simulink library "outp"  (R2021b)
settings: Solver=VariableStepAuto  StartTime=0.0  StopTime=10.0  RelTol=1e-3
undefined symbols (not defined in the file or in its folder): ENUM_PMMMODE_CHARGE, ENUM_PMMMODE_IDLE, ENUM_PMMMODE_INITIALIZE, ENUM_PMMMODE_POWERDOWN, ENUM_PMMMODE_SLEEP, Left, outp, slcm, TRUE
libraries: FVT_lib x1097, hcu_lib x4, simulink x1
(part 2 of 11)

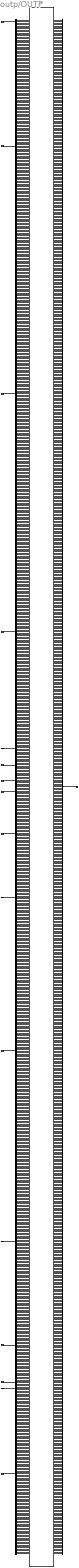
== system outp/OUTP ==
  BACC_outputs : Inport  OutDataTypeStr=Bus: BACC_outputs
  BAPM_outputs : Inport  Port=2  OutDataTypeStr=Bus: BAPM_outputs
  BBCM_outputs : Inport  Port=3  OutDataTypeStr=Bus: BBCM_outputs
  BDDM_outputs : Inport  Port=4  OutDataTypeStr=Bus: BDDM_outputs
  BDHP_outputs : Inport  Port=5  OutDataTypeStr=Bus: BDHP_outputs
  BDKC_outputs : Inport  Port=6  OutDataTypeStr=Bus: BDKC_outputs
  BDSC_outputs : Inport  Port=7  OutDataTypeStr=Bus: BDSC_outputs
  BNMM_outputs : Inport  Port=8  OutDataTypeStr=Bus: BNMM_outputs
  BPMM_outputs : Inport  Port=9  OutDataTypeStr=Bus: BPMM_outputs
  BSYS_outputs : Inport  Port=10  OutDataTypeStr=Bus: BSYS_outputs
  BTHC_outputs : Inport  Port=11  OutDataTypeStr=Bus: BTHC_outputs
  BTPM_outputs : Inport  Port=12  OutDataTypeStr=Bus: BTPM_outputs
  BTQD_outputs : Inport  Port=13  OutDataTypeStr=Bus: BTQD_outputs
  BTQR_outputs : Inport  Port=14  OutDataTypeStr=Bus: BTQR_outputs
  BV2L_outputs : Inport  Port=15  OutDataTypeStr=Bus: BV2L_outputs
  BVMC_outputs : Inport  Port=16  OutDataTypeStr=Bus: BVMC_outputs
  trig_OUTP : TriggerPort  TriggerType=function-call  VariantControl=(inherit)
  bus_creator : BusCreator  Inputs=1097
  bus_selector1 : BusSelector  OutputSignals=VACC_HVTHCMSysAvail_enum,VACC_LVBattVoltSta_enum,VACC_VehHVPwrAvail4THCM_W
  bus_selector10 : BusSelector  OutputSignals=VSYS_HWVer1_cnt,VSYS_HWVer2_cnt,VSYS_HWVer3_cnt,VSYS_CarModel1_cnt,VSYS_CarModel2_cnt,VSYS_CarModel3_cnt,VSYS_ECU1_cnt,VSYS_ECU2_cnt,VSYS_Major1_cnt,VSYS_Major2_cnt,VSYS_Minor1_cnt,VSYS_Minor2_cnt,VSYS_Patch1_cnt,VSYS_Patch2_cnt,VSYS_Country1_cnt,VSYS_Country2_cnt,VSYS_Variation_cnt,VSYS_Dash1_cnt,VSYS_Change1_cnt,VSYS_Change2_cnt,VSYS_Dash2_cnt,VSYS_SHA1_cnt,VSYS_SHA2_cnt,VSYS_SHA3_cnt,VSYS_SHA4_cnt,VSYS_SHA5_cnt,VSYS_SHA6_cnt,VSYS_SHA7_cnt,VSYS_SHA8_cnt,VSYS_NvWriteReqRisingEdge_flg,VSYS_FdcSlpReqRisingEdge_flg,VSYS_FdcSlpTime_sec,VSYS_PmicBootReason_enum,VSYS_WisrBootReason_raw32,VSYS_AcoreRebootCmdACK_flg,VSYS_CurrentNmState_enum,VSYS_ECUGen1_cnt,VSYS_ECUGen2_cnt,VSYS_PmicBootPath_raw32,VSYS_DrivingMode_cnt,VSYS_ModelYear_cnt,VSYS_Var4_cnt,VSYS_Var5_cnt
  bus_selector11 : BusSelector  OutputSignals=VTHC_FDCompCmd_rpm,VTHC_FDSOV1Cmd_flg,VTHC_FDSOV2Cmd_flg,VTHC_FDSOV3Cmd_flg,VTHC_FDEXV1Cmd_step,VTHC_FDEXV2Cmd_step,VTHC_FDSOTXVCmd_flg,VTHC_FDFWVCmd_flg,VTHC_FDTWVCmd_pct,VTHC_FDFrWPTCHeatPwrCmd_W,VTHC_CoolgFanActDuty_pct,VTHC_FDAGSCmd_enum,VTHC_FDEWP1Cmd_enum,VTHC_FDEWP2Cmd_enum,VTHC_FDEWP3Cmd_enum,VTHC_FDFrLeAPTCHeatPwrCmd_W,VTHC_FDFrRiAPTCHeatPwrCmd_W,VTHC_FDRrAPTCHeatPwrCmd_W,VTHC_FDBlowerCmd_pct,VTHC_BatteryMode_enum,VTHC_EDriveMode_enum,VTHC_CabinMode_enum,VTHC_CCUACLampSts_flg,VTHC_CCUAutoLampSts_flg,VTHC_CCUACMaxLampSts_flg,VTHC_CCUSyncLampSts_flg,VTHC_sigAirIntenZon1St_enum,VTHC_sigWindDirZon1St_enum,VTHC_sigRecircSt_flg,VTHC_sigSetTempZon1St_C,VTHC_sigSetTempZon2St_C,VTHC_sigClntTHvBattOut_C,VTHC_sigCbnSolarLeft_W,VTHC_sigClntTHvBattIn_C,VTHC_sigCbnSolarRight_W,VTHC_sigAmbAirT_C,VTHC_sigCbnAirT_C,VTHC_ACSubMode_enum,VTHC_FDRecyAutoCmd_enum,VTHC_ACModeMem_enum,VTHC_Face_flg,VTHC_Foot_flg,VTHC_Frost_flg,VTHC_FaceM_flg,VTHC_FootM_flg,VTHC_CCUSyncSts_flg,VTHC_RecAutoFlg_flg,VTHC_AirIntenZone1M_enum,VTHC_fdefog_flg,VTHC_sigSetTempZon2StM_C,VTHC_sigDfrstSt_flg,VTHC_FDCTHCAirIntZ3Sta_enum,VTHC_FDCTHCLEVentModeSta_enum,VTHC_FDCTHCREVentModeSta_enum,VTHC_FDCTHCLEVentZSta_enum,VTHC_FDCTHCCLEVentZSta_enum,VTHC_FDCTHCREVentZSta_enum,VTHC_FDCTHCCREVentZSta_enum,VTHC_FDCTHCLEVentYSta_enum,VTHC_FDCTHCLVentENSta_flg,VTHC_FDCTHCCLEVentYSta_enum,VTHC_FDCTHCCLVentENSta_flg,VTHC_FDCTHCREVentYSta_enum,VTHC_FDCTHCRVentENSta_flg,VTHC_FDCTHCCREVentYSta_enum,VTHC_FDCTHCCRVentENSta_flg,VTHC_FDCTHCMAPTCForceOFFSta_flg,VTHC_FDCFGSAirIntSta_enum,VTHC_FDCFGSChSta_enum,VTHC_FDCFGSAirIntCmd_enum,VTHC_FDCFGSFuncSta_enum,VTHC_FDCFGSChCmd_enum,VTHC_FDCFGSIONSWSta_flg,VTHC_FDCFGSIONCmd_flg,VTHC_FDCTHCMPreWPTCHeatSta_enum,VTHC_EWPBUflag1_flg,VTHC_EWPBUflag2_flg,VTHC_EWPBUflag3_flg,VTHC_FaceMSet_enum,VTHC_FootMSet_enum,VTHC_fdefogSet_enum,VTHC_CCUSyncStsSet_enum,VTHC_sigRecircStSet_enum,VTHC_RecyAutoSet_enum,VTHC_AirIntenZone1MSet1_enum,VTHC_AirIntenZone1MSet2_enum,VTHC_AirIntenZone1MSet3_enum,VTHC_AirIntenZone1MSet4_enum,VTHC_AirIntenZone1MSet5_enum,VTHC_AirIntenZone1MSet7_enum,VTHC_AirIntenZone3MSet1_enum,VTHC_AirIntenZone3MSet2_enum,VTHC_AirIntenZone3MSet3_enum,VTHC_AirIntenZone3MSet4_enum,VTHC_AirIntenZone3MSet5_enum,VTHC_AirIntenZone3MSet7_enum,VTHC_IONSWStaSet_enum,VTHC_FDCFGSChStaSet123_enum,VTHC_FDCFGSChStaSet457_enum,VTHC_FDCFGSAirIntStaSet123_enum,VTHC_FDCFGSAirIntStaSet457_enum,VTHC_LVentENSet_enum,VTHC_CLVentENSet_enum,VTHC_RVentENSet_enum,VTHC_CRVentENSet_enum,VTHC_LEVentModeStaSet123_enum,VTHC_LEVentModeStaSet457_enum,VTHC_REVentModeStaSet123_enum,VTHC_REVentModeStaSet457_enum,VTHC_FDCTHCLEVentZStaSet1_enum,VTHC_FDCTHCLEVentZStaSet2_enum,VTHC_FDCTHCLEVentZStaSet3_enum,VTHC_FDCTHCLEVentZStaSet4_enum,VTHC_FDCTHCLEVentZStaSet5_enum,VTHC_FDCTHCLEVentZStaSet7_enum,VTHC_FDCTHCCLEVentZStaSet1_enum,VTHC_FDCTHCCLEVentZStaSet2_enum,VTHC_FDCTHCCLEVentZStaSet3_enum,VTHC_FDCTHCCLEVentZStaSet4_enum,VTHC_FDCTHCCLEVentZStaSet5_enum,VTHC_FDCTHCCLEVentZStaSet7_enum,VTHC_FDCTHCREVentZStaSet1_enum,VTHC_FDCTHCREVentZStaSet2_enum,VTHC_FDCTHCREVentZStaSet3_enum,VTHC_FDCTHCREVentZStaSet4_enum,VTHC_FDCTHCREVentZStaSet5_enum,VTHC_FDCTHCREVentZStaSet7_enum,VTHC_FDCTHCCREVentZStaSet1_enum,VTHC_FDCTHCCREVentZStaSet2_enum,VTHC_FDCTHCCREVentZStaSet3_enum,VTHC_FDCTHCCREVentZStaSet4_enum,VTHC_FDCTHCCREVentZStaSet5_enum,VTHC_FDCTHCCREVentZStaSet7_enum,VTHC_FDCTHCLEVentYStaSet1_enum,VTHC_FDCTHCLEVentYStaSet2_enum,VTHC_FDCTHCLEVentYStaSet3_enum,VTHC_FDCTHCLEVentYStaSet4_enum,VTHC_FDCTHCLEVentYStaSet5_enum,VTHC_FDCTHCLEVentYStaSet7_enum,VTHC_FDCTHCCLEVentYStaSet1_enum,VTHC_FDCTHCCLEVentYStaSet2_enum,VTHC_FDCTHCCLEVentYStaSet3_enum,VTHC_FDCTHCCLEVentYStaSet4_enum,VTHC_FDCTHCCLEVentYStaSet5_enum,VTHC_FDCTHCCLEVentYStaSet7_enum,VTHC_FDCTHCREVentYStaSet1_enum,VTHC_FDCTHCREVentYStaSet2_enum,VTHC_FDCTHCREVentYStaSet3_enum,VTHC_FDCTHCREVentYStaSet4_enum,VTHC_FDCTHCREVentYStaSet5_enum,VTHC_FDCTHCREVentYStaSet7_enum,VTHC_FDCTHCCREVentYStaSet1_enum,VTHC_FDCTHCCREVentYStaSet2_enum,VTHC_FDCTHCCREVentYStaSet3_enum,VTHC_FDCTHCCREVentYStaSet4_enum,VTHC_FDCTHCCREVentYStaSet5_enum,VTHC_FDCTHCCREVentYStaSet7_enum,VTHC_SettempZon1Set1_enum,VTHC_SettempZon1Set2_enum,VTHC_SettempZon1Set3_enum,VTHC_SettempZon1Set4_enum,VTHC_SettempZon1Set5_enum,VTHC_SettempZon1Set7_enum,VTHC_ACModeSet123_enum,VTHC_ACModeSet457_enum,VTHC_FACESet_enum,VTHC_FOOTSet_enum,VTHC_FrostSet_enum,VTHC_LVentEN_flg,VTHC_CLVentEN_flg,VTHC_RVentEN_flg,VTHC_CRVentEN_flg,VTHC_FDCFGSLearnCmd_enum,VTHC_FDCFGSFuncSta_flg,VTHC_THSysErrlampReq_flg,VTHC_sigCbnPTCPwrAct_W
  bus_selector12 : BusSelector  OutputSignals=VTPM_LFBatWarn_flg,VTPM_RFBatWarn_flg,VTPM_LRBatWarn_flg,VTPM_RRBatWarn_flg,VTPM_LFWheelPress_raw8,VTPM_RFWheelPress_raw8,VTPM_LRWheelPress_raw8,VTPM_RRWheelPress_raw8,VTPM_LFWheelTemp_C,VTPM_RFWheelTemp_C,VTPM_LRWheelTemp_C,VTPM_RRWheelTemp_C,VTPM_LFSensorFail_flg,VTPM_RFSensorFail_flg,VTPM_LRSensorFail_flg,VTPM_RRSensorFail_flg,VTPM_LFWheelDebug_flg,VTPM_LRWheelDebug_flg,VTPM_RFWheelDebug_flg,VTPM_RRWheelDebug_flg,VTPM_TPMSResButtAllow_flg,VTPM_TPMSCaliButtAllow_flg,VTPM_LFPressIndi_enum,VTPM_RFPressIndi_enum,VTPM_LRPressIndi_enum,VTPM_RRPressIndi_enum,VTPM_TPMSWarnIndi_enum,VTPM_LFWheelTmpIndi_flg,VTPM_RFWheelTmpIndi_flg,VTPM_LRWheelTmpIndi_flg,VTPM_RRWheelTmpIndi_flg,VTPM_LFWheelPSW_raw8,VTPM_LRWheelPSW_raw8,VTPM_RFWheelPSW_raw8,VTPM_RRWheelPSW_raw8,VTPM_CWheelTips_enum,VTPM_AutoLTips_enum,VTPM_LFSensorMode_flg,VTPM_RFSensorMode_flg,VTPM_LRSensorMode_flg,VTPM_RRSensorMode_flg,VTPM_S1ID_raw32,VTPM_S2ID_raw32,VTPM_S3ID_raw32,VTPM_S4ID_raw32,VTPM_S1L_enum,VTPM_S2L_enum,VTPM_S3L_enum,VTPM_S4L_enum,VTPM_ALFin_flg,VTPM_LFP20_raw8,VTPM_RFP20_raw8,VTPM_LRP20_raw8,VTPM_RRP20_raw8,VTPM_FAT_flg,VTPM_IDin_raw32,VTPM_S1WheelDebugALTU_pct,VTPM_S2WheelDebugALTU_pct,VTPM_S3WheelDebugALTU_pct,VTPM_S4WheelDebugALTU_pct,VTPM_ID1messageALTU_raw8,VTPM_ID2messageALTU_raw8,VTPM_ID3messageALTU_raw8,VTPM_ID4messageALTU_raw8,VTPM_Chkfin_flg,VTPM_SetIDLoc_flg,VTPM_TPMSStorge_flg,VTPM_ChkStorge_flg,VTPM_TPMSResButt_flg,VTPM_LFPindi_enum,VTPM_RFPind_enum,VTPM_LRPindi_enum,VTPM_RRPindi_enum,VTPM_WriteChkLFID_raw,VTPM_WriteChkRFID_raw,VTPM_WriteChkLRID_raw,VTPM_WriteChkRRID_raw,VTPM_WriteChkfinLFID_raw,VTPM_WriteChkfinRFID_raw,VTPM_WriteChkfinLRID_raw,VTPM_WriteChkfinRRID_raw,VTPM_Flashchkdatavalid_enum,VTPM_Flashdatavalid_enum,VTPM_unlearnSfali_flg,VTPM_unlearnSfailvalid_enum,VTPM_Prepresstempvalid_enum,VTPM_FlashS1ID_raw,VTPM_FlashS2ID_raw,VTPM_FlashS3ID_raw,VTPM_FlashS4ID_raw,VTPM_FlashIDvalid_enum,VTPM_WritingCnt_enum,VTPM_TPMSTLCmd_flg,VTPM_LProgress_enum,VTPM_TPMSSensorIDRegStart_flg,VTPM_ModelVersion_raw,VTPM_ModelVersionChksum_raw
  bus_selector13 : BusSelector  OutputSignals=VTQD_ParkRequest_flg,VTQD_TqSourceFr_enum,VTQD_TqSourceRr_enum,VTQD_FrEDUAvailBrkRgnTq_Nm,VTQD_RrEDUAvailBrkRgnTq_Nm,VTQD_EVDriveMode_enum,VTQD_ShiftGearPosn_enum,VTQD_PButtonSta_enum,VTQD_FrActvDmpDisabReq_flg,VTQD_RrActvDmpDisabReq_flg,VTQD_FrRgnDecrSta_flg,VTQD_RrRgnDecrSta_flg,VTQD_DriverWhlTqDemFr_Nm,VTQD_DriverWhlTqDemRr_Nm,VTQD_FrEDUActTq_Nm,VTQD_RrEDUActTq_Nm,VTQD_FrEDURolRgnTq_Nm,VTQD_RrEDURolRgnTq_Nm,VTQD_FrEDUSpd_rpm,VTQD_RrEDUSpd_rpm,VTQD_FrEDUSpdValid_flg,VTQD_FrEDUAvailBrkRgnTqV_flg,VTQD_RrEDUSpdValid_flg,VTQD_RrEDUAvailBrkRgnTqV_flg,VTQD_RgnAbnorSta_flg,VTQD_PTCSPermSta_flg,VTQD_FrRgnPermSta_flg,VTQD_RrRgnPermSta_flg,VTQD_FrIdcMin_A,VTQD_FrIdcMax_A,VTQD_FrUdcMin_V,VTQD_FrUdcMax_V,VTQD_RrIdcMin_A,VTQD_RrIdcMax_A,VTQD_RrUdcMin_V,VTQD_RrUdcMax_V,VTQD_ReBrakeLPReq_flg,VTQD_CreepON_flg,VTQD_EquivAccPedalSWSta_flg,VTQD_DriveProtEn_flg,VTQD_ActParkRequest_flg,VTQD_IVIPwrLockSta_enum,VTQD_OPDHoldLamp_flg,VTQD_SaveRegenMode_enum,VTQD_FDCVCURegenMode_enum,VTQD_SpdCtrlMode_enum,VTQD_SpdCtrlSta_flg,VTQD_SetSpd_kph,VTQD_VehActSpd_kph,VTQD_RegenLimIndSta_flg,VTQD_SetSpdLimWarn_flg
  bus_selector14 : BusSelector  OutputSignals=VTQR_FrTMTqReq_Nm,VTQR_RrTMTqReq_Nm
  bus_selector15 : BusSelector  OutputSignals=VV2L_ReqOBCV2LEna_enum,VV2L_ReqV2LIVIPopup_enum,VV2L_ReqV2LIVIDisChrg_enum,VV2L_ReqOBCExtrV2LEna_enum,VV2L_ReqOBCIntrV2LEna_enum,VV2L_HVPO120VGrpALDSt_enum,VV2L_HVPO120VGrpBLDSt_enum
  bus_selector16 : BusSelector  OutputSignals=VVMC_FeatSetSpdFinal_raw32,VVMC_VehicleSpeed_mph,VVMC_VehicleSpeed_kph,VVMC_MeterIndSpeed_raw32,VVMC_VMCAEBCtrlAvail_flg,VVMC_VMCACCCtrlAvail_flg,VVMC_VMCCCCtrlAvail_flg,VVMC_VMCMSACtrlAvail_flg,VVMC_FeatArbitrSta_enum,VVMC_FeatReqSpd_kph,VVMC_JerkPCT_pct,VVMC_LimitPCT_pct,VVMC_FrontRearSlipRatioCtrl_flg,VVMC_RearWhlSlipRatioCtrl_flg,VVMC_SingleWhlSlipRatioCtrl_flg,VVMC_LatAccCtrl_flg,VVMC_SafetyCtrl_flg,VVMC_SPD2ACCAct_flg,VVMC_AccCalcuPID_mps2,VVMC_ISOAccLimit_mps2,VVMC_ISODecLimit_mps2,VVMC_ISOJerkLimit_mps3,VVMC_ACCRequiredAccel_mps2,VVMC_DISCReqAcc_mps2,VVMC_FeatArbitrFinal_enum,VVMC_ActACCRequiredAccel_mps2,VVMC_LateralCtrl_flg,VVMC_ADASLKASta_enum,VVMC_LKAStrToqReq_Nm,VVMC_LKATOIFault_flg,VVMC_LKATOIAct_enum,VVMC_ADASAEBReq_enum,VVMC_ADASFaultSta_flg,VVMC_AEBVehHoldReq_flg,VVMC_ACCVehHoldReq_flg,VVMC_ADASDBSReq_enum,VVMC_ADASACCSta_enum,VVMC_ACCObjDist_m,VVMC_ACCObjRelSpd_mps,VVMC_TimeGapLevel_enum,VVMC_ACCJerkUpperLimit_mps3,VVMC_ACCComfortBandUpper_mps2,VVMC_ACCJerkLowerLimit_mps3,VVMC_ACCComfortBandLower_mps2,VVMC_ADASVehSpdLim_raw32,VVMC_ADASShftPosnReqA_flg,VVMC_ADASShftPosnReq_enum,VVMC_ADASForceIdle_flg,VVMC_HazardWarningReq_flg,VVMC_RightTurnLightReq_flg,VVMC_LeftTurnLightReq_flg,VVMC_ADASFCWSta_enum,VVMC_ADASLDWSta_enum,VVMC_ADASFltWrnReq_flg,VVMC_ACCObjDstLvl_enum,VVMC_ForceLowBeam_enum,VVMC_ACCTakeoverReq_flg,VVMC_ADASWarningMsg_enum,VVMC_ADASCAMSpdLim_enum,VVMC_TargetType_enum,VVMC_ADASSLIFSpdLim_enum,VVMC_LKAHODDisplayWarning_flg,VVMC_LKAHODSoundWarning_flg,VVMC_ADASLFCSta_enum,VVMC_ADASLaneModeL_enum,VVMC_ADASLaneModeR_enum,VVMC_ADASSLIFSta_enum,VVMC_ADASISASta_enum,VVMC_ADASLDWMute_flg,VVMC_ADASFCWMute_flg,VVMC_ADASLFCHandsOffWarning_enum,VVMC_LVDADisabled_flg,VVMC_LVDAMuteSta_enum,VVMC_LVDAFailinfo_flg,VVMC_LVDAWarning_flg,VVMC_LVDAACCStatusInformation_flg,VVMC_ADASLFCWarnSound_enum,VVMC_FCMACCmode_enum,VVMC_ADASLanetypeR_enum,VVMC_ADASLanetypeL_enum,VVMC_ADASLanecurveL_raw32,VVMC_ADASLanecurveR_raw32,VVMC_ADASAEBSta_enum,VVMC_FCMLDWRequest_enum,VVMC_FCMLDWFault_flg,VVMC_ACCCtrlAvail_flg,VVMC_ACCPedalOvrd_flg,VVMC_TimeGapCalcu_s,VVMC_CCCtrlSta_enum,VVMC_MSACtrlSta_enum,VVMC_APSCtrlAvail_flg,VVMC_APSActive_flg,VVMC_APSStaSys_enum,VVMC_APSDecReqA_flg,VVMC_APSDecReq_mps2,VVMC_APSReq_enum,VVMC_LongAcc_Gps,VVMC_CCMSASpdWar_flg,VVMC_IMUEnaCmd_flg,VVMC_CAASCtrlAvail_flg,VVMC_CAASActive_flg,VVMC_ExtraMSACtrlSta_enum,VVMC_CalibratedAccX_G,VVMC_CalibratedAccY_G,VVMC_CalibratedAccZ_G,VVMC_CalibratedGyroX_Dps,VVMC_CalibratedGyroY_Dps,VVMC_CalibratedGyroZ_Dps,VVMC_FDCVMCAPSVRqEPSCtrl_flg,VVMC_FDCVMCAPSAngleTarget_deg,VVMC_FDCVMCAPSRqEPSCtrl_flg,VVMC_FDCVMCAngCtrlTqWtGn_pct,VVMC_FDCVMCDrInpTqBstAct_flg,VVMC_FDCVMCMaxAngCtrlOutTqLim_Nm,VVMC_FDCVMCDrInpTqBstGn_pct
  bus_selector2 : BusSelector  OutputSignals=VAPM_VehSpeed_kph,VAPM_VehSpeedTimeOut_flg,VAPM_FSOffSw_enum,VAPM_FSOffSwTimeOut_flg,VAPM_ChrgPlugSta_enum,VAPM_PASDRMR_cm,VAPM_PASDRML_cm,VAPM_PASDRCR_cm,VAPM_PASDRCL_cm,VAPM_PASDFMR_cm,VAPM_PASDFML_cm,VAPM_PASDFCR_cm,VAPM_PASDFCL_cm,VAPM_APSDRLR_cm,VAPM_APSDRLL_cm,VAPM_APSDFLR_cm,VAPM_APSDFLL_cm,VAPM_PASAFCL_enum,VAPM_PASARMR_enum,VAPM_PASARML_enum,VAPM_PASARCR_enum,VAPM_PASARCL_enum,VAPM_PASAFMR_enum,VAPM_PASAFML_enum,VAPM_PASAFCR_enum,VAPM_USSStaRMR_flg,VAPM_USSStaRML_flg,VAPM_USSStaRLR_flg,VAPM_USSStaRLL_flg,VAPM_USSStaRCR_flg,VAPM_USSStaRCL_flg,VAPM_USSStaFMR_flg,VAPM_USSStaFML_flg,VAPM_USSStaFLR_flg,VAPM_USSStaFLL_flg,VAPM_USSStaFCR_flg,VAPM_USSStaFCL_flg,VAPM_Chime_enum,VAPM_SNSRLayout_enum,VAPM_StaFSya_flg,VAPM_ModOperation_enum,VAPM_BrkPedalPos_pct,VAPM_BrkPedalPosTimeOut_flg,VAPM_LFRawWhlSpeed_kph,VAPM_LFRawWhlSpeedTimeOut_flg,VAPM_RFRawWhlSpeed_kph,VAPM_RFRawWhlSpeedTimeOut_flg,VAPM_LRRawWhlSpeed_kph,VAPM_LRRawWhlSpeedTimeOut_flg,VAPM_RRRawWhlSpeed_kph,VAPM_RRRawWhlSpeedTimeOut_flg,VAPM_LFRawWhlSpeedV_flg,VAPM_LFRawWhlSpeedVTimeOut_flg,VAPM_RFRawWhlSpeedV_flg,VAPM_RFRawWhlSpeedVTimeOut_flg,VAPM_LRRawWhlSpeedV_flg,VAPM_LRRawWhlSpeedVTimeOut_flg,VAPM_RRRawWhlSpeedV_flg,VAPM_RRRawWhlSpeedVTimeOut_flg,VAPM_LFWhlRotDir_enum,VAPM_LFWhlRotDirTimeOut_flg,VAPM_RFWhlRotDir_enum,VAPM_RFWhlRotDirTimeOut_flg,VAPM_LRWhlRotDir_enum,VAPM_LRWhlRotDirTimeOut_flg,VAPM_RRWhlRotDir_enum,VAPM_RRWhlRotDirTimeOut_flg,VAPM_LFPulseCountV_flg,VAPM_LFPulseCountVTimeOut_flg,VAPM_RFPulseCountV_flg,VAPM_RFPulseCountVTimeOut_flg,VAPM_LRPulseCountV_flg,VAPM_LRPulseCountVTimeOut_flg,VAPM_RRPulseCountV_flg,VAPM_RRPulseCountVTimeOut_flg,VAPM_LFPulseCount_enum,VAPM_LFPulseCountTimeOut_flg,VAPM_RFPulseCount_enum,VAPM_RFPulseCountTimeOut_flg,VAPM_LRPulseCount_enum,VAPM_LRPulseCountTimeOut_flg,VAPM_RRPulseCount_enum,VAPM_RRPulseCountTimeOut_flg,VAPM_ShifterHandleCmd_enum,VAPM_ShifterHandleCmdTimeOut_flg,VAPM_DriIntend_enum,VAPM_DriIntendTimeOut_flg,VAPM_EPSAOIControl_enum,VAPM_EPSAOIControlTimeOut_flg,VAPM_SASAngle_Deg,VAPM_SASAngleTimeOut_flg,VAPM_SASSpeed_degps,VAPM_SASSpeedTimeOut_flg,VAPM_SASSpeedValid_flg,VAPM_SASSpeedValidTimeOut_flg,VAPM_SASCAL_flg,VAPM_SASCALTimeOut_flg,VAPM_SASV_flg,VAPM_SASVTimeOut_flg,VAPM_GRADE_Deg,VAPM_GRADETimeOut_flg,VAPM_YawRate_degps,VAPM_YawRateTimeOut_flg,VAPM_LatAccel_Gps,VAPM_LatAccelTimeOut_flg,VAPM_LongAccel_Gps,VAPM_LongAccelTimeOut_flg,VAPM_MCPressure_bar,VAPM_MCPressureTimeOut_flg,VAPM_YawRateV_flg,VAPM_YawRateVTimeOut_flg,VAPM_LatAccelV_flg,VAPM_LatAccelVTimeOut_flg,VAPM_LongAccelV_flg,VAPM_LongAccelVTimeOut_flg,VAPM_MCPressureV_bar,VAPM_MCPressureVTimeOut_flg,VAPM_BrkSwSta_flg,VAPM_BrkSwStaTimeOut_flg,VAPM_BrkSwV_flg,VAPM_BrkSwVTimeOut_flg,VAPM_ESCStandstill_flg,VAPM_ESCStandstillTimeOut_flg,VAPM_ESCAPSSta_enum,VAPM_ESCAPSStaTimeOut_flg,VAPM_EPBExtReleaseAvail_flg,VAPM_EPBExtReleaseAvailTimeOut_flg,VAPM_EPBExtApplyAvail_flg,VAPM_EPBExtApplyAvailTimeOut_flg,VAPM_EPBErrSta_enum,VAPM_EPBErrStaTimeOut_flg,VAPM_EPBSta_enum,VAPM_EPBStaTimeOut_flg,VAPM_AVMparkingcancel_enum,VAPM_AVMparkingcancelTimeOut_flg,VAPM_AVMparkingexcute_enum,VAPM_AVMparkingexcuteTimeOut_flg,VAPM_AVMParkingmode_enum,VAPM_AVMParkingmodeTimeOut_flg,VAPM_AVMErrSTA_flg,VAPM_AVMErrSTATimeOut_flg,VAPM_IVIStatus_flg,VAPM_IVIStatusTimeOut_flg,VAPM_CAASSw_enum,VAPM_CAASSwTimeOut_flg,VAPM_IVIScreen_enum,VAPM_IVIScreenTimeOut_flg,VAPM_ABSActive_flg,VAPM_ABSActiveTimeOut_flg,VAPM_TCSActive_flg,VAPM_TCSActiveTimeOut_flg,VAPM_DriverSeatBeltCmd_flg,VAPM_DriverSeatBeltCmdTimeOut_flg,VAPM_APSProgressPCT_pct,VAPM_APSRQDisplay_enum,VAPM_APSSWVer_enum,VAPM_APSHWVer_enum,VAPM_APSExitCondition_enum,VAPM_APSAngleTarget_Deg,VAPM_APSVRqEPASCtrl_flg,VAPM_APSRqEPASCtrl_flg,VAPM_CAASSta_enum,VAPM_DKCPDkeyAreaRAPSSta_enum,VAPM_DKCParkingModeCmd_enum,VAPM_PUIDLowPower_flg,VAPM_CAASVMCReqA_flg,VAPM_APSShiftPosnReq_enum,VAPM_APSSpeedCMD_kph,VAPM_APSVMCReqA_flg,VAPM_RAPSBCMLamp_enum,VAPM_RAPSBCMLockReq_flg,VAPM_APSPwrReq_enum,VAPM_RAPSErrWarnSta_enum,VAPM_RAPSErrLv1_flg,VAPM_IVIUserTakeOverAPSSta_flg
  bus_selector3 : BusSelector  OutputSignals=VBCM_AntitheftSta_enum,VBCM_TailgateRemote_enum,VBCM_HornCtrl_flg,VBCM_AllDoorSW_flg,VBCM_BCMDoorLockSta_flg,VBCM_AntitheftSeatFlod_flg,VBCM_HoodSW_flg,VBCM_TailgateSW_flg,VBCM_DrDoorSW_flg,VBCM_PsDoorSW_flg,VBCM_RLDoorSW_flg,VBCM_RRDoorSW_flg,VBCM_LockSetting_flg,VBCM_FrChargingDoorCtrl_enum,VBCM_RrChargingDoorCtrl_enum,VBCM_CrashDetd_flg,VBCM_CTDCtrl_enum,VBCM_DoorLockIND_flg,VBCM_CTDLockSW_flg,VBCM_Dimmer_pct,VBCM_DimmerEN_flg,VBCM_PosLamp_flg,VBCM_LBeam_flg,VBCM_HBeam_flg,VBCM_RrFogLamp_flg,VBCM_BrakeLamp_flg,VBCM_ReverseLamp_flg,VBCM_LDRL_flg,VBCM_RDRL_flg,VBCM_LBSD_flg,VBCM_RBSD_flg,VBCM_HazardSW_flg,VBCM_LTurnLP_flg,VBCM_RTurnLP_flg,VBCM_BCMBuzzerReq_flg,VBCM_MirrorCtrl_enum,VBCM_MirrorDefog_flg,VBCM_RrDefog_flg,VBCM_RoomLampH_flg,VBCM_RoomLampL_flg,VBCM_TrunkRel_flg,VBCM_TailgateHDSW_flg,VBCM_FrWiperL_flg,VBCM_FrWiperH_flg,VBCM_RrWiper_flg,VBCM_WasherCtrl_enum,VBCM_WiperFixMode_flg,VBCM_AmbLightBreath1_enum,VBCM_AmbLightBreath2_enum,VBCM_AmbLightBreath3_enum,VBCM_AmbLightBreath4_enum,VBCM_AmbLightBreath5_enum,VBCM_AmbLightBreath6_enum,VBCM_AmbLightBrightness1_enum,VBCM_AmbLightBrightness2_enum,VBCM_AmbLightBrightness3_enum,VBCM_AmbLightBrightness4_enum,VBCM_AmbLightBrightness5_enum,VBCM_AmbLightBrightness6_enum,VBCM_AmbLightColor1_enum,VBCM_AmbLightColor2_enum,VBCM_AmbLightColor3_enum,VBCM_AmbLightColor4_enum,VBCM_AmbLightColor5_enum,VBCM_AmbLightColor6_enum,VBCM_LampPwr_flg,VBCM_SPTGDet_flg,VBCM_APSOpenPTG_flg,VBCM_FollowMe_flg,VBCM_IVIRST_flg,VBCM_CountAlarm_enum,VBCM_MFSWTri_flg,VBCM_MirrorFlodPos_flg,VBCM_FuelDoorPos_flg,VBCM_MFRDNBrightReq_pct,VBCM_PTGInnerSW2_enum,VBCM_DrvWdwCtrlCmd_pct,VBCM_PasWdwCtrlCmd_pct,VBCM_DrRWdwCtrlCmd_pct,VBCM_PsRWdwCtrlCmd_pct,VBCM_APMDoorControlSta_flg,VBCM_AmbFunEN_flg,VBCM_AmbWelEN_flg,VBCM_AmbDimEN_flg,VBCM_AmbLinkDriSta_flg,VBCM_AmbPwrWarnEN_flg,VBCM_AmbODAEN_flg,VBCM_AmbColorSta_enum,VBCM_AmbBrightSta_enum,VBCM_LockAlarm_enum,VBCM_ATCtrl_enum,VBCM_fUnlockSingle_flg,VBCM_UserNow_enum,VBCM_AmbFunENFlash_enum,VBCM_AmbWelENFlash_enum,VBCM_AmbDimENFlash_enum,VBCM_AmbLinkDriStaFlash_enum,VBCM_AmbPwrWarnENFlash_enum,VBCM_AmbODAENFlash_enum,VBCM_AmbColorSta1_enum,VBCM_AmbColorSta2_enum,VBCM_AmbColorSta3_enum,VBCM_AmbColorSta4_enum,VBCM_AmbColorSta5_enum,VBCM_AmbColorSta7_enum,VBCM_AmbBrightnessSta1_enum,VBCM_AmbBrightnessSta2_enum,VBCM_AmbBrightnessSta3_enum,VBCM_AmbBrightnessSta4_enum,VBCM_AmbBrightnessSta5_enum,VBCM_AmbBrightnessSta7_enum,VBCM_HazardIND_flg,VBCM_DimSwSta_flg,VBCM_PassSWSta_flg,VBCM_FWipSwSta_enum,VBCM_FWasSwSta_enum,VBCM_TurnSwSta_enum,VBCM_TurnSwTSetSta_enum,VBCM_SPTGENFun_flg,VBCM_SPTGENFunMem_enum,VBCM_OutMode_enum,VBCM_TurnSwTimeSetSta123_enum,VBCM_TurnSwTimeSetSta457_enum,VBCM_FDLHandleLampCmd_flg,VBCM_FDRHandleLampCmd_flg,VBCM_FDHandleCmd_enum,VBCM_HBeamADB_flg,VBCM_WalkInUnLkENMem_enum,VBCM_WalkOutLkENMem_enum,VBCM_RmLpModeENMem_enum,VBCM_LockSettingStaMem_enum,VBCM_FollowMeENMem_enum,VBCM_WalkInUnLkENFunSta_flg,VBCM_WalkOutLkENFunSta_flg,VBCM_RmLpModeENFunSta_flg,VBCM_FollowMeENFunSta_flg,VBCM_HoodRelCmd_flg,VBCM_WelcomeLight_enum,VBCM_PTGOpenHeightSta_enum,VBCM_UserHeightSet_cnt,VBCM_PTGUserHeight1_cnt,VBCM_PTGUserHeight2_cnt,VBCM_PTGUserHeight3_cnt,VBCM_PTGUserHeight4_cnt,VBCM_PTGUserHeight5_cnt,VBCM_PTGUserHeight7_cnt,VBCM_PTGOpenHeight12_enum,VBCM_PTGOpenHeight34_enum,VBCM_PTGOpenHeight57_enum,VBCM_SenstivityPosnCmd_enum,VBCM_TimeGapLevelSta_enum,VBCM_ACCLevelMem12_enum,VBCM_ACCLevelMem34_enum,VBCM_ACCLevelMem57_enum,VBCM_LRightStaCmd_flg,VBCM_LLeftStaCmd_flg,VBCM_AutoLockSta_flg,VBCM_AutoLockMem_enum,VBCM_AutoUnlockSta_flg,VBCM_AutoUnlockMem_enum,VBCM_HMIKey1FuncSta_enum,VBCM_HMIKey2FuncSta_enum,VBCM_HMIKey3FuncSta_enum,VBCM_HMIKey4FuncSta_enum,VBCM_HMIKey5FuncSta_enum,VBCM_HMIKey6FuncSta_enum,VBCM_HMIKey7FuncSta_enum,VBCM_HMIKey8FuncSta_enum,VBCM_AutoWipHSpdENSta_flg,VBCM_DrvWdwReqAP_enum,VBCM_PasWdwReqAP_enum,VBCM_DrRWdwReqAP_enum,VBCM_PsRWdwReqAP_enum,VBCM_CLWinLockDrSta_flg,VBCM_CLWinLockDrStaMem_enum,VBCM_WinLFOpenedSta_pct,VBCM_WinRFOpenedSta_pct,VBCM_WinLROpenedSta_pct,VBCM_WinRROpenedSta_pct
  bus_selector4 : BusSelector  OutputSignals=VDDM_C3BMS6RCDTC_raw32,VDDM_C3BMS6CSDTC_raw32,VDDM_C3BMS6LCDTC_raw32,VDDM_C3BMS1RCDTC_raw32,VDDM_C3BMS1CSDTC_raw32,VDDM_C3BMS1LCDTC_raw32,VDDM_C3CCU1RCDTC_raw32,VDDM_C3CCU1CSDTC_raw32,VDDM_C3CCU1LCDTC_raw32,VDDM_C3CCU2RCDTC_raw32,VDDM_C3CCU2CSDTC_raw32,VDDM_C3CCU2LCDTC_raw32,VDDM_C1ABM1RCDTC_raw32,VDDM_C1ABM1CSDTC_raw32,VDDM_C1ABM1LCDTC_raw32,VDDM_Lv1ErrDTC_raw32,VDDM_Lv2ErrDTC_raw32,VDDM_Lv3ErrDTC_raw32,VDDM_Lv4ErrDTC_raw32,VDDM_BrkSWErrDTC_raw32,VDDM_BrkSWNoBacDTC_raw32,VDDM_KeyAuthDTC_raw32,VDDM_ONtoRdyDTC_raw32,VDDM_HVB4PreDTC_raw32,VDDM_MCU4PreDTC_raw32,VDDM_DCDC4PreDTC_raw32,VDDM_HVRlyCloDTC_raw32,VDDM_BMSRdyDTC_raw32,VDDM_DCDCEnaDTC_raw32,VDDM_HiLvSaChkDTC_raw32,VDDM_MidLvSaChkDTC_raw32,VDDM_MCUDisDTC_raw32,VDDM_DCDCDisDTC_raw32,VDDM_HVRlyOpDTC_raw32,VDDM_MCUActDTC_raw32,VDDM_OBC4PreDTC_raw32,VDDM_IniLVLoDTC_raw32,VDDM_LVSupLoDTC_raw32,VDDM_LVSupHiDTC_raw32,VDDM_DrStSWDTC_raw32,VDDM_FLDoorSWDTC_raw32,VDDM_RLDoorSWDTC_raw32,VDDM_FRDoorSWDTC_raw32,VDDM_RRDoorSWDTC_raw32,VDDM_HoodSWDTC_raw32,VDDM_TailgaSWDTC_raw32,VDDM_EDriveSysErrVCUErr_flg,VDDM_VehMalfunLevel_enum,VDDM_APS1SigOoRDTC_raw32,VDDM_APS2SigOoRDTC_raw32,VDDM_APSCorrErrDTC_raw32,VDDM_MCUF1NoComDTC_raw32,VDDM_MCUR1NoComDTC_raw32,VDDM_Shifter1NoComDTC_raw32,VDDM_ESC7NoComDTC_raw32,VDDM_ESC1NoComDTC_raw32,VDDM_ESC5NoComDTC_raw32,VDDM_EnterNewOperCyc_flg,VDDM_DiagHCrashDTC_raw32,VDDM_DiagFLTSDTC_raw32,VDDM_DiagFRTSDTC_raw32,VDDM_DiagRLTSDTC_raw32,VDDM_DiagRRTSDTC_raw32,VDDM_FCLUSSDTC_raw32,VDDM_FMLUSSDTC_raw32,VDDM_FMRUSSDTC_raw32,VDDM_FCRUSSDTC_raw32,VDDM_RCLUSSDTC_raw32,VDDM_RMLUSSDTC_raw32,VDDM_RMRUSSDTC_raw32,VDDM_RCRUSSDTC_raw32,VDDM_FLLUSSDTC_raw32,VDDM_FLRUSSDTC_raw32,VDDM_RLLUSSDTC_raw32,VDDM_RLRUSSDTC_raw32,VDDM_FCM2NoComDTC_raw32,VDDM_FCM2RCErrDTC_raw32,VDDM_FCM2CSErrDTC_raw32,VDDM_FCM3NoComDTC_raw32,VDDM_FCM3RCErrDTC_raw32,VDDM_FCM3CSErrDTC_raw32,VDDM_FCM4NoComDTC_raw32,VDDM_FCM4CSErrDTC_raw32,VDDM_FCM5NoComDTC_raw32,VDDM_FCM5CSErrDTC_raw32,VDDM_ZoneSCPNoComDTC_raw32,VDDM_BMSSigErrDetDTC_raw32,VDDM_FCMACCSigErrDetDTC_raw32,VDDM_FrMCUSigErrDetDTC_raw32,VDDM_RrMCUSigErrDetDTC_raw32,VDDM_CCUSigErrDetDTC_raw32,VDDM_ACCAccelCmdErrDetDTC_raw32,VDDM_ACCMalfuncDetDTC_raw32,VDDM_CCMalfuncDetDTC_raw32,VDDM_MSAMalfuncDetDTC_raw32,VDDM_ISAMalfuncDetDTC_raw32,VDDM_MCUF1RCErrDTC_raw32,VDDM_MCUR1RCErrDTC_raw32,VDDM_MCUF1CSErrDTC_raw32,VDDM_MCUR1CSErrDTC_raw32,VDDM_Shifter1RCErrDTC_raw32,VDDM_Shifter1CSErrDTC_raw32,VDDM_ESC7RCErrDTC_raw32,VDDM_ESC7CSErrDTC_raw32,VDDM_ESC1RCErrDTC_raw32,VDDM_ESC1CSErrDTC_raw32,VDDM_ESC5RCErrDTC_raw32,VDDM_ESC5CSErrDTC_raw32,VDDM_FrMCUTqErrDTC_raw32,VDDM_RrMCUTqErrDTC_raw32,VDDM_LFBatwarnDTC_raw32,VDDM_RFBatwarnDTC_raw32,VDDM_LRBatwarnDTC_raw32,VDDM_RRBatwarnDTC_raw32,VDDM_LFPressIndiDTC_raw32,VDDM_RFPressIndiDTC_raw32,VDDM_LRPressIndiDTC_raw32,VDDM_RRPressIndiDTC_raw32,VDDM_LFWheelTmpHighDTC_raw32,VDDM_RFWheelTmpHighDTC_raw32,VDDM_LRWheelTmpHighDTC_raw32,VDDM_RRWheelTmpHighDTC_raw32,VDDM_LFSensorFailDTC_raw32,VDDM_RFSensorFailDTC_raw32,VDDM_LRSensorFailDTC_raw32,VDDM_RRSensorFailDTC_raw32,VDDM_C1EPAS2LCDTC_raw32,VDDM_5vAPS1PwrErrDTC_raw32,VDDM_5vAPS2PwrErrDTC_raw32,VDDM_EPBLockTODTC_raw32,VDDM_EPBUnlockTODTC_raw32,VDDM_LimpHomeActTmp_flg,VDDM_DTCDetect_enum,VDDM_EngagePFail_flg,VDDM_DisengagePFail_flg,VDDM_VCURAPSErrLv2_flg,VDDM_VCURAPSErrLv3_flg,VDDM_EDriveSysErrShifterErr_flg,VDDM_LVSysErrPwrOutErr_flg,VDDM_HVRlyOpFail_flg,VDDM_MCUActDisFail_flg,VDDM_VCUBrkSWSta_enum,VDDM_VCUFLDoorSta_flg,VDDM_VCUFRDoorSta_flg,VDDM_VCURLDoorSta_flg,VDDM_VCURRDoorSta_flg,VDDM_SysAllowReadySta_flg,VDDM_VCUHoodSWSta_flg,VDDM_VCUTailgateSWSta_flg,VDDM_CAN1BusErrorDTC_raw32,VDDM_CAN2BusErrorDTC_raw32,VDDM_CAN3BusErrorDTC_raw32,VDDM_CAN4BusErrorDTC_raw32,VDDM_CAN5BusErrorDTC_raw32,VDDM_CAN6BusErrorDTC_raw32,VDDM_CAN1BusOffDTC_raw32,VDDM_CAN2BusOffDTC_raw32,VDDM_CAN3BusOffDTC_raw32,VDDM_CAN4BusOffDTC_raw32,VDDM_CAN5BusOffDTC_raw32,VDDM_CAN6BusOffDTC_raw32
  bus_selector5 : BusSelector  OutputSignals=VDHP_ActAPSPosn_pct,VDHP_EAPS1MIN_pct,VDHP_EAPS2MIN_pct,VDHP_ResetPedalZeroPosStart_flg,VDHP_EAPS1NRM_pct,VDHP_EAPS2NRM_pct
  bus_selector6 : BusSelector  OutputSignals=VDKC_DKCTimeSN_cnt,VDKC_DKCAuthSta_enum,VDKC_TimeSNDKCFbk_cnt,VDKC_KeyMissSta_flg,VDKC_KeyModeSta_enum,VDKC_DkeyShowIVISta_enum,VDKC_KeyAreaPS_enum,VDKC_KeyAreaLockUnlock_enum,VDKC_PCommandToBCM_enum,VDKC_DKeyWelcomeSta_enum,VDKC_KeyAreaPTG_enum,VDKC_KeyAreaSPTGSta_enum,VDKC_UIDLowPowerSta_enum,VDKC_DkeyAreaRAPSSta_enum,VDKC_ParkingModeCmd_enum,VDKC_KeyNumSta_enum,VDKC_KeyTypeSta_enum,VDKC_FDCDKCAllowSleep_flg
  bus_selector7 : BusSelector  OutputSignals=VDSC_DISCTurn_flg,VDSC_DISCTargetSpd_kph,VDSC_DISCSta_enum,VDSC_DISCButtSta_flg
  bus_selector8 : BusSelector  OutputSignals=VNMM_AllCANTxReq_flg,VNMM_NMmTxReq_flg,VNMM_Awake_enum,VNMM_CSB_flg,VNMM_ErrorState_enum,VNMM_NodeID_enum,VNMM_PNI_flg,VNMM_RptMsgReq_flg,VNMM_WakeUp_enum,VNMM_ActiveWU_flg,VNMM_SysNMmSta_enum,VNMM_NetworkReq_flg
  bus_selector9 : BusSelector  OutputSignals=VPMM_PowerUpState_enum,VPMM_PowerDownState_enum,VPMM_PowerUpFault_enum,VPMM_PowerDownFault_enum,VPMM_ActiveDischargeReq_flg,VPMM_DCDCEnaReq_flg,VPMM_DCDCVoltSetpoint_V,VPMM_HVBatCnctReq_flg,VPMM_HVSysReadyToCharge_enum,VPMM_PowerSta_enum,VPMM_LVPwrSta_flg,VPMM_HVPwrSta_flg,VPMM_SysPowerMode_enum,VPMM_FrMCUEnaReq_flg,VPMM_RrMCUEnaReq_flg,VPMM_DrivetrainSelect_enum,VPMM_DrSeatSta_enum,VPMM_PwrStaSelect_enum,VPMM_PwrStaConstraint_enum,VPMM_TCountSta_enum,VPMM_PwrUpReq_enum,VPMM_PwrDownReq_enum,VPMM_LowSOCWarn_enum,VPMM_ReVehThdChkSta_enum,VPMM_EvccAplusPwrUpReq_flg,VPMM_PwrStaONTOPopReq_flg,VPMM_IVIPwrStaONTOPopT_s,VPMM_LVChrgHoldTtimer_s,VPMM_LVBattChrgTimeCnt_s,VPMM_SilentChkAllowSleep_flg,VPMM_TimerAllowSleep_flg,VPMM_FDADC12VDetAvg_mV,VPMM_PMMAllowECUSleep_flg,VPMM_LVSilentChrgSta_enum,VPMM_LVSilentChrgReq_flg,VPMM_LVSilentChrgLv_enum,VPMM_CtrlFrPwrStbA1P_flg,VPMM_CtrlFrRC1_flg,VPMM_CtrlFrBMSCCUCIR_flg,VPMM_CtrlFrEDUINVERTER_flg,VPMM_HWResetSta_enum,VPMM_CtrlDrPwrStbA2_flg,VPMM_PwrStaTOSta_enum,VPMM_Sched_ChgTOSta_enum,VPMM_PwrReq_OTA_enum,VPMM_OTAPwrReqOFFChkSta_enum,VPMM_OTAPwrReqStdChkSta_enum,VPMM_PwrReqRAPSAvail_flg
  outpmodule : Subsystem
  BOUTP_outputs : Outport  OutDataTypeStr=Bus: BOUTP_outputs
  wires:
  outpmodule/485(VOUTP_5vAPS1PwrErrDTC_raw32) -> bus_creator/485
  outpmodule/483(VOUTP_RRSensorFailDTC_raw32) -> bus_creator/483
  outpmodule/496(VOUTP_LVSysErrPwrOutErr_flg) -> bus_creator/496
  outpmodule/484(VOUTP_C1EPAS2LCDTC_raw32) -> bus_creator/484
  outpmodule/481(VOUTP_RFSensorFailDTC_raw32) -> bus_creator/481
  outpmodule/482(VOUTP_LRSensorFailDTC_raw32) -> bus_creator/482
  outpmodule/478(VOUTP_LRWheelTmpHighDTC_raw32) -> bus_creator/478
  outpmodule/479(VOUTP_RRWheelTmpHighDTC_raw32) -> bus_creator/479
  outpmodule/477(VOUTP_RFWheelTmpHighDTC_raw32) -> bus_creator/477
  outpmodule/475(VOUTP_RRPressIndiDTC_raw32) -> bus_creator/475
  outpmodule/472(VOUTP_LFPressIndiDTC_raw32) -> bus_creator/472
  outpmodule/473(VOUTP_RFPressIndiDTC_raw32) -> bus_creator/473
  outpmodule/469(VOUTP_RFBatwarnDTC_raw32) -> bus_creator/469
  outpmodule/467(VOUTP_RrMCUTqErrDTC_raw32) -> bus_creator/467
  outpmodule/466(VOUTP_FrMCUTqErrDTC_raw32) -> bus_creator/466
  outpmodule/468(VOUTP_LFBatwarnDTC_raw32) -> bus_creator/468
  outpmodule/464(VOUTP_ESC5RCErrDTC_raw32) -> bus_creator/464
  outpmodule/465(VOUTP_ESC5CSErrDTC_raw32) -> bus_creator/465
  outpmodule/462(VOUTP_ESC1RCErrDTC_raw32) -> bus_creator/462
  outpmodule/458(VOUTP_Shifter1RCErrDTC_raw32) -> bus_creator/458
  outpmodule/460(VOUTP_ESC7RCErrDTC_raw32) -> bus_creator/460
  outpmodule/454(VOUTP_MCUF1RCErrDTC_raw32) -> bus_creator/454
  outpmodule/455(VOUTP_MCUR1RCErrDTC_raw32) -> bus_creator/455
  outpmodule/451(VOUTP_CCMalfuncDetDTC_raw32) -> bus_creator/451
  outpmodule/450(VOUTP_ACCMalfuncDetDTC_raw32) -> bus_creator/450
  outpmodule/447(VOUTP_RrMCUSigErrDetDTC_raw32) -> bus_creator/447
  outpmodule/449(VOUTP_ACCAccelCmdErrDetDTC_raw32) -> bus_creator/449
  outpmodule/448(VOUTP_CCUSigErrDetDTC_raw32) -> bus_creator/448
  outpmodule/445(VOUTP_FCMACCSigErrDetDTC_raw32) -> bus_creator/445
  outpmodule/443(VOUTP_ZoneSCPNoComDTC_raw32) -> bus_creator/443
  outpmodule/444(VOUTP_BMSSigErrDetDTC_raw32) -> bus_creator/444
  outpmodule/440(VOUTP_FCM4CSErrDTC_raw32) -> bus_creator/440
  outpmodule/439(VOUTP_FCM4NoComDTC_raw32) -> bus_creator/439
  outpmodule/437(VOUTP_FCM3RCErrDTC_raw32) -> bus_creator/437
  outpmodule/436(VOUTP_FCM3NoComDTC_raw32) -> bus_creator/436
  outpmodule/432(VOUTP_RLRUSSDTC_raw32) -> bus_creator/432
  outpmodule/430(VOUTP_FLRUSSDTC_raw32) -> bus_creator/430
  outpmodule/431(VOUTP_RLLUSSDTC_raw32) -> bus_creator/431
  outpmodule/429(VOUTP_FLLUSSDTC_raw32) -> bus_creator/429
  outpmodule/425(VOUTP_RCLUSSDTC_raw32) -> bus_creator/425
  outpmodule/426(VOUTP_RMLUSSDTC_raw32) -> bus_creator/426
  outpmodule/422(VOUTP_FMLUSSDTC_raw32) -> bus_creator/422
  outpmodule/423(VOUTP_FMRUSSDTC_raw32) -> bus_creator/423
  outpmodule/424(VOUTP_FCRUSSDTC_raw32) -> bus_creator/424
  outpmodule/420(VOUTP_DiagRRTSDTC_raw32) -> bus_creator/420
  outpmodule/421(VOUTP_FCLUSSDTC_raw32) -> bus_creator/421
  outpmodule/419(VOUTP_DiagRLTSDTC_raw32) -> bus_creator/419
  outpmodule/418(VOUTP_DiagFRTSDTC_raw32) -> bus_creator/418
  outpmodule/417(VOUTP_DiagFLTSDTC_raw32) -> bus_creator/417
  outpmodule/416(VOUTP_DiagHCrashDTC_raw32) -> bus_creator/416
  outpmodule/493(VOUTP_VCURAPSErrLv2_flg) -> bus_creator/493
  outpmodule/492(VOUTP_DisengagePFail_flg) -> bus_creator/492
  outpmodule/490(VOUTP_DTCDetect_enum) -> bus_creator/490
  outpmodule/489(VOUTP_LimpHomeActTmp_flg) -> bus_creator/489
  outpmodule/488(VOUTP_EPBUnlockTODTC_raw32) -> bus_creator/488
  outpmodule/410(VOUTP_MCUR1NoComDTC_raw32) -> bus_creator/410
  outpmodule/412(VOUTP_ESC7NoComDTC_raw32) -> bus_creator/412
  outpmodule/415(VOUTP_EnterNewOperCyc_flg) -> bus_creator/415
  outpmodule/409(VOUTP_MCUF1NoComDTC_raw32) -> bus_creator/409
  outpmodule/405(VOUTP_VehMalfunLevel_enum) -> bus_creator/405
  outpmodule/400(VOUTP_FRDoorSWDTC_raw32) -> bus_creator/400
  outpmodule/402(VOUTP_HoodSWDTC_raw32) -> bus_creator/402
  outpmodule/401(VOUTP_RRDoorSWDTC_raw32) -> bus_creator/401
  outpmodule/399(VOUTP_RLDoorSWDTC_raw32) -> bus_creator/399
  outpmodule/398(VOUTP_FLDoorSWDTC_raw32) -> bus_creator/398
  outpmodule/396(VOUTP_LVSupHiDTC_raw32) -> bus_creator/396
  outpmodule/397(VOUTP_DrStSWDTC_raw32) -> bus_creator/397
  outpmodule/394(VOUTP_IniLVLoDTC_raw32) -> bus_creator/394
  outpmodule/391(VOUTP_HVRlyOpDTC_raw32) -> bus_creator/391
  outpmodule/392(VOUTP_MCUActDTC_raw32) -> bus_creator/392
  outpmodule/388(VOUTP_MidLvSaChkDTC_raw32) -> bus_creator/388
  outpmodule/386(VOUTP_DCDCEnaDTC_raw32) -> bus_creator/386
  outpmodule/387(VOUTP_HiLvSaChkDTC_raw32) -> bus_creator/387
  outpmodule/383(VOUTP_DCDC4PreDTC_raw32) -> bus_creator/383
  outpmodule/382(VOUTP_MCU4PreDTC_raw32) -> bus_creator/382
  outpmodule/381(VOUTP_HVB4PreDTC_raw32) -> bus_creator/381
  outpmodule/380(VOUTP_ONtoRdyDTC_raw32) -> bus_creator/380
  outpmodule/379(VOUTP_KeyAuthDTC_raw32) -> bus_creator/379
  outpmodule/378(VOUTP_BrkSWNoBacDTC_raw32) -> bus_creator/378
  outpmodule/376(VOUTP_Lv4ErrDTC_raw32) -> bus_creator/376
  outpmodule/374(VOUTP_Lv2ErrDTC_raw32) -> bus_creator/374
  outpmodule/373(VOUTP_Lv1ErrDTC_raw32) -> bus_creator/373
  outpmodule/372(VOUTP_C1ABM1LCDTC_raw32) -> bus_creator/372
  outpmodule/371(VOUTP_C1ABM1CSDTC_raw32) -> bus_creator/371
  outpmodule/368(VOUTP_C3CCU2CSDTC_raw32) -> bus_creator/368
  outpmodule/367(VOUTP_C3CCU2RCDTC_raw32) -> bus_creator/367
  outpmodule/366(VOUTP_C3CCU1LCDTC_raw32) -> bus_creator/366
  outpmodule/364(VOUTP_C3CCU1RCDTC_raw32) -> bus_creator/364
  outpmodule/359(VOUTP_C3BMS6CSDTC_raw32) -> bus_creator/359
  outpmodule/356(VOUTP_WinLROpenedSta_pct) -> bus_creator/356
  outpmodule/355(VOUTP_WinRFOpenedSta_pct) -> bus_creator/355
  outpmodule/354(VOUTP_WinLFOpenedSta_pct) -> bus_creator/354
  outpmodule/353(VOUTP_CLWinLockDrStaMem_enum) -> bus_creator/353
  outpmodule/350(VOUTP_DrRWdwReqAP_enum) -> bus_creator/350
  outpmodule/347(VOUTP_AutoWipHSpdENSta_flg) -> bus_creator/347
  outpmodule/348(VOUTP_DrvWdwReqAP_enum) -> bus_creator/348
  outpmodule/345(VOUTP_HMIKey7FuncSta_enum) -> bus_creator/345
  outpmodule/344(VOUTP_HMIKey6FuncSta_enum) -> bus_creator/344
  outpmodule/341(VOUTP_HMIKey3FuncSta_enum) -> bus_creator/341
  outpmodule/343(VOUTP_HMIKey5FuncSta_enum) -> bus_creator/343
  outpmodule/340(VOUTP_HMIKey2FuncSta_enum) -> bus_creator/340
  outpmodule/338(VOUTP_AutoUnlockMem_enum) -> bus_creator/338
  outpmodule/339(VOUTP_HMIKey1FuncSta_enum) -> bus_creator/339
  outpmodule/337(VOUTP_AutoUnlockSta_flg) -> bus_creator/337
  outpmodule/335(VOUTP_AutoLockSta_flg) -> bus_creator/335
  outpmodule/414(VOUTP_ESC5NoComDTC_raw32) -> bus_creator/414
  outpmodule/336(VOUTP_AutoLockMem_enum) -> bus_creator/336
  bus_selector2/105 -> outpmodule/108(VAPM_LatAccelTimeOut_flg)  "<VAPM_LatAccelTimeOut_flg>"
  bus_selector2/106 -> outpmodule/109(VAPM_LongAccel_Gps)  "<VAPM_LongAccel_Gps>"
  bus_selector2/99 -> outpmodule/102(VAPM_SASVTimeOut_flg)  "<VAPM_SASVTimeOut_flg>"
  bus_selector2/100 -> outpmodule/103(VAPM_GRADE_Deg)  "<VAPM_GRADE_Deg>"
  bus_selector2/98 -> outpmodule/101(VAPM_SASV_flg)  "<VAPM_SASV_flg>"
  bus_selector2/95 -> outpmodule/98(VAPM_SASSpeedValidTimeOut_flg)  "<VAPM_SASSpeedValidTimeOut_flg>"
  bus_selector2/92 -> outpmodule/95(VAPM_SASSpeed_degps)  "<VAPM_SASSpeed_degps>"
  bus_selector2/94 -> outpmodule/97(VAPM_SASSpeedValid_flg)  "<VAPM_SASSpeedValid_flg>"
  bus_selector2/93 -> outpmodule/96(VAPM_SASSpeedTimeOut_flg)  "<VAPM_SASSpeedTimeOut_flg>"
  bus_selector2/89 -> outpmodule/92(VAPM_EPSAOIControlTimeOut_flg)  "<VAPM_EPSAOIControlTimeOut_flg>"
  bus_selector2/86 -> outpmodule/89(VAPM_DriIntend_enum)  "<VAPM_DriIntend_enum>"
  bus_selector2/87 -> outpmodule/90(VAPM_DriIntendTimeOut_flg)  "<VAPM_DriIntendTimeOut_flg>"
  bus_selector2/117 -> outpmodule/120(VAPM_MCPressureVTimeOut_flg)  "<VAPM_MCPressureVTimeOut_flg>"
  bus_selector2/115 -> outpmodule/118(VAPM_LongAccelVTimeOut_flg)  "<VAPM_LongAccelVTimeOut_flg>"
  bus_selector2/109 -> outpmodule/112(VAPM_MCPressureTimeOut_flg)  "<VAPM_MCPressureTimeOut_flg>"
  outpmodule/403(VOUTP_TailgaSWDTC_raw32) -> bus_creator/403
  bus_selector2/112 -> outpmodule/115(VAPM_LatAccelV_flg)  "<VAPM_LatAccelV_flg>"
  bus_selector2/107 -> outpmodule/110(VAPM_LongAccelTimeOut_flg)  "<VAPM_LongAccelTimeOut_flg>"
  outpmodule/877(VOUTP_RFP20_raw8) -> bus_creator/877
  outpmodule/875(VOUTP_ALFin_flg) -> bus_creator/875
  outpmodule/874(VOUTP_S4L_enum) -> bus_creator/874
  outpmodule/872(VOUTP_S2L_enum) -> bus_creator/872
  outpmodule/871(VOUTP_S1L_enum) -> bus_creator/871
  outpmodule/869(VOUTP_S3ID_raw32) -> bus_creator/869
  outpmodule/864(VOUTP_RFSensorMode_flg) -> bus_creator/864
  outpmodule/862(VOUTP_AutoLTips_enum) -> bus_creator/862
  outpmodule/860(VOUTP_RRWheelPSW_raw8) -> bus_creator/860
  outpmodule/857(VOUTP_LFWheelPSW_raw8) -> bus_creator/857
  outpmodule/856(VOUTP_RRWheelTmpIndi_flg) -> bus_creator/856
  outpmodule/852(VOUTP_TPMSWarnIndi_enum) -> bus_creator/852
  outpmodule/850(VOUTP_LRPressIndi_enum) -> bus_creator/850
  outpmodule/849(VOUTP_RFPressIndi_enum) -> bus_creator/849
  outpmodule/847(VOUTP_TPMSCaliButtAllow_flg) -> bus_creator/847
  outpmodule/843(VOUTP_LRWheelDebug_flg) -> bus_creator/843
  outpmodule/845(VOUTP_RRWheelDebug_flg) -> bus_creator/845
  outpmodule/842(VOUTP_LFWheelDebug_flg) -> bus_creator/842
  outpmodule/841(VOUTP_RRSensorFail_flg) -> bus_creator/841
  outpmodule/837(VOUTP_RRWheelTemp_C) -> bus_creator/837
  outpmodule/835(VOUTP_RFWheelTemp_C) -> bus_creator/835
  outpmodule/834(VOUTP_LFWheelTemp_C) -> bus_creator/834
  outpmodule/831(VOUTP_RFWheelPress_raw8) -> bus_creator/831
  outpmodule/818(VOUTP_LVentEN_flg) -> bus_creator/818
  outpmodule/819(VOUTP_CLVentEN_flg) -> bus_creator/819
  outpmodule/816(VOUTP_FOOTSet_enum) -> bus_creator/816
  outpmodule/814(VOUTP_ACModeSet457_enum) -> bus_creator/814
  outpmodule/813(VOUTP_ACModeSet123_enum) -> bus_creator/813
  outpmodule/812(VOUTP_SettempZon1Set7_enum) -> bus_creator/812
  bus_selector2/119 -> outpmodule/122(VAPM_BrkSwStaTimeOut_flg)  "<VAPM_BrkSwStaTimeOut_flg>"
  bus_selector2/108 -> outpmodule/111(VAPM_MCPressure_bar)  "<VAPM_MCPressure_bar>"
  outpmodule/807(VOUTP_SettempZon1Set1_enum) -> bus_creator/807
  outpmodule/806(VOUTP_FDCTHCCREVentYStaSet7_enum) -> bus_creator/806
  outpmodule/803(VOUTP_FDCTHCCREVentYStaSet3_enum) -> bus_creator/803
  outpmodule/327(VOUTP_PTGOpenHeight57_enum) -> bus_creator/327
  bus_selector2/97 -> outpmodule/100(VAPM_SASCALTimeOut_flg)  "<VAPM_SASCALTimeOut_flg>"
  outpmodule/333(VOUTP_LRightStaCmd_flg) -> bus_creator/333
  outpmodule/323(VOUTP_PTGUserHeight5_cnt) -> bus_creator/323
  outpmodule/322(VOUTP_PTGUserHeight4_cnt) -> bus_creator/322
  outpmodule/321(VOUTP_PTGUserHeight3_cnt) -> bus_creator/321
  outpmodule/319(VOUTP_PTGUserHeight1_cnt) -> bus_creator/319
  outpmodule/317(VOUTP_PTGOpenHeightSta_enum) -> bus_creator/317
  outpmodule/315(VOUTP_HoodRelCmd_flg) -> bus_creator/315
  outpmodule/314(VOUTP_FollowMeENFunSta_flg) -> bus_creator/314
  outpmodule/310(VOUTP_FollowMeENMem_enum) -> bus_creator/310
  outpmodule/311(VOUTP_WalkInUnLkENFunSta_flg) -> bus_creator/311
  outpmodule/306(VOUTP_WalkInUnLkENMem_enum) -> bus_creator/306
  outpmodule/303(VOUTP_FDRHandleLampCmd_flg) -> bus_creator/303
  outpmodule/300(VOUTP_TurnSwTimeSetSta123_enum) -> bus_creator/300
  outpmodule/298(VOUTP_SPTGENFunMem_enum) -> bus_creator/298
  bus_selector2/82 -> outpmodule/85(VAPM_RRPulseCount_enum)  "<VAPM_RRPulseCount_enum>"
  outpmodule/295(VOUTP_TurnSwSta_enum) -> bus_creator/295
  outpmodule/293(VOUTP_FWipSwSta_enum) -> bus_creator/293
  outpmodule/292(VOUTP_PassSWSta_flg) -> bus_creator/292
  outpmodule/290(VOUTP_HazardIND_flg) -> bus_creator/290
  outpmodule/288(VOUTP_AmbBrightnessSta5_enum) -> bus_creator/288
  outpmodule/287(VOUTP_AmbBrightnessSta4_enum) -> bus_creator/287
  outpmodule/284(VOUTP_AmbBrightnessSta1_enum) -> bus_creator/284
  outpmodule/331(VOUTP_ACCLevelMem34_enum) -> bus_creator/331
  outpmodule/283(VOUTP_AmbColorSta7_enum) -> bus_creator/283
  outpmodule/282(VOUTP_AmbColorSta5_enum) -> bus_creator/282
  outpmodule/275(VOUTP_AmbLinkDriStaFlash_enum) -> bus_creator/275
  outpmodule/273(VOUTP_AmbWelENFlash_enum) -> bus_creator/273
  outpmodule/270(VOUTP_fUnlockSingle_flg) -> bus_creator/270
  outpmodule/271(VOUTP_UserNow_enum) -> bus_creator/271
  outpmodule/268(VOUTP_LockAlarm_enum) -> bus_creator/268
  outpmodule/263(VOUTP_AmbLinkDriSta_flg) -> bus_creator/263
  outpmodule/260(VOUTP_AmbFunEN_flg) -> bus_creator/260
  outpmodule/255(VOUTP_DrvWdwCtrlCmd_pct) -> bus_creator/255
  outpmodule/254(VOUTP_PTGInnerSW2_enum) -> bus_creator/254
  outpmodule/328(VOUTP_SenstivityPosnCmd_enum) -> bus_creator/328
  outpmodule/334(VOUTP_LLeftStaCmd_flg) -> bus_creator/334
  outpmodule/901(VOUTP_WriteChkLRID_raw) -> bus_creator/901
  outpmodule/900(VOUTP_WriteChkRFID_raw) -> bus_creator/900
  outpmodule/894(VOUTP_TPMSResButt_flg) -> bus_creator/894
  outpmodule/893(VOUTP_ChkStorge_flg) -> bus_creator/893
  outpmodule/891(VOUTP_SetIDLoc_flg) -> bus_creator/891
  outpmodule/889(VOUTP_ID4messageALTU_raw8) -> bus_creator/889
  outpmodule/890(VOUTP_Chkfin_flg) -> bus_creator/890
  outpmodule/887(VOUTP_ID2messageALTU_raw8) -> bus_creator/887
  outpmodule/882(VOUTP_S1WheelDebugALTU_pct) -> bus_creator/882
  outpmodule/881(VOUTP_IDin_raw32) -> bus_creator/881
  outpmodule/879(VOUTP_RRP20_raw8) -> bus_creator/879
  outpmodule/878(VOUTP_LRP20_raw8) -> bus_creator/878
  outpmodule/910(VOUTP_unlearnSfailvalid_enum) -> bus_creator/910
  outpmodule/909(VOUTP_unlearnSfali_flg) -> bus_creator/909
  outpmodule/908(VOUTP_Flashdatavalid_enum) -> bus_creator/908
  outpmodule/905(VOUTP_WriteChkfinLRID_raw) -> bus_creator/905
  outpmodule/903(VOUTP_WriteChkfinLFID_raw) -> bus_creator/903
  outpmodule/904(VOUTP_WriteChkfinRFID_raw) -> bus_creator/904
  outpmodule/796(VOUTP_FDCTHCREVentYStaSet2_enum) -> bus_creator/796
  outpmodule/817(VOUTP_FrostSet_enum) -> bus_creator/817
  outpmodule/794(VOUTP_FDCTHCCLEVentYStaSet7_enum) -> bus_creator/794
  outpmodule/790(VOUTP_FDCTHCCLEVentYStaSet2_enum) -> bus_creator/790
  outpmodule/792(VOUTP_FDCTHCCLEVentYStaSet4_enum) -> bus_creator/792
  outpmodule/272(VOUTP_AmbFunENFlash_enum) -> bus_creator/272
  outpmodule/786(VOUTP_FDCTHCLEVentYStaSet4_enum) -> bus_creator/786
  outpmodule/785(VOUTP_FDCTHCLEVentYStaSet3_enum) -> bus_creator/785
  outpmodule/404(VOUTP_EDriveSysErrVCUErr_flg) -> bus_creator/404
  outpmodule/783(VOUTP_FDCTHCLEVentYStaSet1_enum) -> bus_creator/783
  outpmodule/779(VOUTP_FDCTHCCREVentZStaSet3_enum) -> bus_creator/779
  outpmodule/780(VOUTP_FDCTHCCREVentZStaSet4_enum) -> bus_creator/780
  outpmodule/778(VOUTP_FDCTHCCREVentZStaSet2_enum) -> bus_creator/778
  outpmodule/769(VOUTP_FDCTHCCLEVentZStaSet5_enum) -> bus_creator/769
  outpmodule/765(VOUTP_FDCTHCCLEVentZStaSet1_enum) -> bus_creator/765
  outpmodule/767(VOUTP_FDCTHCCLEVentZStaSet3_enum) -> bus_creator/767
  outpmodule/763(VOUTP_FDCTHCLEVentZStaSet5_enum) -> bus_creator/763
  outpmodule/760(VOUTP_FDCTHCLEVentZStaSet2_enum) -> bus_creator/760
  outpmodule/756(VOUTP_LEVentModeStaSet457_enum) -> bus_creator/756
  outpmodule/755(VOUTP_LEVentModeStaSet123_enum) -> bus_creator/755
  outpmodule/754(VOUTP_CRVentENSet_enum) -> bus_creator/754
  outpmodule/752(VOUTP_CLVentENSet_enum) -> bus_creator/752
  outpmodule/750(VOUTP_FDCFGSAirIntStaSet457_enum) -> bus_creator/750
  outpmodule/746(VOUTP_IONSWStaSet_enum) -> bus_creator/746
  outpmodule/745(VOUTP_AirIntenZone3MSet7_enum) -> bus_creator/745
  outpmodule/744(VOUTP_AirIntenZone3MSet5_enum) -> bus_creator/744
  outpmodule/742(VOUTP_AirIntenZone3MSet3_enum) -> bus_creator/742
  outpmodule/743(VOUTP_AirIntenZone3MSet4_enum) -> bus_creator/743
  outpmodule/739(VOUTP_AirIntenZone1MSet7_enum) -> bus_creator/739
  outpmodule/737(VOUTP_AirIntenZone1MSet4_enum) -> bus_creator/737
  outpmodule/733(VOUTP_RecyAutoSet_enum) -> bus_creator/733
  outpmodule/851(VOUTP_RRPressIndi_enum) -> bus_creator/851
  outpmodule/735(VOUTP_AirIntenZone1MSet2_enum) -> bus_creator/735
  outpmodule/731(VOUTP_CCUSyncStsSet_enum) -> bus_creator/731
  outpmodule/727(VOUTP_EWPBUflag3_flg) -> bus_creator/727
  outpmodule/726(VOUTP_EWPBUflag2_flg) -> bus_creator/726
  outpmodule/725(VOUTP_EWPBUflag1_flg) -> bus_creator/725
  bus_selector13/38 -> outpmodule/960(VTQD_CreepON_flg)  "<VTQD_CreepON_flg>"
  bus_selector13/29 -> outpmodule/951(VTQD_FrIdcMin_A)  "<VTQD_FrIdcMin_A>"
  bus_selector13/21 -> outpmodule/943(VTQD_FrEDUSpdValid_flg)  "<VTQD_FrEDUSpdValid_flg>"
  bus_selector13/24 -> outpmodule/946(VTQD_RrEDUAvailBrkRgnTqV_flg)  "<VTQD_RrEDUAvailBrkRgnTqV_flg>"
  bus_selector13/23 -> outpmodule/945(VTQD_RrEDUSpdValid_flg)  "<VTQD_RrEDUSpdValid_flg>"
  outpmodule/826(VOUTP_LFBatWarn_flg) -> bus_creator/826
  bus_selector13/18 -> outpmodule/940(VTQD_RrEDURolRgnTq_Nm)  "<VTQD_RrEDURolRgnTq_Nm>"
  bus_selector13/13 -> outpmodule/935(VTQD_DriverWhlTqDemFr_Nm)  "<VTQD_DriverWhlTqDemFr_Nm>"
  bus_selector13/14 -> outpmodule/936(VTQD_DriverWhlTqDemRr_Nm)  "<VTQD_DriverWhlTqDemRr_Nm>"
  bus_selector13/11 -> outpmodule/933(VTQD_FrRgnDecrSta_flg)  "<VTQD_FrRgnDecrSta_flg>"
  bus_selector13/7 -> outpmodule/929(VTQD_ShiftGearPosn_enum)  "<VTQD_ShiftGearPosn_enum>"
  outpmodule/721(VOUTP_FDCFGSChCmd_enum) -> bus_creator/721
  outpmodule/278(VOUTP_AmbColorSta1_enum) -> bus_creator/278
  bus_selector13/8 -> outpmodule/930(VTQD_PButtonSta_enum)  "<VTQD_PButtonSta_enum>"
  bus_selector13/4 -> outpmodule/926(VTQD_FrEDUAvailBrkRgnTq_Nm)  "<VTQD_FrEDUAvailBrkRgnTq_Nm>"
  bus_selector13/1 -> outpmodule/923(VTQD_ParkRequest_flg)  "<VTQD_ParkRequest_flg>"
  bus_selector13/2 -> outpmodule/924(VTQD_TqSourceFr_enum)  "<VTQD_TqSourceFr_enum>"
  outpmodule/870(VOUTP_S4ID_raw32) -> bus_creator/870
  BTPM_outputs/1 -> bus_selector12/1
  bus_selector12/97 -> outpmodule/922(VTPM_ModelVersionChksum_raw)  "<VTPM_ModelVersionChksum_raw>"
  bus_selector12/93 -> outpmodule/918(VTPM_TPMSTLCmd_flg)  "<VTPM_TPMSTLCmd_flg>"
  outpmodule/795(VOUTP_FDCTHCREVentYStaSet1_enum) -> bus_creator/795
  bus_selector12/89 -> outpmodule/914(VTPM_FlashS3ID_raw)  "<VTPM_FlashS3ID_raw>"
  bus_selector12/90 -> outpmodule/915(VTPM_FlashS4ID_raw)  "<VTPM_FlashS4ID_raw>"
  outpmodule/312(VOUTP_WalkOutLkENFunSta_flg) -> bus_creator/312
  bus_selector12/86 -> outpmodule/911(VTPM_Prepresstempvalid_enum)  "<VTPM_Prepresstempvalid_enum>"
  outpmodule/435(VOUTP_FCM2CSErrDTC_raw32) -> bus_creator/435
  bus_selector12/88 -> outpmodule/913(VTPM_FlashS2ID_raw)  "<VTPM_FlashS2ID_raw>"
  bus_selector12/84 -> outpmodule/909(VTPM_unlearnSfali_flg)  "<VTPM_unlearnSfali_flg>"
  outpmodule/302(VOUTP_FDLHandleLampCmd_flg) -> bus_creator/302
  bus_selector12/79 -> outpmodule/904(VTPM_WriteChkfinRFID_raw)  "<VTPM_WriteChkfinRFID_raw>"
  outpmodule/486(VOUTP_5vAPS2PwrErrDTC_raw32) -> bus_creator/486
  bus_selector12/81 -> outpmodule/906(VTPM_WriteChkfinRRID_raw)  "<VTPM_WriteChkfinRRID_raw>"
  outpmodule/720(VOUTP_FDCFGSFuncSta_enum) -> bus_creator/720
  bus_selector12/13 -> outpmodule/838(VTPM_LFSensorFail_flg)  "<VTPM_LFSensorFail_flg>"
  bus_selector12/11 -> outpmodule/836(VTPM_LRWheelTemp_C)  "<VTPM_LRWheelTemp_C>"
  bus_selector12/12 -> outpmodule/837(VTPM_RRWheelTemp_C)  "<VTPM_RRWheelTemp_C>"
  bus_selector12/9 -> outpmodule/834(VTPM_LFWheelTemp_C)  "<VTPM_LFWheelTemp_C>"
  bus_selector12/7 -> outpmodule/832(VTPM_LRWheelPress_raw8)  "<VTPM_LRWheelPress_raw8>"
  bus_selector12/5 -> outpmodule/830(VTPM_LFWheelPress_raw8)  "<VTPM_LFWheelPress_raw8>"
  bus_selector12/1 -> outpmodule/826(VTPM_LFBatWarn_flg)  "<VTPM_LFBatWarn_flg>"
  bus_selector12/77 -> outpmodule/902(VTPM_WriteChkRRID_raw)  "<VTPM_WriteChkRRID_raw>"
  bus_selector12/75 -> outpmodule/900(VTPM_WriteChkRFID_raw)  "<VTPM_WriteChkRFID_raw>"
  bus_selector12/71 -> outpmodule/896(VTPM_RFPind_enum)  "<VTPM_RFPind_enum>"
  bus_selector12/67 -> outpmodule/892(VTPM_TPMSStorge_flg)  "<VTPM_TPMSStorge_flg>"
  bus_selector12/66 -> outpmodule/891(VTPM_SetIDLoc_flg)  "<VTPM_SetIDLoc_flg>"
  bus_selector12/61 -> outpmodule/886(VTPM_ID1messageALTU_raw8)  "<VTPM_ID1messageALTU_raw8>"
  outpmodule/294(VOUTP_FWasSwSta_enum) -> bus_creator/294
  bus_selector12/58 -> outpmodule/883(VTPM_S2WheelDebugALTU_pct)  "<VTPM_S2WheelDebugALTU_pct>"
  bus_selector12/55 -> outpmodule/880(VTPM_FAT_flg)  "<VTPM_FAT_flg>"
  outpmodule/798(VOUTP_FDCTHCREVentYStaSet4_enum) -> bus_creator/798
  bus_selector12/50 -> outpmodule/875(VTPM_ALFin_flg)  "<VTPM_ALFin_flg>"
  bus_selector12/51 -> outpmodule/876(VTPM_LFP20_raw8)  "<VTPM_LFP20_raw8>"
  bus_selector12/46 -> outpmodule/871(VTPM_S1L_enum)  "<VTPM_S1L_enum>"
  bus_selector12/47 -> outpmodule/872(VTPM_S2L_enum)  "<VTPM_S2L_enum>"
  bus_selector12/39 -> outpmodule/864(VTPM_RFSensorMode_flg)  "<VTPM_RFSensorMode_flg>"
  bus_selector12/42 -> outpmodule/867(VTPM_S1ID_raw32)  "<VTPM_S1ID_raw32>"
  bus_selector2/83 -> outpmodule/86(VAPM_RRPulseCountTimeOut_flg)  "<VAPM_RRPulseCountTimeOut_flg>"
  bus_selector12/38 -> outpmodule/863(VTPM_LFSensorMode_flg)  "<VTPM_LFSensorMode_flg>"
  outpmodule/411(VOUTP_Shifter1NoComDTC_raw32) -> bus_creator/411
  bus_selector12/29 -> outpmodule/854(VTPM_RFWheelTmpIndi_flg)  "<VTPM_RFWheelTmpIndi_flg>"
  bus_selector12/32 -> outpmodule/857(VTPM_LFWheelPSW_raw8)  "<VTPM_LFWheelPSW_raw8>"
  bus_selector12/27 -> outpmodule/852(VTPM_TPMSWarnIndi_enum)  "<VTPM_TPMSWarnIndi_enum>"
  bus_selector12/26 -> outpmodule/851(VTPM_RRPressIndi_enum)  "<VTPM_RRPressIndi_enum>"
  bus_selector12/24 -> outpmodule/849(VTPM_RFPressIndi_enum)  "<VTPM_RFPressIndi_enum>"
  bus_selector12/23 -> outpmodule/848(VTPM_LFPressIndi_enum)  "<VTPM_LFPressIndi_enum>"
  bus_selector12/21 -> outpmodule/846(VTPM_TPMSResButtAllow_flg)  "<VTPM_TPMSResButtAllow_flg>"
  bus_selector12/20 -> outpmodule/845(VTPM_RRWheelDebug_flg)  "<VTPM_RRWheelDebug_flg>"
  bus_selector12/16 -> outpmodule/841(VTPM_RRSensorFail_flg)  "<VTPM_RRSensorFail_flg>"
  bus_selector12/19 -> outpmodule/844(VTPM_RFWheelDebug_flg)  "<VTPM_RFWheelDebug_flg>"
  bus_selector12/18 -> outpmodule/843(VTPM_LRWheelDebug_flg)  "<VTPM_LRWheelDebug_flg>"
  outpmodule/718(VOUTP_FDCFGSChSta_enum) -> bus_creator/718
  outpmodule/715(VOUTP_FDCTHCCRVentENSta_flg) -> bus_creator/715
  outpmodule/716(VOUTP_FDCTHCMAPTCForceOFFSta_flg) -> bus_creator/716
  outpmodule/713(VOUTP_FDCTHCRVentENSta_flg) -> bus_creator/713
  outpmodule/712(VOUTP_FDCTHCREVentYSta_enum) -> bus_creator/712
  outpmodule/709(VOUTP_FDCTHCLVentENSta_flg) -> bus_creator/709
  outpmodule/708(VOUTP_FDCTHCLEVentYSta_enum) -> bus_creator/708
  outpmodule/707(VOUTP_FDCTHCCREVentZSta_enum) -> bus_creator/707
  bus_selector12/62 -> outpmodule/887(VTPM_ID2messageALTU_raw8)  "<VTPM_ID2messageALTU_raw8>"
  outpmodule/705(VOUTP_FDCTHCCLEVentZSta_enum) -> bus_creator/705
  outpmodule/700(VOUTP_sigDfrstSt_flg) -> bus_creator/700
  outpmodule/696(VOUTP_RecAutoFlg_flg) -> bus_creator/696
  outpmodule/697(VOUTP_AirIntenZone1M_enum) -> bus_creator/697
  outpmodule/822(VOUTP_FDCFGSLearnCmd_enum) -> bus_creator/822
  outpmodule/693(VOUTP_FaceM_flg) -> bus_creator/693
  outpmodule/690(VOUTP_Face_flg) -> bus_creator/690
  outpmodule/686(VOUTP_sigCbnAirT_C) -> bus_creator/686
  outpmodule/685(VOUTP_sigAmbAirT_C) -> bus_creator/685
  outpmodule/682(VOUTP_sigCbnSolarLeft_W) -> bus_creator/682
  outpmodule/679(VOUTP_sigSetTempZon1St_C) -> bus_creator/679
  outpmodule/681(VOUTP_sigClntTHvBattOut_C) -> bus_creator/681
  outpmodule/675(VOUTP_CCUSyncLampSts_flg) -> bus_creator/675
  outpmodule/757(VOUTP_REVentModeStaSet123_enum) -> bus_creator/757
  outpmodule/676(VOUTP_sigAirIntenZon1St_enum) -> bus_creator/676
  outpmodule/258(VOUTP_PsRWdwCtrlCmd_pct) -> bus_creator/258
  outpmodule/670(VOUTP_EDriveMode_enum) -> bus_creator/670
  outpmodule/667(VOUTP_FDRrAPTCHeatPwrCmd_W) -> bus_creator/667
  outpmodule/665(VOUTP_FDFrLeAPTCHeatPwrCmd_W) -> bus_creator/665
  outpmodule/257(VOUTP_DrRWdwCtrlCmd_pct) -> bus_creator/257
  outpmodule/661(VOUTP_FDAGSCmd_enum) -> bus_creator/661
  outpmodule/662(VOUTP_FDEWP1Cmd_enum) -> bus_creator/662
  outpmodule/659(VOUTP_FDFrWPTCHeatPwrCmd_W) -> bus_creator/659
  outpmodule/656(VOUTP_FDSOTXVCmd_flg) -> bus_creator/656
  outpmodule/657(VOUTP_FDFWVCmd_flg) -> bus_creator/657
  outpmodule/655(VOUTP_FDEXV2Cmd_step) -> bus_creator/655
  outpmodule/824(VOUTP_THSysErrlampReq_flg) -> bus_creator/824
  outpmodule/654(VOUTP_FDEXV1Cmd_step) -> bus_creator/654
  outpmodule/646(VOUTP_DrivingMode_cnt) -> bus_creator/646
  outpmodule/647(VOUTP_ModelYear_cnt) -> bus_creator/647
  outpmodule/645(VOUTP_PmicBootPath_raw32) -> bus_creator/645
  outpmodule/643(VOUTP_ECUGen1_cnt) -> bus_creator/643
  outpmodule/642(VOUTP_CurrentNmState_enum) -> bus_creator/642
  outpmodule/635(VOUTP_SHA8_cnt) -> bus_creator/635
  bus_selector12/31 -> outpmodule/856(VTPM_RRWheelTmpIndi_flg)  "<VTPM_RRWheelTmpIndi_flg>"
  outpmodule/636(VOUTP_NvWriteReqRisingEdge_flg) -> bus_creator/636
  outpmodule/632(VOUTP_SHA5_cnt) -> bus_creator/632
  outpmodule/758(VOUTP_REVentModeStaSet457_enum) -> bus_creator/758
  outpmodule/634(VOUTP_SHA7_cnt) -> bus_creator/634
  outpmodule/633(VOUTP_SHA6_cnt) -> bus_creator/633
  outpmodule/630(VOUTP_SHA3_cnt) -> bus_creator/630
  outpmodule/628(VOUTP_SHA1_cnt) -> bus_creator/628
  bus_selector12/59 -> outpmodule/884(VTPM_S3WheelDebugALTU_pct)  "<VTPM_S3WheelDebugALTU_pct>"
  outpmodule/627(VOUTP_Dash2_cnt) -> bus_creator/627
  outpmodule/626(VOUTP_Change2_cnt) -> bus_creator/626
  outpmodule/895(VOUTP_LFPindi_enum) -> bus_creator/895
  outpmodule/622(VOUTP_Country2_cnt) -> bus_creator/622
  bus_selector2/116 -> outpmodule/119(VAPM_MCPressureV_bar)  "<VAPM_MCPressureV_bar>"
  bus_selector12/6 -> outpmodule/831(VTPM_RFWheelPress_raw8)  "<VTPM_RFWheelPress_raw8>"
  outpmodule/623(VOUTP_Variation_cnt) -> bus_creator/623
  outpmodule/620(VOUTP_Patch2_cnt) -> bus_creator/620
  outpmodule/618(VOUTP_Minor2_cnt) -> bus_creator/618
  bus_selector13/9 -> outpmodule/931(VTQD_FrActvDmpDisabReq_flg)  "<VTQD_FrActvDmpDisabReq_flg>"
  outpmodule/619(VOUTP_Patch1_cnt) -> bus_creator/619
  outpmodule/616(VOUTP_Major2_cnt) -> bus_creator/616
  outpmodule/615(VOUTP_Major1_cnt) -> bus_creator/615
  outpmodule/614(VOUTP_ECU2_cnt) -> bus_creator/614
  bus_selector2/121 -> outpmodule/124(VAPM_BrkSwVTimeOut_flg)  "<VAPM_BrkSwVTimeOut_flg>"
  outpmodule/613(VOUTP_ECU1_cnt) -> bus_creator/613
  outpmodule/612(VOUTP_CarModel3_cnt) -> bus_creator/612
  outpmodule/607(VOUTP_HWVer1_cnt) -> bus_creator/607
  outpmodule/608(VOUTP_HWVer2_cnt) -> bus_creator/608
  outpmodule/873(VOUTP_S3L_enum) -> bus_creator/873
  outpmodule/606(VOUTP_PwrReqRAPSAvail_flg) -> bus_creator/606
  outpmodule/604(VOUTP_OTAPwrReqOFFChkSta_enum) -> bus_creator/604
  outpmodule/602(VOUTP_Sched_ChgTOSta_enum) -> bus_creator/602
  outpmodule/329(VOUTP_TimeGapLevelSta_enum) -> bus_creator/329
  outpmodule/599(VOUTP_HWResetSta_enum) -> bus_creator/599
  outpmodule/597(VOUTP_CtrlFrBMSCCUCIR_flg) -> bus_creator/597
  outpmodule/595(VOUTP_CtrlFrPwrStbA1P_flg) -> bus_creator/595
  outpmodule/594(VOUTP_LVSilentChrgLv_enum) -> bus_creator/594
  bus_selector13/27 -> outpmodule/949(VTQD_FrRgnPermSta_flg)  "<VTQD_FrRgnPermSta_flg>"
  outpmodule/593(VOUTP_LVSilentChrgReq_flg) -> bus_creator/593
  outpmodule/592(VOUTP_LVSilentChrgSta_enum) -> bus_creator/592
  bus_selector12/64 -> outpmodule/889(VTPM_ID4messageALTU_raw8)  "<VTPM_ID4messageALTU_raw8>"
  outpmodule/591(VOUTP_PMMAllowECUSleep_flg) -> bus_creator/591
  outpmodule/590(VOUTP_FDADC12VDetAvg_mV) -> bus_creator/590
  outpmodule/589(VOUTP_TimerAllowSleep_flg) -> bus_creator/589
  bus_selector13/5 -> outpmodule/927(VTQD_RrEDUAvailBrkRgnTq_Nm)  "<VTQD_RrEDUAvailBrkRgnTq_Nm>"
  outpmodule/588(VOUTP_SilentChkAllowSleep_flg) -> bus_creator/588
  outpmodule/584(VOUTP_PwrStaONTOPopReq_flg) -> bus_creator/584
  outpmodule/582(VOUTP_ReVehThdChkSta_enum) -> bus_creator/582
  outpmodule/579(VOUTP_PwrUpReq_enum) -> bus_creator/579
  outpmodule/580(VOUTP_PwrDownReq_enum) -> bus_creator/580
  outpmodule/578(VOUTP_TCountSta_enum) -> bus_creator/578
  outpmodule/577(VOUTP_PwrStaConstraint_enum) -> bus_creator/577
  outpmodule/651(VOUTP_FDSOV1Cmd_flg) -> bus_creator/651
  outpmodule/789(VOUTP_FDCTHCCLEVentYStaSet1_enum) -> bus_creator/789
  outpmodule/576(VOUTP_PwrStaSelect_enum) -> bus_creator/576
  bus_selector11/163 -> outpmodule/812(VTHC_SettempZon1Set7_enum)  "<VTHC_SettempZon1Set7_enum>"
  bus_selector11/161 -> outpmodule/810(VTHC_SettempZon1Set4_enum)  "<VTHC_SettempZon1Set4_enum>"
  bus_selector11/159 -> outpmodule/808(VTHC_SettempZon1Set2_enum)  "<VTHC_SettempZon1Set2_enum>"
  bus_selector11/157 -> outpmodule/806(VTHC_FDCTHCCREVentYStaSet7_enum)  "<VTHC_FDCTHCCREVentYStaSet7_enum>"
  outpmodule/304(VOUTP_FDHandleCmd_enum) -> bus_creator/304
  bus_selector11/153 -> outpmodule/802(VTHC_FDCTHCCREVentYStaSet2_enum)  "<VTHC_FDCTHCCREVentYStaSet2_enum>"
  bus_selector11/150 -> outpmodule/799(VTHC_FDCTHCREVentYStaSet5_enum)  "<VTHC_FDCTHCREVentYStaSet5_enum>"
  bus_selector11/151 -> outpmodule/800(VTHC_FDCTHCREVentYStaSet7_enum)  "<VTHC_FDCTHCREVentYStaSet7_enum>"
  outpmodule/351(VOUTP_PsRWdwReqAP_enum) -> bus_creator/351
  outpmodule/787(VOUTP_FDCTHCLEVentYStaSet5_enum) -> bus_creator/787
  bus_selector11/147 -> outpmodule/796(VTHC_FDCTHCREVentYStaSet2_enum)  "<VTHC_FDCTHCREVentYStaSet2_enum>"
  bus_selector11/145 -> outpmodule/794(VTHC_FDCTHCCLEVentYStaSet7_enum)  "<VTHC_FDCTHCCLEVentYStaSet7_enum>"
  bus_selector11/144 -> outpmodule/793(VTHC_FDCTHCCLEVentYStaSet5_enum)  "<VTHC_FDCTHCCLEVentYStaSet5_enum>"
  bus_selector11/143 -> outpmodule/792(VTHC_FDCTHCCLEVentYStaSet4_enum)  "<VTHC_FDCTHCCLEVentYStaSet4_enum>"
  bus_selector11/141 -> outpmodule/790(VTHC_FDCTHCCLEVentYStaSet2_enum)  "<VTHC_FDCTHCCLEVentYStaSet2_enum>"
  bus_selector13/37 -> outpmodule/959(VTQD_ReBrakeLPReq_flg)  "<VTQD_ReBrakeLPReq_flg>"
  bus_selector11/139 -> outpmodule/788(VTHC_FDCTHCLEVentYStaSet7_enum)  "<VTHC_FDCTHCLEVentYStaSet7_enum>"
  outpmodule/587(VOUTP_LVBattChrgTimeCnt_s) -> bus_creator/587
  bus_selector11/142 -> outpmodule/791(VTHC_FDCTHCCLEVentYStaSet3_enum)  "<VTHC_FDCTHCCLEVentYStaSet3_enum>"
  bus_selector13/15 -> outpmodule/937(VTQD_FrEDUActTq_Nm)  "<VTQD_FrEDUActTq_Nm>"
  outpmodule/629(VOUTP_SHA2_cnt) -> bus_creator/629
  bus_selector11/138 -> outpmodule/787(VTHC_FDCTHCLEVentYStaSet5_enum)  "<VTHC_FDCTHCLEVentYStaSet5_enum>"
  bus_selector11/136 -> outpmodule/785(VTHC_FDCTHCLEVentYStaSet3_enum)  "<VTHC_FDCTHCLEVentYStaSet3_enum>"
  bus_selector13/20 -> outpmodule/942(VTQD_RrEDUSpd_rpm)  "<VTQD_RrEDUSpd_rpm>"
  bus_selector11/134 -> outpmodule/783(VTHC_FDCTHCLEVentYStaSet1_enum)  "<VTHC_FDCTHCLEVentYStaSet1_enum>"
  bus_selector11/131 -> outpmodule/780(VTHC_FDCTHCCREVentZStaSet4_enum)  "<VTHC_FDCTHCCREVentZStaSet4_enum>"
  bus_selector11/132 -> outpmodule/781(VTHC_FDCTHCCREVentZStaSet5_enum)  "<VTHC_FDCTHCCREVentZStaSet5_enum>"
  bus_selector11/125 -> outpmodule/774(VTHC_FDCTHCREVentZStaSet4_enum)  "<VTHC_FDCTHCREVentZStaSet4_enum>"
  outpmodule/1003(VOUTP_ISODecLimit_mps2) -> bus_creator/1003
  bus_selector11/124 -> outpmodule/773(VTHC_FDCTHCREVentZStaSet3_enum)  "<VTHC_FDCTHCREVentZStaSet3_enum>"
  bus_selector11/127 -> outpmodule/776(VTHC_FDCTHCREVentZStaSet7_enum)  "<VTHC_FDCTHCREVentZStaSet7_enum>"
  outpmodule/998(VOUTP_LatAccCtrl_flg) -> bus_creator/998
  outpmodule/994(VOUTP_LimitPCT_pct) -> bus_creator/994
  outpmodule/995(VOUTP_FrontRearSlipRatioCtrl_flg) -> bus_creator/995
  outpmodule/992(VOUTP_FeatReqSpd_kph) -> bus_creator/992
  outpmodule/991(VOUTP_FeatArbitrSta_enum) -> bus_creator/991
  bus_selector11/168 -> outpmodule/817(VTHC_FrostSet_enum)  "<VTHC_FrostSet_enum>"
  outpmodule/987(VOUTP_VMCAEBCtrlAvail_flg) -> bus_creator/987
  outpmodule/668(VOUTP_FDBlowerCmd_pct) -> bus_creator/668
  outpmodule/791(VOUTP_FDCTHCCLEVentYStaSet3_enum) -> bus_creator/791
  outpmodule/985(VOUTP_VehicleSpeed_kph) -> bus_creator/985
  outpmodule/982(VOUTP_HVPO120VGrpBLDSt_enum) -> bus_creator/982
  outpmodule/362(VOUTP_C3BMS1CSDTC_raw32) -> bus_creator/362
  bus_selector12/65 -> outpmodule/890(VTPM_Chkfin_flg)  "<VTPM_Chkfin_flg>"
  outpmodule/981(VOUTP_HVPO120VGrpALDSt_enum) -> bus_creator/981
  outpmodule/976(VOUTP_ReqOBCV2LEna_enum) -> bus_creator/976
  outpmodule/829(VOUTP_RRBatWarn_flg) -> bus_creator/829
  outpmodule/977(VOUTP_ReqV2LIVIPopup_enum) -> bus_creator/977
  outpmodule/610(VOUTP_CarModel1_cnt) -> bus_creator/610
  outpmodule/971(VOUTP_VehActSpd_kph) -> bus_creator/971
  outpmodule/968(VOUTP_SpdCtrlMode_enum) -> bus_creator/968
  outpmodule/966(VOUTP_SaveRegenMode_enum) -> bus_creator/966
  outpmodule/964(VOUTP_IVIPwrLockSta_enum) -> bus_creator/964
  outpmodule/963(VOUTP_ActParkRequest_flg) -> bus_creator/963
  outpmodule/959(VOUTP_ReBrakeLPReq_flg) -> bus_creator/959
  outpmodule/954(VOUTP_FrUdcMax_V) -> bus_creator/954
  bus_selector12/92 -> outpmodule/917(VTPM_WritingCnt_enum)  "<VTPM_WritingCnt_enum>"
  bus_selector11/126 -> outpmodule/775(VTHC_FDCTHCREVentZStaSet5_enum)  "<VTHC_FDCTHCREVentZStaSet5_enum>"
  outpmodule/953(VOUTP_FrUdcMin_V) -> bus_creator/953
  outpmodule/951(VOUTP_FrIdcMin_A) -> bus_creator/951
  bus_selector12/30 -> outpmodule/855(VTPM_LRWheelTmpIndi_flg)  "<VTPM_LRWheelTmpIndi_flg>"
  outpmodule/949(VOUTP_FrRgnPermSta_flg) -> bus_creator/949
  outpmodule/568(VOUTP_PowerSta_enum) -> bus_creator/568
  bus_selector13/22 -> outpmodule/944(VTQD_FrEDUAvailBrkRgnTqV_flg)  "<VTQD_FrEDUAvailBrkRgnTqV_flg>"
  outpmodule/569(VOUTP_LVPwrSta_flg) -> bus_creator/569
  outpmodule/653(VOUTP_FDSOV3Cmd_flg) -> bus_creator/653
  outpmodule/566(VOUTP_HVBatCnctReq_flg) -> bus_creator/566
  outpmodule/574(VOUTP_DrivetrainSelect_enum) -> bus_creator/574
  outpmodule/565(VOUTP_DCDCVoltSetpoint_V) -> bus_creator/565
  outpmodule/563(VOUTP_ActiveDischargeReq_flg) -> bus_creator/563
  outpmodule/560(VOUTP_PowerDownState_enum) -> bus_creator/560
  outpmodule/562(VOUTP_PowerDownFault_enum) -> bus_creator/562
  outpmodule/559(VOUTP_PowerUpState_enum) -> bus_creator/559
  outpmodule/556(VOUTP_ActiveWU_flg) -> bus_creator/556
  outpmodule/557(VOUTP_SysNMmSta_enum) -> bus_creator/557
  outpmodule/558(VOUTP_NetworkReq_flg) -> bus_creator/558
  outpmodule/823(VOUTP_FDCFGSFuncSta_flg) -> bus_creator/823
  outpmodule/554(VOUTP_RptMsgReq_flg) -> bus_creator/554
  outpmodule/553(VOUTP_PNI_flg) -> bus_creator/553
  outpmodule/549(VOUTP_Awake_enum) -> bus_creator/549
  outpmodule/545(VOUTP_DISCSta_enum) -> bus_creator/545
  outpmodule/542(VOUTP_FDCDKCAllowSleep_flg) -> bus_creator/542
  outpmodule/539(VOUTP_ParkingModeCmd_enum) -> bus_creator/539
  outpmodule/538(VOUTP_DkeyAreaRAPSSta_enum) -> bus_creator/538
  outpmodule/533(VOUTP_PCommandToBCM_enum) -> bus_creator/533
  outpmodule/534(VOUTP_DKeyWelcomeSta_enum) -> bus_creator/534
  outpmodule/530(VOUTP_DkeyShowIVISta_enum) -> bus_creator/530
  bus_selector12/17 -> outpmodule/842(VTPM_LFWheelDebug_flg)  "<VTPM_LFWheelDebug_flg>"
  outpmodule/528(VOUTP_KeyMissSta_flg) -> bus_creator/528
  outpmodule/519(VOUTP_ActAPSPosn_pct) -> bus_creator/519
  outpmodule/518(VOUTP_CAN6BusOffDTC_raw32) -> bus_creator/518
  outpmodule/768(VOUTP_FDCTHCCLEVentZStaSet4_enum) -> bus_creator/768
  outpmodule/516(VOUTP_CAN4BusOffDTC_raw32) -> bus_creator/516
  outpmodule/880(VOUTP_FAT_flg) -> bus_creator/880
  outpmodule/967(VOUTP_FDCVCURegenMode_enum) -> bus_creator/967
  outpmodule/515(VOUTP_CAN3BusOffDTC_raw32) -> bus_creator/515
  outpmodule/513(VOUTP_CAN1BusOffDTC_raw32) -> bus_creator/513
  outpmodule/512(VOUTP_CAN6BusErrorDTC_raw32) -> bus_creator/512
  outpmodule/511(VOUTP_CAN5BusErrorDTC_raw32) -> bus_creator/511
  outpmodule/510(VOUTP_CAN4BusErrorDTC_raw32) -> bus_creator/510
  outpmodule/502(VOUTP_VCURLDoorSta_flg) -> bus_creator/502
  outpmodule/501(VOUTP_VCUFRDoorSta_flg) -> bus_creator/501
  outpmodule/499(VOUTP_VCUBrkSWSta_enum) -> bus_creator/499
  outpmodule/498(VOUTP_MCUActDisFail_flg) -> bus_creator/498
  outpmodule/571(VOUTP_SysPowerMode_enum) -> bus_creator/571
  outpmodule/570(VOUTP_HVPwrSta_flg) -> bus_creator/570
  outpmodule/961(VOUTP_EquivAccPedalSWSta_flg) -> bus_creator/961
  outpmodule/989(VOUTP_VMCCCCtrlAvail_flg) -> bus_creator/989
  outpmodule/1069(VOUTP_ACCPedalOvrd_flg) -> bus_creator/1069
  outpmodule/1095(VOUTP_FDCVMCDrInpTqBstAct_flg) -> bus_creator/1095
  outpmodule/1092(VOUTP_FDCVMCAPSAngleTarget_deg) -> bus_creator/1092
  bus_selector13/26 -> outpmodule/948(VTQD_PTCSPermSta_flg)  "<VTQD_PTCSPermSta_flg>"
  outpmodule/1091(VOUTP_FDCVMCAPSVRqEPSCtrl_flg) -> bus_creator/1091
  bus_selector12/8 -> outpmodule/833(VTPM_RRWheelPress_raw8)  "<VTPM_RRWheelPress_raw8>"
  outpmodule/1090(VOUTP_CalibratedGyroZ_Dps) -> bus_creator/1090
  outpmodule/384(VOUTP_HVRlyCloDTC_raw32) -> bus_creator/384
  outpmodule/1088(VOUTP_CalibratedGyroX_Dps) -> bus_creator/1088
  outpmodule/1089(VOUTP_CalibratedGyroY_Dps) -> bus_creator/1089
  outpmodule/1087(VOUTP_CalibratedAccZ_G) -> bus_creator/1087
  outpmodule/1086(VOUTP_CalibratedAccY_G) -> bus_creator/1086
  outpmodule/309(VOUTP_LockSettingStaMem_enum) -> bus_creator/309
  outpmodule/711(VOUTP_FDCTHCCLVentENSta_flg) -> bus_creator/711
  outpmodule/1014(VOUTP_ADASAEBReq_enum) -> bus_creator/1014
  outpmodule/1012(VOUTP_LKATOIFault_flg) -> bus_creator/1012
  outpmodule/1013(VOUTP_LKATOIAct_enum) -> bus_creator/1013
  outpmodule/660(VOUTP_CoolgFanActDuty_pct) -> bus_creator/660
  outpmodule/1009(VOUTP_LateralCtrl_flg) -> bus_creator/1009
  outpmodule/761(VOUTP_FDCTHCLEVentZStaSet3_enum) -> bus_creator/761
  outpmodule/1011(VOUTP_LKAStrToqReq_Nm) -> bus_creator/1011
  bus_selector11/158 -> outpmodule/807(VTHC_SettempZon1Set1_enum)  "<VTHC_SettempZon1Set1_enum>"
  outpmodule/1008(VOUTP_ActACCRequiredAccel_mps2) -> bus_creator/1008
  outpmodule/1005(VOUTP_ACCRequiredAccel_mps2) -> bus_creator/1005
  outpmodule/88(VOUTP_ShifterHandleCmdTimeOut_flg) -> bus_creator/88
  outpmodule/962(VOUTP_DriveProtEn_flg) -> bus_creator/962
  outpmodule/86(VOUTP_RRPulseCountTimeOut_flg) -> bus_creator/86
  outpmodule/89(VOUTP_DriIntend_enum) -> bus_creator/89
  bus_selector11/165 -> outpmodule/814(VTHC_ACModeSet457_enum)  "<VTHC_ACModeSet457_enum>"
  outpmodule/370(VOUTP_C1ABM1RCDTC_raw32) -> bus_creator/370
  bus_selector3/76 -> outpmodule/254(VBCM_PTGInnerSW2_enum)  "<VBCM_PTGInnerSW2_enum>"
  bus_selector3/71 -> outpmodule/249(VBCM_CountAlarm_enum)  "<VBCM_CountAlarm_enum>"
  bus_selector12/56 -> outpmodule/881(VTPM_IDin_raw32)  "<VTPM_IDin_raw32>"
  bus_selector3/70 -> outpmodule/248(VBCM_IVIRST_flg)  "<VBCM_IVIRST_flg>"
  bus_selector3/69 -> outpmodule/247(VBCM_FollowMe_flg)  "<VBCM_FollowMe_flg>"
  bus_selector3/67 -> outpmodule/245(VBCM_SPTGDet_flg)  "<VBCM_SPTGDet_flg>"
  outpmodule/427(VOUTP_RMRUSSDTC_raw32) -> bus_creator/427
  outpmodule/1007(VOUTP_FeatArbitrFinal_enum) -> bus_creator/1007
  bus_selector4/64 -> outpmodule/421(VDDM_FCLUSSDTC_raw32)  "<VDDM_FCLUSSDTC_raw32>"
  outpmodule/495(VOUTP_EDriveSysErrShifterErr_flg) -> bus_creator/495
  bus_selector4/62 -> outpmodule/419(VDDM_DiagRLTSDTC_raw32)  "<VDDM_DiagRLTSDTC_raw32>"
  outpmodule/536(VOUTP_KeyAreaSPTGSta_enum) -> bus_creator/536
  outpmodule/529(VOUTP_KeyModeSta_enum) -> bus_creator/529
  bus_selector4/60 -> outpmodule/417(VDDM_DiagFLTSDTC_raw32)  "<VDDM_DiagFLTSDTC_raw32>"
  bus_selector4/108 -> outpmodule/465(VDDM_ESC5CSErrDTC_raw32)  "<VDDM_ESC5CSErrDTC_raw32>"
  bus_selector11/167 -> outpmodule/816(VTHC_FOOTSet_enum)  "<VTHC_FOOTSet_enum>"
  bus_selector4/107 -> outpmodule/464(VDDM_ESC5RCErrDTC_raw32)  "<VDDM_ESC5RCErrDTC_raw32>"
  bus_selector4/106 -> outpmodule/463(VDDM_ESC1CSErrDTC_raw32)  "<VDDM_ESC1CSErrDTC_raw32>"
  bus_selector4/105 -> outpmodule/462(VDDM_ESC1RCErrDTC_raw32)  "<VDDM_ESC1RCErrDTC_raw32>"
  bus_selector4/104 -> outpmodule/461(VDDM_ESC7CSErrDTC_raw32)  "<VDDM_ESC7CSErrDTC_raw32>"
  bus_selector4/99 -> outpmodule/456(VDDM_MCUF1CSErrDTC_raw32)  "<VDDM_MCUF1CSErrDTC_raw32>"
  bus_selector4/100 -> outpmodule/457(VDDM_MCUR1CSErrDTC_raw32)  "<VDDM_MCUR1CSErrDTC_raw32>"
  bus_selector4/95 -> outpmodule/452(VDDM_MSAMalfuncDetDTC_raw32)  "<VDDM_MSAMalfuncDetDTC_raw32>"
  bus_selector4/94 -> outpmodule/451(VDDM_CCMalfuncDetDTC_raw32)  "<VDDM_CCMalfuncDetDTC_raw32>"
  outpmodule/683(VOUTP_sigClntTHvBattIn_C) -> bus_creator/683
  bus_selector4/97 -> outpmodule/454(VDDM_MCUF1RCErrDTC_raw32)  "<VDDM_MCUF1RCErrDTC_raw32>"
  bus_selector4/91 -> outpmodule/448(VDDM_CCUSigErrDetDTC_raw32)  "<VDDM_CCUSigErrDetDTC_raw32>"
  bus_selector4/89 -> outpmodule/446(VDDM_FrMCUSigErrDetDTC_raw32)  "<VDDM_FrMCUSigErrDetDTC_raw32>"
  outpmodule/550(VOUTP_CSB_flg) -> bus_creator/550
  bus_selector4/88 -> outpmodule/445(VDDM_FCMACCSigErrDetDTC_raw32)  "<VDDM_FCMACCSigErrDetDTC_raw32>"
  outpmodule/759(VOUTP_FDCTHCLEVentZStaSet1_enum) -> bus_creator/759
  bus_selector4/87 -> outpmodule/444(VDDM_BMSSigErrDetDTC_raw32)  "<VDDM_BMSSigErrDetDTC_raw32>"
  bus_selector4/86 -> outpmodule/443(VDDM_ZoneSCPNoComDTC_raw32)  "<VDDM_ZoneSCPNoComDTC_raw32>"
  bus_selector4/84 -> outpmodule/441(VDDM_FCM5NoComDTC_raw32)  "<VDDM_FCM5NoComDTC_raw32>"
  bus_selector12/82 -> outpmodule/907(VTPM_Flashchkdatavalid_enum)  "<VTPM_Flashchkdatavalid_enum>"
  bus_selector4/85 -> outpmodule/442(VDDM_FCM5CSErrDTC_raw32)  "<VDDM_FCM5CSErrDTC_raw32>"
  bus_selector4/83 -> outpmodule/440(VDDM_FCM4CSErrDTC_raw32)  "<VDDM_FCM4CSErrDTC_raw32>"
  bus_selector4/80 -> outpmodule/437(VDDM_FCM3RCErrDTC_raw32)  "<VDDM_FCM3RCErrDTC_raw32>"
  outpmodule/1070(VOUTP_TimeGapCalcu_s) -> bus_creator/1070
  bus_selector4/79 -> outpmodule/436(VDDM_FCM3NoComDTC_raw32)  "<VDDM_FCM3NoComDTC_raw32>"
  bus_selector4/77 -> outpmodule/434(VDDM_FCM2RCErrDTC_raw32)  "<VDDM_FCM2RCErrDTC_raw32>"
  bus_selector4/74 -> outpmodule/431(VDDM_RLLUSSDTC_raw32)  "<VDDM_RLLUSSDTC_raw32>"
  outpmodule/678(VOUTP_sigRecircSt_flg) -> bus_creator/678
  bus_selector4/73 -> outpmodule/430(VDDM_FLRUSSDTC_raw32)  "<VDDM_FLRUSSDTC_raw32>"
  bus_selector4/72 -> outpmodule/429(VDDM_FLLUSSDTC_raw32)  "<VDDM_FLLUSSDTC_raw32>"
  bus_selector4/63 -> outpmodule/420(VDDM_DiagRRTSDTC_raw32)  "<VDDM_DiagRRTSDTC_raw32>"
  bus_selector4/71 -> outpmodule/428(VDDM_RCRUSSDTC_raw32)  "<VDDM_RCRUSSDTC_raw32>"
  bus_selector4/67 -> outpmodule/424(VDDM_FCRUSSDTC_raw32)  "<VDDM_FCRUSSDTC_raw32>"
  bus_selector4/68 -> outpmodule/425(VDDM_RCLUSSDTC_raw32)  "<VDDM_RCLUSSDTC_raw32>"
  bus_selector4/69 -> outpmodule/426(VDDM_RMLUSSDTC_raw32)  "<VDDM_RMLUSSDTC_raw32>"
  bus_selector4/66 -> outpmodule/423(VDDM_FMRUSSDTC_raw32)  "<VDDM_FMRUSSDTC_raw32>"
  bus_selector12/4 -> outpmodule/829(VTPM_RRBatWarn_flg)  "<VTPM_RRBatWarn_flg>"
  bus_selector4/65 -> outpmodule/422(VDDM_FMLUSSDTC_raw32)  "<VDDM_FMLUSSDTC_raw32>"
  bus_selector11/7 -> outpmodule/656(VTHC_FDSOTXVCmd_flg)  "<VTHC_FDSOTXVCmd_flg>"
  bus_selector12/52 -> outpmodule/877(VTPM_RFP20_raw8)  "<VTPM_RFP20_raw8>"
  bus_selector11/6 -> outpmodule/655(VTHC_FDEXV2Cmd_step)  "<VTHC_FDEXV2Cmd_step>"
  bus_selector11/133 -> outpmodule/782(VTHC_FDCTHCCREVentZStaSet7_enum)  "<VTHC_FDCTHCCREVentZStaSet7_enum>"
  outpmodule/561(VOUTP_PowerUpFault_enum) -> bus_creator/561
  bus_selector11/5 -> outpmodule/654(VTHC_FDEXV1Cmd_step)  "<VTHC_FDEXV1Cmd_step>"
  bus_selector11/4 -> outpmodule/653(VTHC_FDSOV3Cmd_flg)  "<VTHC_FDSOV3Cmd_flg>"
  bus_selector11/3 -> outpmodule/652(VTHC_FDSOV2Cmd_flg)  "<VTHC_FDSOV2Cmd_flg>"
  bus_selector11/2 -> outpmodule/651(VTHC_FDSOV1Cmd_flg)  "<VTHC_FDSOV1Cmd_flg>"
  bus_selector11/1 -> outpmodule/650(VTHC_FDCompCmd_rpm)  "<VTHC_FDCompCmd_rpm>"
  outpmodule/296(VOUTP_TurnSwTSetSta_enum) -> bus_creator/296
  outpmodule/702(VOUTP_FDCTHCLEVentModeSta_enum) -> bus_creator/702
  bus_selector11/99 -> outpmodule/748(VTHC_FDCFGSChStaSet457_enum)  "<VTHC_FDCFGSChStaSet457_enum>"
  bus_selector11/97 -> outpmodule/746(VTHC_IONSWStaSet_enum)  "<VTHC_IONSWStaSet_enum>"
  outpmodule/996(VOUTP_RearWhlSlipRatioCtrl_flg) -> bus_creator/996
  bus_selector11/98 -> outpmodule/747(VTHC_FDCFGSChStaSet123_enum)  "<VTHC_FDCFGSChStaSet123_enum>"
  outpmodule/500(VOUTP_VCUFLDoorSta_flg) -> bus_creator/500
  bus_selector11/93 -> outpmodule/742(VTHC_AirIntenZone3MSet3_enum)  "<VTHC_AirIntenZone3MSet3_enum>"
  outpmodule/476(VOUTP_LFWheelTmpHighDTC_raw32) -> bus_creator/476
  bus_selector11/95 -> outpmodule/744(VTHC_AirIntenZone3MSet5_enum)  "<VTHC_AirIntenZone3MSet5_enum>"
  bus_selector11/92 -> outpmodule/741(VTHC_AirIntenZone3MSet2_enum)  "<VTHC_AirIntenZone3MSet2_enum>"
  bus_selector11/91 -> outpmodule/740(VTHC_AirIntenZone3MSet1_enum)  "<VTHC_AirIntenZone3MSet1_enum>"
  outpmodule/624(VOUTP_Dash1_cnt) -> bus_creator/624
  bus_selector11/86 -> outpmodule/735(VTHC_AirIntenZone1MSet2_enum)  "<VTHC_AirIntenZone1MSet2_enum>"
  bus_selector11/87 -> outpmodule/736(VTHC_AirIntenZone1MSet3_enum)  "<VTHC_AirIntenZone1MSet3_enum>"
  outpmodule/809(VOUTP_SettempZon1Set3_enum) -> bus_creator/809
  outpmodule/567(VOUTP_HVSysReadyToCharge_enum) -> bus_creator/567
  bus_selector11/89 -> outpmodule/738(VTHC_AirIntenZone1MSet5_enum)  "<VTHC_AirIntenZone1MSet5_enum>"
  bus_selector11/88 -> outpmodule/737(VTHC_AirIntenZone1MSet4_enum)  "<VTHC_AirIntenZone1MSet4_enum>"
  bus_selector11/84 -> outpmodule/733(VTHC_RecyAutoSet_enum)  "<VTHC_RecyAutoSet_enum>"
  bus_selector3/72 -> outpmodule/250(VBCM_MFSWTri_flg)  "<VBCM_MFSWTri_flg>"
  bus_selector11/85 -> outpmodule/734(VTHC_AirIntenZone1MSet1_enum)  "<VTHC_AirIntenZone1MSet1_enum>"
  bus_selector11/82 -> outpmodule/731(VTHC_CCUSyncStsSet_enum)  "<VTHC_CCUSyncStsSet_enum>"
  bus_selector12/95 -> outpmodule/920(VTPM_TPMSSensorIDRegStart_flg)  "<VTPM_TPMSSensorIDRegStart_flg>"
  outpmodule/541(VOUTP_KeyTypeSta_enum) -> bus_creator/541
  outpmodule/1010(VOUTP_ADASLKASta_enum) -> bus_creator/1010
  bus_selector12/43 -> outpmodule/868(VTPM_S2ID_raw32)  "<VTPM_S2ID_raw32>"
  bus_selector11/80 -> outpmodule/729(VTHC_FootMSet_enum)  "<VTHC_FootMSet_enum>"
  bus_selector11/77 -> outpmodule/726(VTHC_EWPBUflag2_flg)  "<VTHC_EWPBUflag2_flg>"
  outpmodule/517(VOUTP_CAN5BusOffDTC_raw32) -> bus_creator/517
  bus_selector2/104 -> outpmodule/107(VAPM_LatAccel_Gps)  "<VAPM_LatAccel_Gps>"
  bus_selector11/78 -> outpmodule/727(VTHC_EWPBUflag3_flg)  "<VTHC_EWPBUflag3_flg>"
  bus_selector11/74 -> outpmodule/723(VTHC_FDCFGSIONCmd_flg)  "<VTHC_FDCFGSIONCmd_flg>"
  outpmodule/307(VOUTP_WalkOutLkENMem_enum) -> bus_creator/307
  bus_selector11/76 -> outpmodule/725(VTHC_EWPBUflag1_flg)  "<VTHC_EWPBUflag1_flg>"
  bus_selector11/72 -> outpmodule/721(VTHC_FDCFGSChCmd_enum)  "<VTHC_FDCFGSChCmd_enum>"
  bus_selector11/71 -> outpmodule/720(VTHC_FDCFGSFuncSta_enum)  "<VTHC_FDCFGSFuncSta_enum>"
  bus_selector11/169 -> outpmodule/818(VTHC_LVentEN_flg)  "<VTHC_LVentEN_flg>"
  bus_selector11/73 -> outpmodule/722(VTHC_FDCFGSIONSWSta_flg)  "<VTHC_FDCFGSIONSWSta_flg>"
  outpmodule/771(VOUTP_FDCTHCREVentZStaSet1_enum) -> bus_creator/771
  bus_selector11/69 -> outpmodule/718(VTHC_FDCFGSChSta_enum)  "<VTHC_FDCFGSChSta_enum>"
  bus_selector11/66 -> outpmodule/715(VTHC_FDCTHCCRVentENSta_flg)  "<VTHC_FDCTHCCRVentENSta_flg>"
  bus_selector11/65 -> outpmodule/714(VTHC_FDCTHCCREVentYSta_enum)  "<VTHC_FDCTHCCREVentYSta_enum>"
  bus_selector11/64 -> outpmodule/713(VTHC_FDCTHCRVentENSta_flg)  "<VTHC_FDCTHCRVentENSta_flg>"
  bus_selector11/63 -> outpmodule/712(VTHC_FDCTHCREVentYSta_enum)  "<VTHC_FDCTHCREVentYSta_enum>"
  bus_selector11/62 -> outpmodule/711(VTHC_FDCTHCCLVentENSta_flg)  "<VTHC_FDCTHCCLVentENSta_flg>"
  bus_selector11/59 -> outpmodule/708(VTHC_FDCTHCLEVentYSta_enum)  "<VTHC_FDCTHCLEVentYSta_enum>"
  outpmodule/1083(VOUTP_CAASActive_flg) -> bus_creator/1083
  bus_selector11/58 -> outpmodule/707(VTHC_FDCTHCCREVentZSta_enum)  "<VTHC_FDCTHCCREVentZSta_enum>"
  bus_selector11/57 -> outpmodule/706(VTHC_FDCTHCREVentZSta_enum)  "<VTHC_FDCTHCREVentZSta_enum>"
  bus_selector11/56 -> outpmodule/705(VTHC_FDCTHCCLEVentZSta_enum)  "<VTHC_FDCTHCCLEVentZSta_enum>"
  bus_selector11/52 -> outpmodule/701(VTHC_FDCTHCAirIntZ3Sta_enum)  "<VTHC_FDCTHCAirIntZ3Sta_enum>"
  outpmodule/990(VOUTP_VMCMSACtrlAvail_flg) -> bus_creator/990
  bus_selector11/53 -> outpmodule/702(VTHC_FDCTHCLEVentModeSta_enum)  "<VTHC_FDCTHCLEVentModeSta_enum>"
  outpmodule/774(VOUTP_FDCTHCREVentZStaSet4_enum) -> bus_creator/774
  bus_selector11/50 -> outpmodule/699(VTHC_sigSetTempZon2StM_C)  "<VTHC_sigSetTempZon2StM_C>"
  bus_selector12/57 -> outpmodule/882(VTPM_S1WheelDebugALTU_pct)  "<VTPM_S1WheelDebugALTU_pct>"
  bus_selector11/48 -> outpmodule/697(VTHC_AirIntenZone1M_enum)  "<VTHC_AirIntenZone1M_enum>"
  bus_selector11/49 -> outpmodule/698(VTHC_fdefog_flg)  "<VTHC_fdefog_flg>"
  bus_selector11/46 -> outpmodule/695(VTHC_CCUSyncSts_flg)  "<VTHC_CCUSyncSts_flg>"
  bus_selector11/44 -> outpmodule/693(VTHC_FaceM_flg)  "<VTHC_FaceM_flg>"
  bus_selector11/45 -> outpmodule/694(VTHC_FootM_flg)  "<VTHC_FootM_flg>"
  bus_selector11/42 -> outpmodule/691(VTHC_Foot_flg)  "<VTHC_Foot_flg>"
  bus_selector12/74 -> outpmodule/899(VTPM_WriteChkLFID_raw)  "<VTPM_WriteChkLFID_raw>"
  bus_selector11/39 -> outpmodule/688(VTHC_FDRecyAutoCmd_enum)  "<VTHC_FDRecyAutoCmd_enum>"
  outpmodule/800(VOUTP_FDCTHCREVentYStaSet7_enum) -> bus_creator/800
  bus_selector11/40 -> outpmodule/689(VTHC_ACModeMem_enum)  "<VTHC_ACModeMem_enum>"
  bus_selector11/170 -> outpmodule/819(VTHC_CLVentEN_flg)  "<VTHC_CLVentEN_flg>"
  bus_selector11/41 -> outpmodule/690(VTHC_Face_flg)  "<VTHC_Face_flg>"
  outpmodule/797(VOUTP_FDCTHCREVentYStaSet3_enum) -> bus_creator/797
  bus_selector11/37 -> outpmodule/686(VTHC_sigCbnAirT_C)  "<VTHC_sigCbnAirT_C>"
  bus_selector11/32 -> outpmodule/681(VTHC_sigClntTHvBattOut_C)  "<VTHC_sigClntTHvBattOut_C>"
  bus_selector12/14 -> outpmodule/839(VTPM_RFSensorFail_flg)  "<VTPM_RFSensorFail_flg>"
  bus_selector11/31 -> outpmodule/680(VTHC_sigSetTempZon2St_C)  "<VTHC_sigSetTempZon2St_C>"
  bus_selector11/30 -> outpmodule/679(VTHC_sigSetTempZon1St_C)  "<VTHC_sigSetTempZon1St_C>"
  bus_selector11/174 -> outpmodule/823(VTHC_FDCFGSFuncSta_flg)  "<VTHC_FDCFGSFuncSta_flg>"
  bus_selector11/28 -> outpmodule/677(VTHC_sigWindDirZon1St_enum)  "<VTHC_sigWindDirZon1St_enum>"
  bus_selector11/27 -> outpmodule/676(VTHC_sigAirIntenZon1St_enum)  "<VTHC_sigAirIntenZon1St_enum>"
  bus_selector11/26 -> outpmodule/675(VTHC_CCUSyncLampSts_flg)  "<VTHC_CCUSyncLampSts_flg>"
  bus_selector11/25 -> outpmodule/674(VTHC_CCUACMaxLampSts_flg)  "<VTHC_CCUACMaxLampSts_flg>"
  bus_selector11/17 -> outpmodule/666(VTHC_FDFrRiAPTCHeatPwrCmd_W)  "<VTHC_FDFrRiAPTCHeatPwrCmd_W>"
  bus_selector11/19 -> outpmodule/668(VTHC_FDBlowerCmd_pct)  "<VTHC_FDBlowerCmd_pct>"
  bus_selector11/14 -> outpmodule/663(VTHC_FDEWP2Cmd_enum)  "<VTHC_FDEWP2Cmd_enum>"
  bus_selector11/15 -> outpmodule/664(VTHC_FDEWP3Cmd_enum)  "<VTHC_FDEWP3Cmd_enum>"
  bus_selector11/13 -> outpmodule/662(VTHC_FDEWP1Cmd_enum)  "<VTHC_FDEWP1Cmd_enum>"
  outpmodule/801(VOUTP_FDCTHCCREVentYStaSet1_enum) -> bus_creator/801
  bus_selector11/12 -> outpmodule/661(VTHC_FDAGSCmd_enum)  "<VTHC_FDAGSCmd_enum>"
  bus_selector11/10 -> outpmodule/659(VTHC_FDFrWPTCHeatPwrCmd_W)  "<VTHC_FDFrWPTCHeatPwrCmd_W>"
  outpmodule/1079(VOUTP_LongAcc_Gps) -> bus_creator/1079
  outpmodule/1078(VOUTP_APSReq_enum) -> bus_creator/1078
  outpmodule/1077(VOUTP_APSDecReq_mps2) -> bus_creator/1077
  outpmodule/1075(VOUTP_APSStaSys_enum) -> bus_creator/1075
  outpmodule/1076(VOUTP_APSDecReqA_flg) -> bus_creator/1076
  outpmodule/1074(VOUTP_APSActive_flg) -> bus_creator/1074
  outpmodule/1072(VOUTP_MSACtrlSta_enum) -> bus_creator/1072
  bus_selector4/4 -> outpmodule/361(VDDM_C3BMS1RCDTC_raw32)  "<VDDM_C3BMS1RCDTC_raw32>"
  bus_selector4/6 -> outpmodule/363(VDDM_C3BMS1LCDTC_raw32)  "<VDDM_C3BMS1LCDTC_raw32>"
  bus_selector4/5 -> outpmodule/362(VDDM_C3BMS1CSDTC_raw32)  "<VDDM_C3BMS1CSDTC_raw32>"
  bus_selector4/7 -> outpmodule/364(VDDM_C3CCU1RCDTC_raw32)  "<VDDM_C3CCU1RCDTC_raw32>"
  bus_selector4/3 -> outpmodule/360(VDDM_C3BMS6LCDTC_raw32)  "<VDDM_C3BMS6LCDTC_raw32>"
  outpmodule/1034(VOUTP_ADASFCWSta_enum) -> bus_creator/1034
  outpmodule/1036(VOUTP_ADASFltWrnReq_flg) -> bus_creator/1036
  outpmodule/1033(VOUTP_LeftTurnLightReq_flg) -> bus_creator/1033
  outpmodule/280(VOUTP_AmbColorSta3_enum) -> bus_creator/280
  outpmodule/1031(VOUTP_HazardWarningReq_flg) -> bus_creator/1031
  outpmodule/1029(VOUTP_ADASShftPosnReq_enum) -> bus_creator/1029
  outpmodule/1027(VOUTP_ADASVehSpdLim_raw32) -> bus_creator/1027
  outpmodule/1026(VOUTP_ACCComfortBandLower_mps2) -> bus_creator/1026
  outpmodule/1025(VOUTP_ACCJerkLowerLimit_mps3) -> bus_creator/1025
  outpmodule/1023(VOUTP_ACCJerkUpperLimit_mps3) -> bus_creator/1023
  outpmodule/1020(VOUTP_ACCObjDist_m) -> bus_creator/1020
  bus_selector11/172 -> outpmodule/821(VTHC_CRVentEN_flg)  "<VTHC_CRVentEN_flg>"
  outpmodule/1021(VOUTP_ACCObjRelSpd_mps) -> bus_creator/1021
  outpmodule/1019(VOUTP_ADASACCSta_enum) -> bus_creator/1019
  outpmodule/1018(VOUTP_ADASDBSReq_enum) -> bus_creator/1018
  outpmodule/90(VOUTP_DriIntendTimeOut_flg) -> bus_creator/90
  outpmodule/888(VOUTP_ID3messageALTU_raw8) -> bus_creator/888
  outpmodule/1080(VOUTP_CCMSASpdWar_flg) -> bus_creator/1080
  outpmodule/1017(VOUTP_ACCVehHoldReq_flg) -> bus_creator/1017
  outpmodule/1066(VOUTP_FCMLDWRequest_enum) -> bus_creator/1066
  outpmodule/1068(VOUTP_ACCCtrlAvail_flg) -> bus_creator/1068
  outpmodule/1065(VOUTP_ADASAEBSta_enum) -> bus_creator/1065
  outpmodule/1064(VOUTP_ADASLanecurveR_raw32) -> bus_creator/1064
  outpmodule/1063(VOUTP_ADASLanecurveL_raw32) -> bus_creator/1063
  outpmodule/1062(VOUTP_ADASLanetypeL_enum) -> bus_creator/1062
  outpmodule/1060(VOUTP_FCMACCmode_enum) -> bus_creator/1060
  outpmodule/1057(VOUTP_LVDAWarning_flg) -> bus_creator/1057
  outpmodule/1059(VOUTP_ADASLFCWarnSound_enum) -> bus_creator/1059
  outpmodule/621(VOUTP_Country1_cnt) -> bus_creator/621
  outpmodule/1049(VOUTP_ADASSLIFSta_enum) -> bus_creator/1049
  outpmodule/1046(VOUTP_ADASLFCSta_enum) -> bus_creator/1046
  outpmodule/1040(VOUTP_ADASWarningMsg_enum) -> bus_creator/1040
  bus_selector2/133 -> outpmodule/136(VAPM_EPBStaTimeOut_flg)  "<VAPM_EPBStaTimeOut_flg>"
  outpmodule/1038(VOUTP_ForceLowBeam_enum) -> bus_creator/1038
  outpmodule/1001(VOUTP_AccCalcuPID_mps2) -> bus_creator/1001
  outpmodule/1035(VOUTP_ADASLDWSta_enum) -> bus_creator/1035
  bus_selector3/50 -> outpmodule/228(VBCM_AmbLightBreath3_enum)  "<VBCM_AmbLightBreath3_enum>"
  bus_selector2/103 -> outpmodule/106(VAPM_YawRateTimeOut_flg)  "<VAPM_YawRateTimeOut_flg>"
  outpmodule/692(VOUTP_Frost_flg) -> bus_creator/692
  bus_selector3/42 -> outpmodule/220(VBCM_TailgateHDSW_flg)  "<VBCM_TailgateHDSW_flg>"
  bus_selector3/39 -> outpmodule/217(VBCM_RoomLampH_flg)  "<VBCM_RoomLampH_flg>"
  outpmodule/975(VOUTP_RrTMTqReq_Nm) -> bus_creator/975
  bus_selector4/81 -> outpmodule/438(VDDM_FCM3CSErrDTC_raw32)  "<VDDM_FCM3CSErrDTC_raw32>"
  bus_selector3/29 -> outpmodule/207(VBCM_RDRL_flg)  "<VBCM_RDRL_flg>"
  bus_selector3/65 -> outpmodule/243(VBCM_AmbLightColor6_enum)  "<VBCM_AmbLightColor6_enum>"
  bus_selector3/63 -> outpmodule/241(VBCM_AmbLightColor4_enum)  "<VBCM_AmbLightColor4_enum>"
  outpmodule/722(VOUTP_FDCFGSIONSWSta_flg) -> bus_creator/722
  bus_selector11/38 -> outpmodule/687(VTHC_ACSubMode_enum)  "<VTHC_ACSubMode_enum>"
  bus_selector3/62 -> outpmodule/240(VBCM_AmbLightColor3_enum)  "<VBCM_AmbLightColor3_enum>"
  bus_selector13/46 -> outpmodule/968(VTQD_SpdCtrlMode_enum)  "<VTQD_SpdCtrlMode_enum>"
  bus_selector13/45 -> outpmodule/967(VTQD_FDCVCURegenMode_enum)  "<VTQD_FDCVCURegenMode_enum>"
  bus_selector13/51 -> outpmodule/973(VTQD_SetSpdLimWarn_flg)  "<VTQD_SetSpdLimWarn_flg>"
  bus_selector2/72 -> outpmodule/75(VAPM_LRPulseCountV_flg)  "<VAPM_LRPulseCountV_flg>"
  bus_selector2/65 -> outpmodule/68(VAPM_LRWhlRotDirTimeOut_flg)  "<VAPM_LRWhlRotDirTimeOut_flg>"
  bus_selector2/67 -> outpmodule/70(VAPM_RRWhlRotDirTimeOut_flg)  "<VAPM_RRWhlRotDirTimeOut_flg>"
  outpmodule/855(VOUTP_LRWheelTmpIndi_flg) -> bus_creator/855
  outpmodule/358(VOUTP_C3BMS6RCDTC_raw32) -> bus_creator/358
  bus_selector12/28 -> outpmodule/853(VTPM_LFWheelTmpIndi_flg)  "<VTPM_LFWheelTmpIndi_flg>"
  bus_selector2/68 -> outpmodule/71(VAPM_LFPulseCountV_flg)  "<VAPM_LFPulseCountV_flg>"
  outpmodule/377(VOUTP_BrkSWErrDTC_raw32) -> bus_creator/377
  bus_selector2/74 -> outpmodule/77(VAPM_RRPulseCountV_flg)  "<VAPM_RRPulseCountV_flg>"
  outpmodule/1096(VOUTP_FDCVMCMaxAngCtrlOutTqLim_Nm) -> bus_creator/1096
  outpmodule/684(VOUTP_sigCbnSolarRight_W) -> bus_creator/684
  bus_selector2/73 -> outpmodule/76(VAPM_LRPulseCountVTimeOut_flg)  "<VAPM_LRPulseCountVTimeOut_flg>"
  bus_selector3/123 -> outpmodule/301(VBCM_TurnSwTimeSetSta457_enum)  "<VBCM_TurnSwTimeSetSta457_enum>"
  bus_selector12/54 -> outpmodule/879(VTPM_RRP20_raw8)  "<VTPM_RRP20_raw8>"
  outpmodule/463(VOUTP_ESC1CSErrDTC_raw32) -> bus_creator/463
  bus_selector3/122 -> outpmodule/300(VBCM_TurnSwTimeSetSta123_enum)  "<VBCM_TurnSwTimeSetSta123_enum>"
  outpmodule/277(VOUTP_AmbODAENFlash_enum) -> bus_creator/277
  bus_selector11/96 -> outpmodule/745(VTHC_AirIntenZone3MSet7_enum)  "<VTHC_AirIntenZone3MSet7_enum>"
  bus_selector3/116 -> outpmodule/294(VBCM_FWasSwSta_enum)  "<VBCM_FWasSwSta_enum>"
  bus_selector3/115 -> outpmodule/293(VBCM_FWipSwSta_enum)  "<VBCM_FWipSwSta_enum>"
  bus_selector3/112 -> outpmodule/290(VBCM_HazardIND_flg)  "<VBCM_HazardIND_flg>"
  bus_selector3/111 -> outpmodule/289(VBCM_AmbBrightnessSta7_enum)  "<VBCM_AmbBrightnessSta7_enum>"
  bus_selector3/108 -> outpmodule/286(VBCM_AmbBrightnessSta3_enum)  "<VBCM_AmbBrightnessSta3_enum>"
  outpmodule/1030(VOUTP_ADASForceIdle_flg) -> bus_creator/1030
  bus_selector3/106 -> outpmodule/284(VBCM_AmbBrightnessSta1_enum)  "<VBCM_AmbBrightnessSta1_enum>"
  bus_selector3/107 -> outpmodule/285(VBCM_AmbBrightnessSta2_enum)  "<VBCM_AmbBrightnessSta2_enum>"
  outpmodule/457(VOUTP_MCUR1CSErrDTC_raw32) -> bus_creator/457
  bus_selector3/104 -> outpmodule/282(VBCM_AmbColorSta5_enum)  "<VBCM_AmbColorSta5_enum>"
  bus_selector3/105 -> outpmodule/283(VBCM_AmbColorSta7_enum)  "<VBCM_AmbColorSta7_enum>"
  outpmodule/853(VOUTP_LFWheelTmpIndi_flg) -> bus_creator/853
  bus_selector3/101 -> outpmodule/279(VBCM_AmbColorSta2_enum)  "<VBCM_AmbColorSta2_enum>"
  outpmodule/770(VOUTP_FDCTHCCLEVentZStaSet7_enum) -> bus_creator/770
  bus_selector3/103 -> outpmodule/281(VBCM_AmbColorSta4_enum)  "<VBCM_AmbColorSta4_enum>"
  bus_selector3/97 -> outpmodule/275(VBCM_AmbLinkDriStaFlash_enum)  "<VBCM_AmbLinkDriStaFlash_enum>"
  bus_selector11/146 -> outpmodule/795(VTHC_FDCTHCREVentYStaSet1_enum)  "<VTHC_FDCTHCREVentYStaSet1_enum>"
  bus_selector3/98 -> outpmodule/276(VBCM_AmbPwrWarnENFlash_enum)  "<VBCM_AmbPwrWarnENFlash_enum>"
  bus_selector3/99 -> outpmodule/277(VBCM_AmbODAENFlash_enum)  "<VBCM_AmbODAENFlash_enum>"
  bus_selector3/96 -> outpmodule/274(VBCM_AmbDimENFlash_enum)  "<VBCM_AmbDimENFlash_enum>"
  bus_selector12/91 -> outpmodule/916(VTPM_FlashIDvalid_enum)  "<VTPM_FlashIDvalid_enum>"
  outpmodule/546(VOUTP_DISCButtSta_flg) -> bus_creator/546
  bus_selector3/93 -> outpmodule/271(VBCM_UserNow_enum)  "<VBCM_UserNow_enum>"
  bus_selector12/40 -> outpmodule/865(VTPM_LRSensorMode_flg)  "<VTPM_LRSensorMode_flg>"
  outpmodule/526(VOUTP_DKCAuthSta_enum) -> bus_creator/526
  bus_selector2/71 -> outpmodule/74(VAPM_RFPulseCountVTimeOut_flg)  "<VAPM_RFPulseCountVTimeOut_flg>"
  bus_selector3/89 -> outpmodule/267(VBCM_AmbBrightSta_enum)  "<VBCM_AmbBrightSta_enum>"
  bus_selector3/87 -> outpmodule/265(VBCM_AmbODAEN_flg)  "<VBCM_AmbODAEN_flg>"
  bus_selector3/84 -> outpmodule/262(VBCM_AmbDimEN_flg)  "<VBCM_AmbDimEN_flg>"
  bus_selector4/103 -> outpmodule/460(VDDM_ESC7RCErrDTC_raw32)  "<VDDM_ESC7RCErrDTC_raw32>"
  bus_selector3/85 -> outpmodule/263(VBCM_AmbLinkDriSta_flg)  "<VBCM_AmbLinkDriSta_flg>"
  outpmodule/494(VOUTP_VCURAPSErrLv3_flg) -> bus_creator/494
  bus_selector3/79 -> outpmodule/257(VBCM_DrRWdwCtrlCmd_pct)  "<VBCM_DrRWdwCtrlCmd_pct>"
  bus_selector11/70 -> outpmodule/719(VTHC_FDCFGSAirIntCmd_enum)  "<VTHC_FDCFGSAirIntCmd_enum>"
  bus_selector6/12 -> outpmodule/536(VDKC_KeyAreaSPTGSta_enum)  "<VDKC_KeyAreaSPTGSta_enum>"
  bus_selector13/35 -> outpmodule/957(VTQD_RrUdcMin_V)  "<VTQD_RrUdcMin_V>"
  bus_selector4/11 -> outpmodule/368(VDDM_C3CCU2CSDTC_raw32)  "<VDDM_C3CCU2CSDTC_raw32>"
  bus_selector3/124 -> outpmodule/302(VBCM_FDLHandleLampCmd_flg)  "<VBCM_FDLHandleLampCmd_flg>"
  bus_selector4/9 -> outpmodule/366(VDDM_C3CCU1LCDTC_raw32)  "<VDDM_C3CCU1LCDTC_raw32>"
  bus_selector13/34 -> outpmodule/956(VTQD_RrIdcMax_A)  "<VTQD_RrIdcMax_A>"
  bus_selector3/140 -> outpmodule/318(VBCM_UserHeightSet_cnt)  "<VBCM_UserHeightSet_cnt>"
  bus_selector3/137 -> outpmodule/315(VBCM_HoodRelCmd_flg)  "<VBCM_HoodRelCmd_flg>"
  bus_selector3/138 -> outpmodule/316(VBCM_WelcomeLight_enum)  "<VBCM_WelcomeLight_enum>"
  bus_selector11/81 -> outpmodule/730(VTHC_fdefogSet_enum)  "<VTHC_fdefogSet_enum>"
  bus_selector3/135 -> outpmodule/313(VBCM_RmLpModeENFunSta_flg)  "<VBCM_RmLpModeENFunSta_flg>"
  bus_selector3/134 -> outpmodule/312(VBCM_WalkOutLkENFunSta_flg)  "<VBCM_WalkOutLkENFunSta_flg>"
  bus_selector3/136 -> outpmodule/314(VBCM_FollowMeENFunSta_flg)  "<VBCM_FollowMeENFunSta_flg>"
  outpmodule/441(VOUTP_FCM5NoComDTC_raw32) -> bus_creator/441
  bus_selector2/88 -> outpmodule/91(VAPM_EPSAOIControl_enum)  "<VAPM_EPSAOIControl_enum>"
  bus_selector3/133 -> outpmodule/311(VBCM_WalkInUnLkENFunSta_flg)  "<VBCM_WalkInUnLkENFunSta_flg>"
  bus_selector3/132 -> outpmodule/310(VBCM_FollowMeENMem_enum)  "<VBCM_FollowMeENMem_enum>"
  bus_selector12/94 -> outpmodule/919(VTPM_LProgress_enum)  "<VTPM_LProgress_enum>"
  bus_selector3/131 -> outpmodule/309(VBCM_LockSettingStaMem_enum)  "<VBCM_LockSettingStaMem_enum>"
  bus_selector3/130 -> outpmodule/308(VBCM_RmLpModeENMem_enum)  "<VBCM_RmLpModeENMem_enum>"
  outpmodule/375(VOUTP_Lv3ErrDTC_raw32) -> bus_creator/375
  bus_selector12/44 -> outpmodule/869(VTPM_S3ID_raw32)  "<VTPM_S3ID_raw32>"
  bus_selector11/33 -> outpmodule/682(VTHC_sigCbnSolarLeft_W)  "<VTHC_sigCbnSolarLeft_W>"
  outpmodule/1039(VOUTP_ACCTakeoverReq_flg) -> bus_creator/1039
  bus_selector3/126 -> outpmodule/304(VBCM_FDHandleCmd_enum)  "<VBCM_FDHandleCmd_enum>"
  outpmodule/585(VOUTP_IVIPwrStaONTOPopT_s) -> bus_creator/585
  bus_selector4/129 -> outpmodule/486(VDDM_5vAPS2PwrErrDTC_raw32)  "<VDDM_5vAPS2PwrErrDTC_raw32>"
  BAPM_outputs/1 -> bus_selector2/1
  bus_selector4/127 -> outpmodule/484(VDDM_C1EPAS2LCDTC_raw32)  "<VDDM_C1EPAS2LCDTC_raw32>"
  bus_selector3/109 -> outpmodule/287(VBCM_AmbBrightnessSta4_enum)  "<VBCM_AmbBrightnessSta4_enum>"
  outpmodule/972(VOUTP_RegenLimIndSta_flg) -> bus_creator/972
  bus_selector4/126 -> outpmodule/483(VDDM_RRSensorFailDTC_raw32)  "<VDDM_RRSensorFailDTC_raw32>"
  bus_selector4/123 -> outpmodule/480(VDDM_LFSensorFailDTC_raw32)  "<VDDM_LFSensorFailDTC_raw32>"
  bus_selector4/120 -> outpmodule/477(VDDM_RFWheelTmpHighDTC_raw32)  "<VDDM_RFWheelTmpHighDTC_raw32>"
  bus_selector4/116 -> outpmodule/473(VDDM_RFPressIndiDTC_raw32)  "<VDDM_RFPressIndiDTC_raw32>"
  bus_selector4/115 -> outpmodule/472(VDDM_LFPressIndiDTC_raw32)  "<VDDM_LFPressIndiDTC_raw32>"
  bus_selector4/114 -> outpmodule/471(VDDM_RRBatwarnDTC_raw32)  "<VDDM_RRBatwarnDTC_raw32>"
  bus_selector4/109 -> outpmodule/466(VDDM_FrMCUTqErrDTC_raw32)  "<VDDM_FrMCUTqErrDTC_raw32>"
  outpmodule/316(VOUTP_WelcomeLight_enum) -> bus_creator/316
  bus_selector4/110 -> outpmodule/467(VDDM_RrMCUTqErrDTC_raw32)  "<VDDM_RrMCUTqErrDTC_raw32>"
  outpmodule/1085(VOUTP_CalibratedAccX_G) -> bus_creator/1085
  outpmodule/680(VOUTP_sigSetTempZon2St_C) -> bus_creator/680
  bus_selector1/3 -> outpmodule/3(VACC_VehHVPwrAvail4THCM_W)  "<VACC_VehHVPwrAvail4THCM_W>"
  outpmodule/586(VOUTP_LVChrgHoldTtimer_s) -> bus_creator/586
  bus_selector2/61 -> outpmodule/64(VAPM_LFWhlRotDirTimeOut_flg)  "<VAPM_LFWhlRotDirTimeOut_flg>"
  bus_selector2/60 -> outpmodule/63(VAPM_LFWhlRotDir_enum)  "<VAPM_LFWhlRotDir_enum>"
  bus_selector2/59 -> outpmodule/62(VAPM_RRRawWhlSpeedVTimeOut_flg)  "<VAPM_RRRawWhlSpeedVTimeOut_flg>"
  outpmodule/357(VOUTP_WinRROpenedSta_pct) -> bus_creator/357
  BACC_outputs/1 -> bus_selector1/1
  bus_selector8/5 -> outpmodule/551(VNMM_ErrorState_enum)  "<VNMM_ErrorState_enum>"
  outpmodule/671(VOUTP_CabinMode_enum) -> bus_creator/671
  bus_selector2/5 -> outpmodule/8(VAPM_ChrgPlugSta_enum)  "<VAPM_ChrgPlugSta_enum>"
  bus_selector3/31 -> outpmodule/209(VBCM_RBSD_flg)  "<VBCM_RBSD_flg>"
  bus_selector2/3 -> outpmodule/6(VAPM_FSOffSw_enum)  "<VAPM_FSOffSw_enum>"
  bus_selector11/128 -> outpmodule/777(VTHC_FDCTHCCREVentZStaSet1_enum)  "<VTHC_FDCTHCCREVentZStaSet1_enum>"
  outpmodule/1024(VOUTP_ACCComfortBandUpper_mps2) -> bus_creator/1024
  outpmodule/286(VOUTP_AmbBrightnessSta3_enum) -> bus_creator/286
  bus_selector2/1 -> outpmodule/4(VAPM_VehSpeed_kph)  "<VAPM_VehSpeed_kph>"
  bus_selector2/76 -> outpmodule/79(VAPM_LFPulseCount_enum)  "<VAPM_LFPulseCount_enum>"
  bus_selector2/80 -> outpmodule/83(VAPM_LRPulseCount_enum)  "<VAPM_LRPulseCount_enum>"
  bus_selector2/53 -> outpmodule/56(VAPM_LFRawWhlSpeedVTimeOut_flg)  "<VAPM_LFRawWhlSpeedVTimeOut_flg>"
  bus_selector4/90 -> outpmodule/447(VDDM_RrMCUSigErrDetDTC_raw32)  "<VDDM_RrMCUSigErrDetDTC_raw32>"
  outpmodule/532(VOUTP_KeyAreaLockUnlock_enum) -> bus_creator/532
  bus_selector2/54 -> outpmodule/57(VAPM_RFRawWhlSpeedV_flg)  "<VAPM_RFRawWhlSpeedV_flg>"
  bus_selector2/50 -> outpmodule/53(VAPM_RRRawWhlSpeed_kph)  "<VAPM_RRRawWhlSpeed_kph>"
  outpmodule/596(VOUTP_CtrlFrRC1_flg) -> bus_creator/596
  bus_selector12/76 -> outpmodule/901(VTPM_WriteChkLRID_raw)  "<VTPM_WriteChkLRID_raw>"
  outpmodule/781(VOUTP_FDCTHCCREVentZStaSet5_enum) -> bus_creator/781
  bus_selector2/51 -> outpmodule/54(VAPM_RRRawWhlSpeedTimeOut_flg)  "<VAPM_RRRawWhlSpeedTimeOut_flg>"
  outpmodule/349(VOUTP_PasWdwReqAP_enum) -> bus_creator/349
  bus_selector2/49 -> outpmodule/52(VAPM_LRRawWhlSpeedTimeOut_flg)  "<VAPM_LRRawWhlSpeedTimeOut_flg>"
  bus_selector2/42 -> outpmodule/45(VAPM_BrkPedalPos_pct)  "<VAPM_BrkPedalPos_pct>"
  bus_selector3/120 -> outpmodule/298(VBCM_SPTGENFunMem_enum)  "<VBCM_SPTGENFunMem_enum>"
  outpmodule/459(VOUTP_Shifter1CSErrDTC_raw32) -> bus_creator/459
  bus_selector2/40 -> outpmodule/43(VAPM_StaFSya_flg)  "<VAPM_StaFSya_flg>"
  outpmodule/456(VOUTP_MCUF1CSErrDTC_raw32) -> bus_creator/456
  bus_selector2/41 -> outpmodule/44(VAPM_ModOperation_enum)  "<VAPM_ModOperation_enum>"
  outpmodule/886(VOUTP_ID1messageALTU_raw8) -> bus_creator/886
  bus_selector2/38 -> outpmodule/41(VAPM_Chime_enum)  "<VAPM_Chime_enum>"
  bus_selector2/35 -> outpmodule/38(VAPM_USSStaFLL_flg)  "<VAPM_USSStaFLL_flg>"
  bus_selector2/28 -> outpmodule/31(VAPM_USSStaRLR_flg)  "<VAPM_USSStaRLR_flg>"
  bus_selector2/29 -> outpmodule/32(VAPM_USSStaRLL_flg)  "<VAPM_USSStaRLL_flg>"
  bus_selector2/27 -> outpmodule/30(VAPM_USSStaRML_flg)  "<VAPM_USSStaRML_flg>"
  bus_selector3/139 -> outpmodule/317(VBCM_PTGOpenHeightSta_enum)  "<VBCM_PTGOpenHeightSta_enum>"
  bus_selector2/21 -> outpmodule/24(VAPM_PASARCR_enum)  "<VAPM_PASARCR_enum>"
  outpmodule/361(VOUTP_C3BMS1RCDTC_raw32) -> bus_creator/361
  bus_selector2/45 -> outpmodule/48(VAPM_LFRawWhlSpeedTimeOut_flg)  "<VAPM_LFRawWhlSpeedTimeOut_flg>"
  bus_selector12/87 -> outpmodule/912(VTPM_FlashS1ID_raw)  "<VTPM_FlashS1ID_raw>"
  bus_selector2/17 -> outpmodule/20(VAPM_APSDFLL_cm)  "<VAPM_APSDFLL_cm>"
  bus_selector2/19 -> outpmodule/22(VAPM_PASARMR_enum)  "<VAPM_PASARMR_enum>"
  outpmodule/346(VOUTP_HMIKey8FuncSta_enum) -> bus_creator/346
  outpmodule/846(VOUTP_TPMSResButtAllow_flg) -> bus_creator/846
  bus_selector2/18 -> outpmodule/21(VAPM_PASAFCL_enum)  "<VAPM_PASAFCL_enum>"
  outpmodule/640(VOUTP_WisrBootReason_raw32) -> bus_creator/640
  bus_selector2/13 -> outpmodule/16(VAPM_PASDFCL_cm)  "<VAPM_PASDFCL_cm>"
  bus_selector2/14 -> outpmodule/17(VAPM_APSDRLR_cm)  "<VAPM_APSDRLR_cm>"
  bus_selector2/11 -> outpmodule/14(VAPM_PASDFML_cm)  "<VAPM_PASDFML_cm>"
  outpmodule/1073(VOUTP_APSCtrlAvail_flg) -> bus_creator/1073
  bus_selector3/88 -> outpmodule/266(VBCM_AmbColorSta_enum)  "<VBCM_AmbColorSta_enum>"
  outpmodule/393(VOUTP_OBC4PreDTC_raw32) -> bus_creator/393
  outpmodule/979(VOUTP_ReqOBCExtrV2LEna_enum) -> bus_creator/979
  bus_selector2/8 -> outpmodule/11(VAPM_PASDRCR_cm)  "<VAPM_PASDRCR_cm>"
  bus_selector3/102 -> outpmodule/280(VBCM_AmbColorSta3_enum)  "<VBCM_AmbColorSta3_enum>"
  outpmodule/269(VOUTP_ATCtrl_enum) -> bus_creator/269
  bus_selector2/9 -> outpmodule/12(VAPM_PASDRCL_cm)  "<VAPM_PASDRCL_cm>"
  outpmodule/1041(VOUTP_ADASCAMSpdLim_enum) -> bus_creator/1041
  bus_selector2/7 -> outpmodule/10(VAPM_PASDRML_cm)  "<VAPM_PASDRML_cm>"
  bus_selector2/47 -> outpmodule/50(VAPM_RFRawWhlSpeedTimeOut_flg)  "<VAPM_RFRawWhlSpeedTimeOut_flg>"
  bus_selector9/20 -> outpmodule/578(VPMM_TCountSta_enum)  "<VPMM_TCountSta_enum>"
  bus_selector11/173 -> outpmodule/822(VTHC_FDCFGSLearnCmd_enum)  "<VTHC_FDCFGSLearnCmd_enum>"
  outpmodule/548(VOUTP_NMmTxReq_flg) -> bus_creator/548
  outpmodule/609(VOUTP_HWVer3_cnt) -> bus_creator/609
  bus_selector9/19 -> outpmodule/577(VPMM_PwrStaConstraint_enum)  "<VPMM_PwrStaConstraint_enum>"
  bus_selector9/17 -> outpmodule/575(VPMM_DrSeatSta_enum)  "<VPMM_DrSeatSta_enum>"
  bus_selector9/15 -> outpmodule/573(VPMM_RrMCUEnaReq_flg)  "<VPMM_RrMCUEnaReq_flg>"
  outpmodule/1054(VOUTP_LVDADisabled_flg) -> bus_creator/1054
  bus_selector9/13 -> outpmodule/571(VPMM_SysPowerMode_enum)  "<VPMM_SysPowerMode_enum>"
  bus_selector9/7 -> outpmodule/565(VPMM_DCDCVoltSetpoint_V)  "<VPMM_DCDCVoltSetpoint_V>"
  outpmodule/664(VOUTP_FDEWP3Cmd_enum) -> bus_creator/664
  bus_selector4/130 -> outpmodule/487(VDDM_EPBLockTODTC_raw32)  "<VDDM_EPBLockTODTC_raw32>"
  bus_selector9/5 -> outpmodule/563(VPMM_ActiveDischargeReq_flg)  "<VPMM_ActiveDischargeReq_flg>"
  bus_selector9/1 -> outpmodule/559(VPMM_PowerUpState_enum)  "<VPMM_PowerUpState_enum>"
  bus_selector2/10 -> outpmodule/13(VAPM_PASDFMR_cm)  "<VAPM_PASDFMR_cm>"
  outpmodule/902(VOUTP_WriteChkRRID_raw) -> bus_creator/902
  bus_selector9/3 -> outpmodule/561(VPMM_PowerUpFault_enum)  "<VPMM_PowerUpFault_enum>"
  bus_selector13/50 -> outpmodule/972(VTQD_RegenLimIndSta_flg)  "<VTQD_RegenLimIndSta_flg>"
  bus_selector9/29 -> outpmodule/587(VPMM_LVBattChrgTimeCnt_s)  "<VPMM_LVBattChrgTimeCnt_s>"
  outpmodule/672(VOUTP_CCUACLampSts_flg) -> bus_creator/672
  bus_selector11/156 -> outpmodule/805(VTHC_FDCTHCCREVentYStaSet5_enum)  "<VTHC_FDCTHCCREVentYStaSet5_enum>"
  bus_selector9/27 -> outpmodule/585(VPMM_IVIPwrStaONTOPopT_s)  "<VPMM_IVIPwrStaONTOPopT_s>"
  bus_selector3/34 -> outpmodule/212(VBCM_RTurnLP_flg)  "<VBCM_RTurnLP_flg>"
  bus_selector9/28 -> outpmodule/586(VPMM_LVChrgHoldTtimer_s)  "<VPMM_LVChrgHoldTtimer_s>"
  bus_selector2/81 -> outpmodule/84(VAPM_LRPulseCountTimeOut_flg)  "<VAPM_LRPulseCountTimeOut_flg>"
  bus_selector2/120 -> outpmodule/123(VAPM_BrkSwV_flg)  "<VAPM_BrkSwV_flg>"
  bus_selector4/98 -> outpmodule/455(VDDM_MCUR1RCErrDTC_raw32)  "<VDDM_MCUR1RCErrDTC_raw32>"
  bus_selector2/34 -> outpmodule/37(VAPM_USSStaFLR_flg)  "<VAPM_USSStaFLR_flg>"
  bus_selector13/30 -> outpmodule/952(VTQD_FrIdcMax_A)  "<VTQD_FrIdcMax_A>"
  bus_selector3/7 -> outpmodule/185(VBCM_HoodSW_flg)  "<VBCM_HoodSW_flg>"
  bus_selector3/16 -> outpmodule/194(VBCM_CrashDetd_flg)  "<VBCM_CrashDetd_flg>"
  bus_selector13/3 -> outpmodule/925(VTQD_TqSourceRr_enum)  "<VTQD_TqSourceRr_enum>"
  bus_selector3/6 -> outpmodule/184(VBCM_AntitheftSeatFlod_flg)  "<VBCM_AntitheftSeatFlod_flg>"
  outpmodule/369(VOUTP_C3CCU2LCDTC_raw32) -> bus_creator/369
  bus_selector2/30 -> outpmodule/33(VAPM_USSStaRCR_flg)  "<VAPM_USSStaRCR_flg>"
  bus_selector3/5 -> outpmodule/183(VBCM_BCMDoorLockSta_flg)  "<VBCM_BCMDoorLockSta_flg>"
  outpmodule/898(VOUTP_RRPindi_enum) -> bus_creator/898
  bus_selector11/79 -> outpmodule/728(VTHC_FaceMSet_enum)  "<VTHC_FaceMSet_enum>"
  outpmodule/256(VOUTP_PasWdwCtrlCmd_pct) -> bus_creator/256
  bus_selector3/3 -> outpmodule/181(VBCM_HornCtrl_flg)  "<VBCM_HornCtrl_flg>"
  bus_selector3/56 -> outpmodule/234(VBCM_AmbLightBrightness3_enum)  "<VBCM_AmbLightBrightness3_enum>"
  bus_selector11/55 -> outpmodule/704(VTHC_FDCTHCLEVentZSta_enum)  "<VTHC_FDCTHCLEVentZSta_enum>"
  bus_selector2/22 -> outpmodule/25(VAPM_PASARCL_enum)  "<VAPM_PASARCL_enum>"
  bus_selector3/58 -> outpmodule/236(VBCM_AmbLightBrightness5_enum)  "<VBCM_AmbLightBrightness5_enum>"
  bus_selector3/2 -> outpmodule/180(VBCM_TailgateRemote_enum)  "<VBCM_TailgateRemote_enum>"
  bus_selector3/1 -> outpmodule/179(VBCM_AntitheftSta_enum)  "<VBCM_AntitheftSta_enum>"
  bus_selector13/40 -> outpmodule/962(VTQD_DriveProtEn_flg)  "<VTQD_DriveProtEn_flg>"
  bus_selector2/149 -> outpmodule/152(VAPM_ABSActiveTimeOut_flg)  "<VAPM_ABSActiveTimeOut_flg>"
  outpmodule/907(VOUTP_Flashchkdatavalid_enum) -> bus_creator/907
  bus_selector2/148 -> outpmodule/151(VAPM_ABSActive_flg)  "<VAPM_ABSActive_flg>"
  bus_selector2/147 -> outpmodule/150(VAPM_IVIScreenTimeOut_flg)  "<VAPM_IVIScreenTimeOut_flg>"
  bus_selector2/146 -> outpmodule/149(VAPM_IVIScreen_enum)  "<VAPM_IVIScreen_enum>"
  outpmodule/808(VOUTP_SettempZon1Set2_enum) -> bus_creator/808
  bus_selector2/145 -> outpmodule/148(VAPM_CAASSwTimeOut_flg)  "<VAPM_CAASSwTimeOut_flg>"
  outpmodule/1082(VOUTP_CAASCtrlAvail_flg) -> bus_creator/1082
  outpmodule/289(VOUTP_AmbBrightnessSta7_enum) -> bus_creator/289
  bus_selector3/118 -> outpmodule/296(VBCM_TurnSwTSetSta_enum)  "<VBCM_TurnSwTSetSta_enum>"
  outpmodule/740(VOUTP_AirIntenZone3MSet1_enum) -> bus_creator/740
  outpmodule/332(VOUTP_ACCLevelMem57_enum) -> bus_creator/332
  bus_selector2/143 -> outpmodule/146(VAPM_IVIStatusTimeOut_flg)  "<VAPM_IVIStatusTimeOut_flg>"
  bus_selector2/64 -> outpmodule/67(VAPM_LRWhlRotDir_enum)  "<VAPM_LRWhlRotDir_enum>"
  bus_selector2/142 -> outpmodule/145(VAPM_IVIStatus_flg)  "<VAPM_IVIStatus_flg>"
  bus_selector2/139 -> outpmodule/142(VAPM_AVMParkingmodeTimeOut_flg)  "<VAPM_AVMParkingmodeTimeOut_flg>"
  outpmodule/291(VOUTP_DimSwSta_flg) -> bus_creator/291
  bus_selector2/174 -> outpmodule/177(VAPM_RAPSErrLv1_flg)  "<VAPM_RAPSErrLv1_flg>"
  bus_selector2/175 -> outpmodule/178(VAPM_IVIUserTakeOverAPSSta_flg)  "<VAPM_IVIUserTakeOverAPSSta_flg>"
  bus_selector2/172 -> outpmodule/175(VAPM_APSPwrReq_enum)  "<VAPM_APSPwrReq_enum>"
  outpmodule/572(VOUTP_FrMCUEnaReq_flg) -> bus_creator/572
  outpmodule/1055(VOUTP_LVDAMuteSta_enum) -> bus_creator/1055
  bus_selector2/173 -> outpmodule/176(VAPM_RAPSErrWarnSta_enum)  "<VAPM_RAPSErrWarnSta_enum>"
  bus_selector2/168 -> outpmodule/171(VAPM_APSSpeedCMD_kph)  "<VAPM_APSSpeedCMD_kph>"
  outpmodule/453(VOUTP_ISAMalfuncDetDTC_raw32) -> bus_creator/453
  outpmodule/699(VOUTP_sigSetTempZon2StM_C) -> bus_creator/699
  bus_selector2/165 -> outpmodule/168(VAPM_PUIDLowPower_flg)  "<VAPM_PUIDLowPower_flg>"
  bus_selector2/163 -> outpmodule/166(VAPM_DKCPDkeyAreaRAPSSta_enum)  "<VAPM_DKCPDkeyAreaRAPSSta_enum>"
  bus_selector2/164 -> outpmodule/167(VAPM_DKCParkingModeCmd_enum)  "<VAPM_DKCParkingModeCmd_enum>"
  bus_selector2/160 -> outpmodule/163(VAPM_APSVRqEPASCtrl_flg)  "<VAPM_APSVRqEPASCtrl_flg>"
  bus_selector11/130 -> outpmodule/779(VTHC_FDCTHCCREVentZStaSet3_enum)  "<VTHC_FDCTHCCREVentZStaSet3_enum>"
  bus_selector11/47 -> outpmodule/696(VTHC_RecAutoFlg_flg)  "<VTHC_RecAutoFlg_flg>"
  bus_selector2/159 -> outpmodule/162(VAPM_APSAngleTarget_Deg)  "<VAPM_APSAngleTarget_Deg>"
  bus_selector2/155 -> outpmodule/158(VAPM_APSRQDisplay_enum)  "<VAPM_APSRQDisplay_enum>"
  bus_selector2/157 -> outpmodule/160(VAPM_APSHWVer_enum)  "<VAPM_APSHWVer_enum>"
  outpmodule/695(VOUTP_CCUSyncSts_flg) -> bus_creator/695
  bus_selector2/156 -> outpmodule/159(VAPM_APSSWVer_enum)  "<VAPM_APSSWVer_enum>"
  bus_selector3/36 -> outpmodule/214(VBCM_MirrorCtrl_enum)  "<VBCM_MirrorCtrl_enum>"
  outpmodule/297(VOUTP_SPTGENFun_flg) -> bus_creator/297
  bus_selector13/12 -> outpmodule/934(VTQD_RrRgnDecrSta_flg)  "<VTQD_RrRgnDecrSta_flg>"
  bus_selector2/153 -> outpmodule/156(VAPM_DriverSeatBeltCmdTimeOut_flg)  "<VAPM_DriverSeatBeltCmdTimeOut_flg>"
  outpmodule/531(VOUTP_KeyAreaPS_enum) -> bus_creator/531
  outpmodule/497(VOUTP_HVRlyOpFail_flg) -> bus_creator/497
  bus_selector12/48 -> outpmodule/873(VTPM_S3L_enum)  "<VTPM_S3L_enum>"
  bus_selector12/22 -> outpmodule/847(VTPM_TPMSCaliButtAllow_flg)  "<VTPM_TPMSCaliButtAllow_flg>"
  bus_selector2/154 -> outpmodule/157(VAPM_APSProgressPCT_pct)  "<VAPM_APSProgressPCT_pct>"
  bus_selector2/150 -> outpmodule/153(VAPM_TCSActive_flg)  "<VAPM_TCSActive_flg>"
  bus_selector10/41 -> outpmodule/647(VSYS_ModelYear_cnt)  "<VSYS_ModelYear_cnt>"
  bus_selector10/40 -> outpmodule/646(VSYS_DrivingMode_cnt)  "<VSYS_DrivingMode_cnt>"
  bus_selector2/75 -> outpmodule/78(VAPM_RRPulseCountVTimeOut_flg)  "<VAPM_RRPulseCountVTimeOut_flg>"
  bus_selector10/43 -> outpmodule/649(VSYS_Var5_cnt)  "<VSYS_Var5_cnt>"
  bus_selector11/123 -> outpmodule/772(VTHC_FDCTHCREVentZStaSet2_enum)  "<VTHC_FDCTHCREVentZStaSet2_enum>"
  outpmodule/267(VOUTP_AmbBrightSta_enum) -> bus_creator/267
  bus_selector3/119 -> outpmodule/297(VBCM_SPTGENFun_flg)  "<VBCM_SPTGENFun_flg>"
  bus_selector11/122 -> outpmodule/771(VTHC_FDCTHCREVentZStaSet1_enum)  "<VTHC_FDCTHCREVentZStaSet1_enum>"
  bus_selector11/121 -> outpmodule/770(VTHC_FDCTHCCLEVentZStaSet7_enum)  "<VTHC_FDCTHCCLEVentZStaSet7_enum>"
  bus_selector11/117 -> outpmodule/766(VTHC_FDCTHCCLEVentZStaSet2_enum)  "<VTHC_FDCTHCCLEVentZStaSet2_enum>"
  bus_selector9/30 -> outpmodule/588(VPMM_SilentChkAllowSleep_flg)  "<VPMM_SilentChkAllowSleep_flg>"
  bus_selector11/116 -> outpmodule/765(VTHC_FDCTHCCLEVentZStaSet1_enum)  "<VTHC_FDCTHCCLEVentZStaSet1_enum>"
  bus_selector11/16 -> outpmodule/665(VTHC_FDFrLeAPTCHeatPwrCmd_W)  "<VTHC_FDFrLeAPTCHeatPwrCmd_W>"
  bus_selector11/114 -> outpmodule/763(VTHC_FDCTHCLEVentZStaSet5_enum)  "<VTHC_FDCTHCLEVentZStaSet5_enum>"
  bus_selector11/111 -> outpmodule/760(VTHC_FDCTHCLEVentZStaSet2_enum)  "<VTHC_FDCTHCLEVentZStaSet2_enum>"
  bus_selector3/81 -> outpmodule/259(VBCM_APMDoorControlSta_flg)  "<VBCM_APMDoorControlSta_flg>"
  bus_selector11/110 -> outpmodule/759(VTHC_FDCTHCLEVentZStaSet1_enum)  "<VTHC_FDCTHCLEVentZStaSet1_enum>"
  outpmodule/603(VOUTP_PwrReq_OTA_enum) -> bus_creator/603
  bus_selector11/109 -> outpmodule/758(VTHC_REVentModeStaSet457_enum)  "<VTHC_REVentModeStaSet457_enum>"
  bus_selector4/78 -> outpmodule/435(VDDM_FCM2CSErrDTC_raw32)  "<VDDM_FCM2CSErrDTC_raw32>"
  bus_selector13/10 -> outpmodule/932(VTQD_RrActvDmpDisabReq_flg)  "<VTQD_RrActvDmpDisabReq_flg>"
  bus_selector2/52 -> outpmodule/55(VAPM_LFRawWhlSpeedV_flg)  "<VAPM_LFRawWhlSpeedV_flg>"
  outpmodule/480(VOUTP_LFSensorFailDTC_raw32) -> bus_creator/480
  bus_selector11/108 -> outpmodule/757(VTHC_REVentModeStaSet123_enum)  "<VTHC_REVentModeStaSet123_enum>"
  bus_selector9/22 -> outpmodule/580(VPMM_PwrDownReq_enum)  "<VPMM_PwrDownReq_enum>"
  bus_selector11/107 -> outpmodule/756(VTHC_LEVentModeStaSet457_enum)  "<VTHC_LEVentModeStaSet457_enum>"
  bus_selector11/105 -> outpmodule/754(VTHC_CRVentENSet_enum)  "<VTHC_CRVentENSet_enum>"
  bus_selector2/32 -> outpmodule/35(VAPM_USSStaFMR_flg)  "<VAPM_USSStaFMR_flg>"
  outpmodule/601(VOUTP_PwrStaTOSta_enum) -> bus_creator/601
  outpmodule/970(VOUTP_SetSpd_kph) -> bus_creator/970
  bus_selector11/104 -> outpmodule/753(VTHC_RVentENSet_enum)  "<VTHC_RVentENSet_enum>"
  bus_selector11/103 -> outpmodule/752(VTHC_CLVentENSet_enum)  "<VTHC_CLVentENSet_enum>"
  outpmodule/866(VOUTP_RRSensorMode_flg) -> bus_creator/866
  outpmodule/753(VOUTP_RVentENSet_enum) -> bus_creator/753
  bus_selector11/102 -> outpmodule/751(VTHC_LVentENSet_enum)  "<VTHC_LVentENSet_enum>"
  bus_selector11/101 -> outpmodule/750(VTHC_FDCFGSAirIntStaSet457_enum)  "<VTHC_FDCFGSAirIntStaSet457_enum>"
  bus_selector11/21 -> outpmodule/670(VTHC_EDriveMode_enum)  "<VTHC_EDriveMode_enum>"
  bus_selector11/100 -> outpmodule/749(VTHC_FDCFGSAirIntStaSet123_enum)  "<VTHC_FDCFGSAirIntStaSet123_enum>"
  bus_selector2/122 -> outpmodule/125(VAPM_ESCStandstill_flg)  "<VAPM_ESCStandstill_flg>"
  BSYS_outputs/1 -> bus_selector10/1
  bus_selector4/2 -> outpmodule/359(VDDM_C3BMS6CSDTC_raw32)  "<VDDM_C3BMS6CSDTC_raw32>"
  bus_selector4/161 -> outpmodule/518(VDDM_CAN6BusOffDTC_raw32)  "<VDDM_CAN6BusOffDTC_raw32>"
  bus_selector4/160 -> outpmodule/517(VDDM_CAN5BusOffDTC_raw32)  "<VDDM_CAN5BusOffDTC_raw32>"
  bus_selector4/158 -> outpmodule/515(VDDM_CAN3BusOffDTC_raw32)  "<VDDM_CAN3BusOffDTC_raw32>"
  bus_selector4/159 -> outpmodule/516(VDDM_CAN4BusOffDTC_raw32)  "<VDDM_CAN4BusOffDTC_raw32>"
  outpmodule/265(VOUTP_AmbODAEN_flg) -> bus_creator/265
  bus_selector4/157 -> outpmodule/514(VDDM_CAN2BusOffDTC_raw32)  "<VDDM_CAN2BusOffDTC_raw32>"
  bus_selector4/154 -> outpmodule/511(VDDM_CAN5BusErrorDTC_raw32)  "<VDDM_CAN5BusErrorDTC_raw32>"
  bus_selector2/170 -> outpmodule/173(VAPM_RAPSBCMLamp_enum)  "<VAPM_RAPSBCMLamp_enum>"
  bus_selector2/33 -> outpmodule/36(VAPM_USSStaFML_flg)  "<VAPM_USSStaFML_flg>"
  bus_selector4/151 -> outpmodule/508(VDDM_CAN2BusErrorDTC_raw32)  "<VDDM_CAN2BusErrorDTC_raw32>"
  bus_selector4/149 -> outpmodule/506(VDDM_VCUTailgateSWSta_flg)  "<VDDM_VCUTailgateSWSta_flg>"
  outpmodule/470(VOUTP_LRBatwarnDTC_raw32) -> bus_creator/470
  bus_selector4/148 -> outpmodule/505(VDDM_VCUHoodSWSta_flg)  "<VDDM_VCUHoodSWSta_flg>"
  bus_selector4/147 -> outpmodule/504(VDDM_SysAllowReadySta_flg)  "<VDDM_SysAllowReadySta_flg>"
  bus_selector4/142 -> outpmodule/499(VDDM_VCUBrkSWSta_enum)  "<VDDM_VCUBrkSWSta_enum>"
  bus_selector2/70 -> outpmodule/73(VAPM_RFPulseCountV_flg)  "<VAPM_RFPulseCountV_flg>"
  bus_selector4/139 -> outpmodule/496(VDDM_LVSysErrPwrOutErr_flg)  "<VDDM_LVSysErrPwrOutErr_flg>"
  bus_selector4/136 -> outpmodule/493(VDDM_VCURAPSErrLv2_flg)  "<VDDM_VCURAPSErrLv2_flg>"
  bus_selector4/135 -> outpmodule/492(VDDM_DisengagePFail_flg)  "<VDDM_DisengagePFail_flg>"
  bus_selector2/152 -> outpmodule/155(VAPM_DriverSeatBeltCmd_flg)  "<VAPM_DriverSeatBeltCmd_flg>"
  bus_selector4/137 -> outpmodule/494(VDDM_VCURAPSErrLv3_flg)  "<VDDM_VCURAPSErrLv3_flg>"
  outpmodule/876(VOUTP_LFP20_raw8) -> bus_creator/876
  outpmodule/723(VOUTP_FDCFGSIONCmd_flg) -> bus_creator/723
  bus_selector8/10 -> outpmodule/556(VNMM_ActiveWU_flg)  "<VNMM_ActiveWU_flg>"
  outpmodule/506(VOUTP_VCUTailgateSWSta_flg) -> bus_creator/506
  bus_selector6/1 -> outpmodule/525(VDKC_DKCTimeSN_cnt)  "<VDKC_DKCTimeSN_cnt>"
  bus_selector8/9 -> outpmodule/555(VNMM_WakeUp_enum)  "<VNMM_WakeUp_enum>"
  bus_selector9/12 -> outpmodule/570(VPMM_HVPwrSta_flg)  "<VPMM_HVPwrSta_flg>"
  bus_selector5/1 -> outpmodule/519(VDHP_ActAPSPosn_pct)  "<VDHP_ActAPSPosn_pct>"
  bus_selector9/21 -> outpmodule/579(VPMM_PwrUpReq_enum)  "<VPMM_PwrUpReq_enum>"
  bus_selector5/3 -> outpmodule/521(VDHP_EAPS2MIN_pct)  "<VDHP_EAPS2MIN_pct>"
  bus_selector13/41 -> outpmodule/963(VTQD_ActParkRequest_flg)  "<VTQD_ActParkRequest_flg>"
  outpmodule/698(VOUTP_fdefog_flg) -> bus_creator/698
  bus_selector5/2 -> outpmodule/520(VDHP_EAPS1MIN_pct)  "<VDHP_EAPS1MIN_pct>"
  bus_selector5/4 -> outpmodule/522(VDHP_ResetPedalZeroPosStart_flg)  "<VDHP_ResetPedalZeroPosStart_flg>"
  BNMM_outputs/1 -> bus_selector8/1
  bus_selector6/8 -> outpmodule/532(VDKC_KeyAreaLockUnlock_enum)  "<VDKC_KeyAreaLockUnlock_enum>"
  bus_selector3/57 -> outpmodule/235(VBCM_AmbLightBrightness4_enum)  "<VBCM_AmbLightBrightness4_enum>"
  outpmodule/390(VOUTP_DCDCDisDTC_raw32) -> bus_creator/390
  bus_selector6/6 -> outpmodule/530(VDKC_DkeyShowIVISta_enum)  "<VDKC_DkeyShowIVISta_enum>"
  outpmodule/978(VOUTP_ReqV2LIVIDisChrg_enum) -> bus_creator/978
  bus_selector8/11 -> outpmodule/557(VNMM_SysNMmSta_enum)  "<VNMM_SysNMmSta_enum>"
  outpmodule/925(VOUTP_TqSourceRr_enum) -> bus_creator/925
  bus_selector10/38 -> outpmodule/644(VSYS_ECUGen2_cnt)  "<VSYS_ECUGen2_cnt>"
  bus_selector3/54 -> outpmodule/232(VBCM_AmbLightBrightness1_enum)  "<VBCM_AmbLightBrightness1_enum>"
  outpmodule/259(VOUTP_APMDoorControlSta_flg) -> bus_creator/259
  outpmodule/924(VOUTP_TqSourceFr_enum) -> bus_creator/924
  outpmodule/264(VOUTP_AmbPwrWarnEN_flg) -> bus_creator/264
  outpmodule/923(VOUTP_ParkRequest_flg) -> bus_creator/923
  bus_selector12/60 -> outpmodule/885(VTPM_S4WheelDebugALTU_pct)  "<VTPM_S4WheelDebugALTU_pct>"
  outpmodule/918(VOUTP_TPMSTLCmd_flg) -> bus_creator/918
  bus_selector12/15 -> outpmodule/840(VTPM_LRSensorFail_flg)  "<VTPM_LRSensorFail_flg>"
  outpmodule/920(VOUTP_TPMSSensorIDRegStart_flg) -> bus_creator/920
  outpmodule/1037(VOUTP_ACCObjDstLvl_enum) -> bus_creator/1037
  outpmodule/919(VOUTP_LProgress_enum) -> bus_creator/919
  outpmodule/916(VOUTP_FlashIDvalid_enum) -> bus_creator/916
  outpmodule/525(VOUTP_DKCTimeSN_cnt) -> bus_creator/525
  bus_selector12/53 -> outpmodule/878(VTPM_LRP20_raw8)  "<VTPM_LRP20_raw8>"
  outpmodule/947(VOUTP_RgnAbnorSta_flg) -> bus_creator/947
  outpmodule/941(VOUTP_FrEDUSpd_rpm) -> bus_creator/941
  outpmodule/943(VOUTP_FrEDUSpdValid_flg) -> bus_creator/943
  bus_selector4/132 -> outpmodule/489(VDDM_LimpHomeActTmp_flg)  "<VDDM_LimpHomeActTmp_flg>"
  outpmodule/942(VOUTP_RrEDUSpd_rpm) -> bus_creator/942
  bus_selector13/48 -> outpmodule/970(VTQD_SetSpd_kph)  "<VTQD_SetSpd_kph>"
  outpmodule/939(VOUTP_FrEDURolRgnTq_Nm) -> bus_creator/939
  bus_selector1/1 -> outpmodule/1(VACC_HVTHCMSysAvail_enum)  "<VACC_HVTHCMSysAvail_enum>"
  outpmodule/940(VOUTP_RrEDURolRgnTq_Nm) -> bus_creator/940
  outpmodule/938(VOUTP_RrEDUActTq_Nm) -> bus_creator/938
  outpmodule/935(VOUTP_DriverWhlTqDemFr_Nm) -> bus_creator/935
  outpmodule/1042(VOUTP_TargetType_enum) -> bus_creator/1042
  outpmodule/934(VOUTP_RrRgnDecrSta_flg) -> bus_creator/934
  outpmodule/1050(VOUTP_ADASISASta_enum) -> bus_creator/1050
  bus_selector12/69 -> outpmodule/894(VTPM_TPMSResButt_flg)  "<VTPM_TPMSResButt_flg>"
  outpmodule/933(VOUTP_FrRgnDecrSta_flg) -> bus_creator/933
  bus_selector11/8 -> outpmodule/657(VTHC_FDFWVCmd_flg)  "<VTHC_FDFWVCmd_flg>"
  outpmodule/299(VOUTP_OutMode_enum) -> bus_creator/299
  outpmodule/931(VOUTP_FrActvDmpDisabReq_flg) -> bus_creator/931
  outpmodule/928(VOUTP_EVDriveMode_enum) -> bus_creator/928
  bus_selector10/10 -> outpmodule/616(VSYS_Major2_cnt)  "<VSYS_Major2_cnt>"
  outpmodule/261(VOUTP_AmbWelEN_flg) -> bus_creator/261
  bus_selector10/6 -> outpmodule/612(VSYS_CarModel3_cnt)  "<VSYS_CarModel3_cnt>"
  outpmodule/543(VOUTP_DISCTurn_flg) -> bus_creator/543
  bus_selector4/156 -> outpmodule/513(VDDM_CAN1BusOffDTC_raw32)  "<VDDM_CAN1BusOffDTC_raw32>"
  bus_selector10/4 -> outpmodule/610(VSYS_CarModel1_cnt)  "<VSYS_CarModel1_cnt>"
  outpmodule/301(VOUTP_TurnSwTimeSetSta457_enum) -> bus_creator/301
  bus_selector10/2 -> outpmodule/608(VSYS_HWVer2_cnt)  "<VSYS_HWVer2_cnt>"
  bus_selector9/48 -> outpmodule/606(VPMM_PwrReqRAPSAvail_flg)  "<VPMM_PwrReqRAPSAvail_flg>"
  outpmodule/581(VOUTP_LowSOCWarn_enum) -> bus_creator/581
  bus_selector9/45 -> outpmodule/603(VPMM_PwrReq_OTA_enum)  "<VPMM_PwrReq_OTA_enum>"
  bus_selector9/44 -> outpmodule/602(VPMM_Sched_ChgTOSta_enum)  "<VPMM_Sched_ChgTOSta_enum>"
  outpmodule/389(VOUTP_MCUDisDTC_raw32) -> bus_creator/389
  outpmodule/839(VOUTP_RFSensorFail_flg) -> bus_creator/839
  outpmodule/305(VOUTP_HBeamADB_flg) -> bus_creator/305
  bus_selector2/31 -> outpmodule/34(VAPM_USSStaRCL_flg)  "<VAPM_USSStaRCL_flg>"
  outpmodule/1016(VOUTP_AEBVehHoldReq_flg) -> bus_creator/1016
  bus_selector9/42 -> outpmodule/600(VPMM_CtrlDrPwrStbA2_flg)  "<VPMM_CtrlDrPwrStbA2_flg>"
  bus_selector9/38 -> outpmodule/596(VPMM_CtrlFrRC1_flg)  "<VPMM_CtrlFrRC1_flg>"
  outpmodule/503(VOUTP_VCURRDoorSta_flg) -> bus_creator/503
  outpmodule/1045(VOUTP_LKAHODSoundWarning_flg) -> bus_creator/1045
  bus_selector9/36 -> outpmodule/594(VPMM_LVSilentChrgLv_enum)  "<VPMM_LVSilentChrgLv_enum>"
  bus_selector13/16 -> outpmodule/938(VTQD_RrEDUActTq_Nm)  "<VTQD_RrEDUActTq_Nm>"
  bus_selector9/32 -> outpmodule/590(VPMM_FDADC12VDetAvg_mV)  "<VPMM_FDADC12VDetAvg_mV>"
  bus_selector4/124 -> outpmodule/481(VDDM_RFSensorFailDTC_raw32)  "<VDDM_RFSensorFailDTC_raw32>"
  bus_selector3/46 -> outpmodule/224(VBCM_WasherCtrl_enum)  "<VBCM_WasherCtrl_enum>"
  outpmodule/520(VOUTP_EAPS1MIN_pct) -> bus_creator/520
  bus_selector12/85 -> outpmodule/910(VTPM_unlearnSfailvalid_enum)  "<VTPM_unlearnSfailvalid_enum>"
  bus_selector9/33 -> outpmodule/591(VPMM_PMMAllowECUSleep_flg)  "<VPMM_PMMAllowECUSleep_flg>"
  bus_selector10/37 -> outpmodule/643(VSYS_ECUGen1_cnt)  "<VSYS_ECUGen1_cnt>"
  bus_selector2/25 -> outpmodule/28(VAPM_PASAFCR_enum)  "<VAPM_PASAFCR_enum>"
  outpmodule/805(VOUTP_FDCTHCCREVentYStaSet5_enum) -> bus_creator/805
  bus_selector10/34 -> outpmodule/640(VSYS_WisrBootReason_raw32)  "<VSYS_WisrBootReason_raw32>"
  bus_selector10/1 -> outpmodule/607(VSYS_HWVer1_cnt)  "<VSYS_HWVer1_cnt>"
  bus_selector10/29 -> outpmodule/635(VSYS_SHA8_cnt)  "<VSYS_SHA8_cnt>"
  outpmodule/810(VOUTP_SettempZon1Set4_enum) -> bus_creator/810
  BDHP_outputs/1 -> bus_selector5/1
  outpmodule/551(VOUTP_ErrorState_enum) -> bus_creator/551
  bus_selector10/32 -> outpmodule/638(VSYS_FdcSlpTime_sec)  "<VSYS_FdcSlpTime_sec>"
  bus_selector6/5 -> outpmodule/529(VDKC_KeyModeSta_enum)  "<VDKC_KeyModeSta_enum>"
  bus_selector10/26 -> outpmodule/632(VSYS_SHA5_cnt)  "<VSYS_SHA5_cnt>"
  bus_selector4/155 -> outpmodule/512(VDDM_CAN6BusErrorDTC_raw32)  "<VDDM_CAN6BusErrorDTC_raw32>"
  bus_selector10/27 -> outpmodule/633(VSYS_SHA6_cnt)  "<VSYS_SHA6_cnt>"
  bus_selector11/154 -> outpmodule/803(VTHC_FDCTHCCREVentYStaSet3_enum)  "<VTHC_FDCTHCCREVentYStaSet3_enum>"
  bus_selector10/28 -> outpmodule/634(VSYS_SHA7_cnt)  "<VSYS_SHA7_cnt>"
  bus_selector10/25 -> outpmodule/631(VSYS_SHA4_cnt)  "<VSYS_SHA4_cnt>"
  outpmodule/913(VOUTP_FlashS2ID_raw) -> bus_creator/913
  bus_selector10/20 -> outpmodule/626(VSYS_Change2_cnt)  "<VSYS_Change2_cnt>"
  bus_selector10/19 -> outpmodule/625(VSYS_Change1_cnt)  "<VSYS_Change1_cnt>"
  bus_selector3/30 -> outpmodule/208(VBCM_LBSD_flg)  "<VBCM_LBSD_flg>"
  bus_selector10/21 -> outpmodule/627(VSYS_Dash2_cnt)  "<VSYS_Dash2_cnt>"
  outpmodule/555(VOUTP_WakeUp_enum) -> bus_creator/555
  bus_selector10/17 -> outpmodule/623(VSYS_Variation_cnt)  "<VSYS_Variation_cnt>"
  bus_selector4/141 -> outpmodule/498(VDDM_MCUActDisFail_flg)  "<VDDM_MCUActDisFail_flg>"
  outpmodule/945(VOUTP_RrEDUSpdValid_flg) -> bus_creator/945
  bus_selector10/18 -> outpmodule/624(VSYS_Dash1_cnt)  "<VSYS_Dash1_cnt>"
  bus_selector10/15 -> outpmodule/621(VSYS_Country1_cnt)  "<VSYS_Country1_cnt>"
  bus_selector4/113 -> outpmodule/470(VDDM_LRBatwarnDTC_raw32)  "<VDDM_LRBatwarnDTC_raw32>"
  bus_selector3/49 -> outpmodule/227(VBCM_AmbLightBreath2_enum)  "<VBCM_AmbLightBreath2_enum>"
  bus_selector4/35 -> outpmodule/392(VDDM_MCUActDTC_raw32)  "<VDDM_MCUActDTC_raw32>"
  outpmodule/821(VOUTP_CRVentEN_flg) -> bus_creator/821
  bus_selector4/33 -> outpmodule/390(VDDM_DCDCDisDTC_raw32)  "<VDDM_DCDCDisDTC_raw32>"
  bus_selector4/30 -> outpmodule/387(VDDM_HiLvSaChkDTC_raw32)  "<VDDM_HiLvSaChkDTC_raw32>"
  outpmodule/694(VOUTP_FootM_flg) -> bus_creator/694
  outpmodule/952(VOUTP_FrIdcMax_A) -> bus_creator/952
  bus_selector4/29 -> outpmodule/386(VDDM_DCDCEnaDTC_raw32)  "<VDDM_DCDCEnaDTC_raw32>"
  bus_selector4/112 -> outpmodule/469(VDDM_RFBatwarnDTC_raw32)  "<VDDM_RFBatwarnDTC_raw32>"
  bus_selector4/25 -> outpmodule/382(VDDM_MCU4PreDTC_raw32)  "<VDDM_MCU4PreDTC_raw32>"
  outpmodule/434(VOUTP_FCM2RCErrDTC_raw32) -> bus_creator/434
  outpmodule/836(VOUTP_LRWheelTemp_C) -> bus_creator/836
  bus_selector11/115 -> outpmodule/764(VTHC_FDCTHCLEVentZStaSet7_enum)  "<VTHC_FDCTHCLEVentZStaSet7_enum>"
  bus_selector3/86 -> outpmodule/264(VBCM_AmbPwrWarnEN_flg)  "<VBCM_AmbPwrWarnEN_flg>"
  bus_selector4/26 -> outpmodule/383(VDDM_DCDC4PreDTC_raw32)  "<VDDM_DCDC4PreDTC_raw32>"
  bus_selector2/63 -> outpmodule/66(VAPM_RFWhlRotDirTimeOut_flg)  "<VAPM_RFWhlRotDirTimeOut_flg>"
  bus_selector2/138 -> outpmodule/141(VAPM_AVMParkingmode_enum)  "<VAPM_AVMParkingmode_enum>"
  outpmodule/281(VOUTP_AmbColorSta4_enum) -> bus_creator/281
  bus_selector4/27 -> outpmodule/384(VDDM_HVRlyCloDTC_raw32)  "<VDDM_HVRlyCloDTC_raw32>"
  bus_selector4/117 -> outpmodule/474(VDDM_LRPressIndiDTC_raw32)  "<VDDM_LRPressIndiDTC_raw32>"
  bus_selector10/13 -> outpmodule/619(VSYS_Patch1_cnt)  "<VSYS_Patch1_cnt>"
  bus_selector4/23 -> outpmodule/380(VDDM_ONtoRdyDTC_raw32)  "<VDDM_ONtoRdyDTC_raw32>"
  bus_selector10/36 -> outpmodule/642(VSYS_CurrentNmState_enum)  "<VSYS_CurrentNmState_enum>"
  bus_selector4/24 -> outpmodule/381(VDDM_HVB4PreDTC_raw32)  "<VDDM_HVB4PreDTC_raw32>"
  bus_selector2/140 -> outpmodule/143(VAPM_AVMErrSTA_flg)  "<VAPM_AVMErrSTA_flg>"
  bus_selector4/20 -> outpmodule/377(VDDM_BrkSWErrDTC_raw32)  "<VDDM_BrkSWErrDTC_raw32>"
  outpmodule/1081(VOUTP_IMUEnaCmd_flg) -> bus_creator/1081
  bus_selector4/19 -> outpmodule/376(VDDM_Lv4ErrDTC_raw32)  "<VDDM_Lv4ErrDTC_raw32>"
  bus_selector4/16 -> outpmodule/373(VDDM_Lv1ErrDTC_raw32)  "<VDDM_Lv1ErrDTC_raw32>"
  outpmodule/313(VOUTP_RmLpModeENFunSta_flg) -> bus_creator/313
  bus_selector12/10 -> outpmodule/835(VTPM_RFWheelTemp_C)  "<VTPM_RFWheelTemp_C>"
  bus_selector4/17 -> outpmodule/374(VDDM_Lv2ErrDTC_raw32)  "<VDDM_Lv2ErrDTC_raw32>"
  bus_selector4/12 -> outpmodule/369(VDDM_C3CCU2LCDTC_raw32)  "<VDDM_C3CCU2LCDTC_raw32>"
  bus_selector4/13 -> outpmodule/370(VDDM_C1ABM1RCDTC_raw32)  "<VDDM_C1ABM1RCDTC_raw32>"
  bus_selector3/125 -> outpmodule/303(VBCM_FDRHandleLampCmd_flg)  "<VBCM_FDRHandleLampCmd_flg>"
  bus_selector4/32 -> outpmodule/389(VDDM_MCUDisDTC_raw32)  "<VDDM_MCUDisDTC_raw32>"
  bus_selector2/37 -> outpmodule/40(VAPM_USSStaFCL_flg)  "<VAPM_USSStaFCL_flg>"
  outpmodule/1058(VOUTP_LVDAACCStatusInformation_flg) -> bus_creator/1058
  bus_selector12/34 -> outpmodule/859(VTPM_RFWheelPSW_raw8)  "<VTPM_RFWheelPSW_raw8>"
  bus_selector4/58 -> outpmodule/415(VDDM_EnterNewOperCyc_flg)  "<VDDM_EnterNewOperCyc_flg>"
  bus_creator/1 -> BOUTP_outputs/1
  bus_selector4/57 -> outpmodule/414(VDDM_ESC5NoComDTC_raw32)  "<VDDM_ESC5NoComDTC_raw32>"
  outpmodule/974(VOUTP_FrTMTqReq_Nm) -> bus_creator/974
  bus_selector4/53 -> outpmodule/410(VDDM_MCUR1NoComDTC_raw32)  "<VDDM_MCUR1NoComDTC_raw32>"
  bus_selector4/54 -> outpmodule/411(VDDM_Shifter1NoComDTC_raw32)  "<VDDM_Shifter1NoComDTC_raw32>"
  bus_selector10/14 -> outpmodule/620(VSYS_Patch2_cnt)  "<VSYS_Patch2_cnt>"
  bus_selector4/50 -> outpmodule/407(VDDM_APS2SigOoRDTC_raw32)  "<VDDM_APS2SigOoRDTC_raw32>"
  bus_selector4/51 -> outpmodule/408(VDDM_APSCorrErrDTC_raw32)  "<VDDM_APSCorrErrDTC_raw32>"
  bus_selector4/49 -> outpmodule/406(VDDM_APS1SigOoRDTC_raw32)  "<VDDM_APS1SigOoRDTC_raw32>"
  bus_selector2/101 -> outpmodule/104(VAPM_GRADETimeOut_flg)  "<VAPM_GRADETimeOut_flg>"
  bus_selector2/169 -> outpmodule/172(VAPM_APSVMCReqA_flg)  "<VAPM_APSVMCReqA_flg>"
  bus_selector4/48 -> outpmodule/405(VDDM_VehMalfunLevel_enum)  "<VDDM_VehMalfunLevel_enum>"
  bus_selector13/33 -> outpmodule/955(VTQD_RrIdcMin_A)  "<VTQD_RrIdcMin_A>"
  bus_selector4/45 -> outpmodule/402(VDDM_HoodSWDTC_raw32)  "<VDDM_HoodSWDTC_raw32>"
  bus_selector4/39 -> outpmodule/396(VDDM_LVSupHiDTC_raw32)  "<VDDM_LVSupHiDTC_raw32>"
  bus_selector4/36 -> outpmodule/393(VDDM_OBC4PreDTC_raw32)  "<VDDM_OBC4PreDTC_raw32>"
  outpmodule/969(VOUTP_SpdCtrlSta_flg) -> bus_creator/969
  bus_selector4/152 -> outpmodule/509(VDDM_CAN3BusErrorDTC_raw32)  "<VDDM_CAN3BusErrorDTC_raw32>"
  outpmodule/246(VOUTP_APSOpenPTG_flg) -> bus_creator/246
  bus_selector11/176 -> outpmodule/825(VTHC_sigCbnPTCPwrAct_W)  "<VTHC_sigCbnPTCPwrAct_W>"
  bus_selector1/2 -> outpmodule/2(VACC_LVBattVoltSta_enum)  "<VACC_LVBattVoltSta_enum>"
  outpmodule/830(VOUTP_LFWheelPress_raw8) -> bus_creator/830
  outpmodule/244(VOUTP_LampPwr_flg) -> bus_creator/244
  bus_selector6/7 -> outpmodule/531(VDKC_KeyAreaPS_enum)  "<VDKC_KeyAreaPS_enum>"
  outpmodule/243(VOUTP_AmbLightColor6_enum) -> bus_creator/243
  bus_selector11/29 -> outpmodule/678(VTHC_sigRecircSt_flg)  "<VTHC_sigRecircSt_flg>"
  outpmodule/242(VOUTP_AmbLightColor5_enum) -> bus_creator/242
  bus_selector13/6 -> outpmodule/928(VTQD_EVDriveMode_enum)  "<VTQD_EVDriveMode_enum>"
  bus_selector3/68 -> outpmodule/246(VBCM_APSOpenPTG_flg)  "<VBCM_APSOpenPTG_flg>"
  bus_selector9/2 -> outpmodule/560(VPMM_PowerDownState_enum)  "<VPMM_PowerDownState_enum>"
  bus_selector2/26 -> outpmodule/29(VAPM_USSStaRMR_flg)  "<VAPM_USSStaRMR_flg>"
  outpmodule/433(VOUTP_FCM2NoComDTC_raw32) -> bus_creator/433
  outpmodule/239(VOUTP_AmbLightColor2_enum) -> bus_creator/239
  bus_selector4/134 -> outpmodule/491(VDDM_EngagePFail_flg)  "<VDDM_EngagePFail_flg>"
  outpmodule/235(VOUTP_AmbLightBrightness4_enum) -> bus_creator/235
  outpmodule/793(VOUTP_FDCTHCCLEVentYStaSet5_enum) -> bus_creator/793
  bus_selector2/141 -> outpmodule/144(VAPM_AVMErrSTATimeOut_flg)  "<VAPM_AVMErrSTATimeOut_flg>"
  outpmodule/1022(VOUTP_TimeGapLevel_enum) -> bus_creator/1022
  bus_selector4/47 -> outpmodule/404(VDDM_EDriveSysErrVCUErr_flg)  "<VDDM_EDriveSysErrVCUErr_flg>"
  outpmodule/342(VOUTP_HMIKey4FuncSta_enum) -> bus_creator/342
  outpmodule/234(VOUTP_AmbLightBrightness3_enum) -> bus_creator/234
  outpmodule/227(VOUTP_AmbLightBreath2_enum) -> bus_creator/227
  bus_selector2/23 -> outpmodule/26(VAPM_PASAFMR_enum)  "<VAPM_PASAFMR_enum>"
  outpmodule/666(VOUTP_FDFrRiAPTCHeatPwrCmd_W) -> bus_creator/666
  outpmodule/229(VOUTP_AmbLightBreath4_enum) -> bus_creator/229
  bus_selector9/16 -> outpmodule/574(VPMM_DrivetrainSelect_enum)  "<VPMM_DrivetrainSelect_enum>"
  outpmodule/223(VOUTP_RrWiper_flg) -> bus_creator/223
  outpmodule/220(VOUTP_TailgateHDSW_flg) -> bus_creator/220
  outpmodule/221(VOUTP_FrWiperL_flg) -> bus_creator/221
  outpmodule/215(VOUTP_MirrorDefog_flg) -> bus_creator/215
  outpmodule/687(VOUTP_ACSubMode_enum) -> bus_creator/687
  outpmodule/214(VOUTP_MirrorCtrl_enum) -> bus_creator/214
  outpmodule/213(VOUTP_BCMBuzzerReq_flg) -> bus_creator/213
  bus_selector3/51 -> outpmodule/229(VBCM_AmbLightBreath4_enum)  "<VBCM_AmbLightBreath4_enum>"
  bus_selector3/47 -> outpmodule/225(VBCM_WiperFixMode_flg)  "<VBCM_WiperFixMode_flg>"
  bus_selector11/90 -> outpmodule/739(VTHC_AirIntenZone1MSet7_enum)  "<VTHC_AirIntenZone1MSet7_enum>"
  outpmodule/209(VOUTP_RBSD_flg) -> bus_creator/209
  bus_selector11/43 -> outpmodule/692(VTHC_Frost_flg)  "<VTHC_Frost_flg>"
  outpmodule/208(VOUTP_LBSD_flg) -> bus_creator/208
  outpmodule/204(VOUTP_BrakeLamp_flg) -> bus_creator/204
  outpmodule/201(VOUTP_LBeam_flg) -> bus_creator/201
  bus_selector9/46 -> outpmodule/604(VPMM_OTAPwrReqOFFChkSta_enum)  "<VPMM_OTAPwrReqOFFChkSta_enum>"
  outpmodule/199(VOUTP_DimmerEN_flg) -> bus_creator/199
  outpmodule/930(VOUTP_PButtonSta_enum) -> bus_creator/930
  outpmodule/200(VOUTP_PosLamp_flg) -> bus_creator/200
  bus_selector4/111 -> outpmodule/468(VDDM_LFBatwarnDTC_raw32)  "<VDDM_LFBatwarnDTC_raw32>"
  bus_selector3/37 -> outpmodule/215(VBCM_MirrorDefog_flg)  "<VBCM_MirrorDefog_flg>"
  bus_selector9/47 -> outpmodule/605(VPMM_OTAPwrReqStdChkSta_enum)  "<VPMM_OTAPwrReqStdChkSta_enum>"
  outpmodule/197(VOUTP_CTDLockSW_flg) -> bus_creator/197
  bus_selector3/41 -> outpmodule/219(VBCM_TrunkRel_flg)  "<VBCM_TrunkRel_flg>"
  outpmodule/198(VOUTP_Dimmer_pct) -> bus_creator/198
  bus_selector4/1 -> outpmodule/358(VDDM_C3BMS6RCDTC_raw32)  "<VDDM_C3BMS6RCDTC_raw32>"
  outpmodule/194(VOUTP_CrashDetd_flg) -> bus_creator/194
  outpmodule/1094(VOUTP_FDCVMCAngCtrlTqWtGn_pct) -> bus_creator/1094
  bus_selector2/161 -> outpmodule/164(VAPM_APSRqEPASCtrl_flg)  "<VAPM_APSRqEPASCtrl_flg>"
  outpmodule/192(VOUTP_FrChargingDoorCtrl_enum) -> bus_creator/192
  outpmodule/186(VOUTP_TailgateSW_flg) -> bus_creator/186
  bus_selector11/171 -> outpmodule/820(VTHC_RVentEN_flg)  "<VTHC_RVentEN_flg>"
  outpmodule/1051(VOUTP_ADASLDWMute_flg) -> bus_creator/1051
  outpmodule/958(VOUTP_RrUdcMax_V) -> bus_creator/958
  outpmodule/182(VOUTP_AllDoorSW_flg) -> bus_creator/182
  bus_selector13/43 -> outpmodule/965(VTQD_OPDHoldLamp_flg)  "<VTQD_OPDHoldLamp_flg>"
  outpmodule/179(VOUTP_AntitheftSta_enum) -> bus_creator/179
  outpmodule/766(VOUTP_FDCTHCCLEVentZStaSet2_enum) -> bus_creator/766
  bus_selector3/59 -> outpmodule/237(VBCM_AmbLightBrightness6_enum)  "<VBCM_AmbLightBrightness6_enum>"
  outpmodule/176(VOUTP_RAPSErrWarnSta_enum) -> bus_creator/176
  BDDM_outputs/1 -> bus_selector4/1
  outpmodule/802(VOUTP_FDCTHCCREVentYStaSet2_enum) -> bus_creator/802
  bus_selector3/75 -> outpmodule/253(VBCM_MFRDNBrightReq_pct)  "<VBCM_MFRDNBrightReq_pct>"
  outpmodule/1052(VOUTP_ADASFCWMute_flg) -> bus_creator/1052
  outpmodule/175(VOUTP_APSPwrReq_enum) -> bus_creator/175
  bus_selector12/3 -> outpmodule/828(VTPM_LRBatWarn_flg)  "<VTPM_LRBatWarn_flg>"
  bus_selector3/74 -> outpmodule/252(VBCM_FuelDoorPos_flg)  "<VBCM_FuelDoorPos_flg>"
  outpmodule/173(VOUTP_RAPSBCMLamp_enum) -> bus_creator/173
  outpmodule/251(VOUTP_MirrorFlodPos_flg) -> bus_creator/251
  outpmodule/177(VOUTP_RAPSErrLv1_flg) -> bus_creator/177
  outpmodule/250(VOUTP_MFSWTri_flg) -> bus_creator/250
  outpmodule/247(VOUTP_FollowMe_flg) -> bus_creator/247
  outpmodule/523(VOUTP_EAPS1NRM_pct) -> bus_creator/523
  outpmodule/948(VOUTP_PTCSPermSta_flg) -> bus_creator/948
  bus_selector3/26 -> outpmodule/204(VBCM_BrakeLamp_flg)  "<VBCM_BrakeLamp_flg>"
  outpmodule/1097(VOUTP_FDCVMCDrInpTqBstGn_pct) -> bus_creator/1097
  bus_selector3/25 -> outpmodule/203(VBCM_RrFogLamp_flg)  "<VBCM_RrFogLamp_flg>"
  outpmodule/509(VOUTP_CAN3BusErrorDTC_raw32) -> bus_creator/509
  outpmodule/1006(VOUTP_DISCReqAcc_mps2) -> bus_creator/1006
  outpmodule/764(VOUTP_FDCTHCLEVentZStaSet7_enum) -> bus_creator/764
  bus_selector3/19 -> outpmodule/197(VBCM_CTDLockSW_flg)  "<VBCM_CTDLockSW_flg>"
  bus_selector3/18 -> outpmodule/196(VBCM_DoorLockIND_flg)  "<VBCM_DoorLockIND_flg>"
  outpmodule/863(VOUTP_LFSensorMode_flg) -> bus_creator/863
  bus_selector3/17 -> outpmodule/195(VBCM_CTDCtrl_enum)  "<VBCM_CTDCtrl_enum>"
  outpmodule/861(VOUTP_CWheelTips_enum) -> bus_creator/861
  outpmodule/147(VOUTP_CAASSw_enum) -> bus_creator/147
  outpmodule/149(VOUTP_IVIScreen_enum) -> bus_creator/149
  bus_selector3/77 -> outpmodule/255(VBCM_DrvWdwCtrlCmd_pct)  "<VBCM_DrvWdwCtrlCmd_pct>"
  bus_selector11/112 -> outpmodule/761(VTHC_FDCTHCLEVentZStaSet3_enum)  "<VTHC_FDCTHCLEVentZStaSet3_enum>"
  outpmodule/146(VOUTP_IVIStatusTimeOut_flg) -> bus_creator/146
  outpmodule/141(VOUTP_AVMParkingmode_enum) -> bus_creator/141
  outpmodule/240(VOUTP_AmbLightColor3_enum) -> bus_creator/240
  outpmodule/1093(VOUTP_FDCVMCAPSRqEPSCtrl_flg) -> bus_creator/1093
  outpmodule/138(VOUTP_AVMparkingcancelTimeOut_flg) -> bus_creator/138
  bus_selector2/39 -> outpmodule/42(VAPM_SNSRLayout_enum)  "<VAPM_SNSRLayout_enum>"
  outpmodule/704(VOUTP_FDCTHCLEVentZSta_enum) -> bus_creator/704
  outpmodule/137(VOUTP_AVMparkingcancel_enum) -> bus_creator/137
  bus_selector3/95 -> outpmodule/273(VBCM_AmbWelENFlash_enum)  "<VBCM_AmbWelENFlash_enum>"
  outpmodule/650(VOUTP_FDCompCmd_rpm) -> bus_creator/650
  outpmodule/136(VOUTP_EPBStaTimeOut_flg) -> bus_creator/136
  outpmodule/134(VOUTP_EPBErrStaTimeOut_flg) -> bus_creator/134
  outpmodule/132(VOUTP_EPBExtApplyAvailTimeOut_flg) -> bus_creator/132
  outpmodule/126(VOUTP_ESCStandstillTimeOut_flg) -> bus_creator/126
  bus_selector12/63 -> outpmodule/888(VTPM_ID3messageALTU_raw8)  "<VTPM_ID3messageALTU_raw8>"
  bus_selector4/102 -> outpmodule/459(VDDM_Shifter1CSErrDTC_raw32)  "<VDDM_Shifter1CSErrDTC_raw32>"
  outpmodule/127(VOUTP_ESCAPSSta_enum) -> bus_creator/127
  bus_selector11/155 -> outpmodule/804(VTHC_FDCTHCCREVentYStaSet4_enum)  "<VTHC_FDCTHCCREVentYStaSet4_enum>"
  outpmodule/128(VOUTP_ESCAPSStaTimeOut_flg) -> bus_creator/128
  outpmodule/125(VOUTP_ESCStandstill_flg) -> bus_creator/125
  bus_selector12/45 -> outpmodule/870(VTPM_S4ID_raw32)  "<VTPM_S4ID_raw32>"
  outpmodule/123(VOUTP_BrkSwV_flg) -> bus_creator/123
  bus_selector4/150 -> outpmodule/507(VDDM_CAN1BusErrorDTC_raw32)  "<VDDM_CAN1BusErrorDTC_raw32>"
  outpmodule/122(VOUTP_BrkSwStaTimeOut_flg) -> bus_creator/122
  outpmodule/867(VOUTP_S1ID_raw32) -> bus_creator/867
  bus_selector9/6 -> outpmodule/564(VPMM_DCDCEnaReq_flg)  "<VPMM_DCDCEnaReq_flg>"
  outpmodule/121(VOUTP_BrkSwSta_flg) -> bus_creator/121
  outpmodule/120(VOUTP_MCPressureVTimeOut_flg) -> bus_creator/120
  bus_selector4/153 -> outpmodule/510(VDDM_CAN4BusErrorDTC_raw32)  "<VDDM_CAN4BusErrorDTC_raw32>"
  outpmodule/598(VOUTP_CtrlFrEDUINVERTER_flg) -> bus_creator/598
  outpmodule/114(VOUTP_YawRateVTimeOut_flg) -> bus_creator/114
  outpmodule/929(VOUTP_ShiftGearPosn_enum) -> bus_creator/929
  outpmodule/185(VOUTP_HoodSW_flg) -> bus_creator/185
  outpmodule/885(VOUTP_S4WheelDebugALTU_pct) -> bus_creator/885
  bus_selector9/25 -> outpmodule/583(VPMM_EvccAplusPwrUpReq_flg)  "<VPMM_EvccAplusPwrUpReq_flg>"
  outpmodule/111(VOUTP_MCPressure_bar) -> bus_creator/111
  outpmodule/573(VOUTP_RrMCUEnaReq_flg) -> bus_creator/573
  outpmodule/279(VOUTP_AmbColorSta2_enum) -> bus_creator/279
  bus_selector13/17 -> outpmodule/939(VTQD_FrEDURolRgnTq_Nm)  "<VTQD_FrEDURolRgnTq_Nm>"
  outpmodule/108(VOUTP_LatAccelTimeOut_flg) -> bus_creator/108
  bus_selector10/16 -> outpmodule/622(VSYS_Country2_cnt)  "<VSYS_Country2_cnt>"
  outpmodule/104(VOUTP_GRADETimeOut_flg) -> bus_creator/104
  bus_selector4/75 -> outpmodule/432(VDDM_RLRUSSDTC_raw32)  "<VDDM_RLRUSSDTC_raw32>"
  outpmodule/102(VOUTP_SASVTimeOut_flg) -> bus_creator/102
  outpmodule/103(VOUTP_GRADE_Deg) -> bus_creator/103
  outpmodule/471(VOUTP_RRBatwarnDTC_raw32) -> bus_creator/471
  outpmodule/238(VOUTP_AmbLightColor1_enum) -> bus_creator/238
  bus_selector11/149 -> outpmodule/798(VTHC_FDCTHCREVentYStaSet4_enum)  "<VTHC_FDCTHCREVentYStaSet4_enum>"
  outpmodule/100(VOUTP_SASCALTimeOut_flg) -> bus_creator/100
  outpmodule/97(VOUTP_SASSpeedValid_flg) -> bus_creator/97
  outpmodule/605(VOUTP_OTAPwrReqStdChkSta_enum) -> bus_creator/605
  outpmodule/838(VOUTP_LFSensorFail_flg) -> bus_creator/838
  bus_selector4/121 -> outpmodule/478(VDDM_LRWheelTmpHighDTC_raw32)  "<VDDM_LRWheelTmpHighDTC_raw32>"
  outpmodule/93(VOUTP_SASAngle_Deg) -> bus_creator/93
  bus_selector12/80 -> outpmodule/905(VTPM_WriteChkfinLRID_raw)  "<VTPM_WriteChkfinLRID_raw>"
  outpmodule/92(VOUTP_EPSAOIControlTimeOut_flg) -> bus_creator/92
  bus_selector12/73 -> outpmodule/898(VTPM_RRPindi_enum)  "<VTPM_RRPindi_enum>"
  bus_selector9/10 -> outpmodule/568(VPMM_PowerSta_enum)  "<VPMM_PowerSta_enum>"
  bus_selector4/55 -> outpmodule/412(VDDM_ESC7NoComDTC_raw32)  "<VDDM_ESC7NoComDTC_raw32>"
  outpmodule/91(VOUTP_EPSAOIControl_enum) -> bus_creator/91
  bus_selector2/15 -> outpmodule/18(VAPM_APSDRLL_cm)  "<VAPM_APSDRLL_cm>"
  bus_selector4/8 -> outpmodule/365(VDDM_C3CCU1CSDTC_raw32)  "<VDDM_C3CCU1CSDTC_raw32>"
  bus_selector16/28 -> outpmodule/1010(VVMC_ADASLKASta_enum)  "<VVMC_ADASLKASta_enum>"
  bus_selector3/83 -> outpmodule/261(VBCM_AmbWelEN_flg)  "<VBCM_AmbWelEN_flg>"
  bus_selector16/26 -> outpmodule/1008(VVMC_ActACCRequiredAccel_mps2)  "<VVMC_ActACCRequiredAccel_mps2>"
  bus_selector16/27 -> outpmodule/1009(VVMC_LateralCtrl_flg)  "<VVMC_LateralCtrl_flg>"
  bus_selector2/12 -> outpmodule/15(VAPM_PASDFCR_cm)  "<VAPM_PASDFCR_cm>"
  bus_selector16/23 -> outpmodule/1005(VVMC_ACCRequiredAccel_mps2)  "<VVMC_ACCRequiredAccel_mps2>"
  outpmodule/110(VOUTP_LongAccelTimeOut_flg) -> bus_creator/110
  bus_selector3/40 -> outpmodule/218(VBCM_RoomLampL_flg)  "<VBCM_RoomLampL_flg>"
  outpmodule/233(VOUTP_AmbLightBrightness2_enum) -> bus_creator/233
  bus_selector16/25 -> outpmodule/1007(VVMC_FeatArbitrFinal_enum)  "<VVMC_FeatArbitrFinal_enum>"
  bus_selector16/21 -> outpmodule/1003(VVMC_ISODecLimit_mps2)  "<VVMC_ISODecLimit_mps2>"
  outpmodule/452(VOUTP_MSAMalfuncDetDTC_raw32) -> bus_creator/452
  bus_selector12/83 -> outpmodule/908(VTPM_Flashdatavalid_enum)  "<VTPM_Flashdatavalid_enum>"
  bus_selector16/20 -> outpmodule/1002(VVMC_ISOAccLimit_mps2)  "<VVMC_ISOAccLimit_mps2>"
  outpmodule/218(VOUTP_RoomLampL_flg) -> bus_creator/218
  bus_selector9/24 -> outpmodule/582(VPMM_ReVehThdChkSta_enum)  "<VPMM_ReVehThdChkSta_enum>"
  outpmodule/896(VOUTP_RFPind_enum) -> bus_creator/896
  bus_selector16/19 -> outpmodule/1001(VVMC_AccCalcuPID_mps2)  "<VVMC_AccCalcuPID_mps2>"
  bus_selector2/58 -> outpmodule/61(VAPM_RRRawWhlSpeedV_flg)  "<VAPM_RRRawWhlSpeedV_flg>"
  bus_selector16/18 -> outpmodule/1000(VVMC_SPD2ACCAct_flg)  "<VVMC_SPD2ACCAct_flg>"
  bus_selector2/151 -> outpmodule/154(VAPM_TCSActiveTimeOut_flg)  "<VAPM_TCSActiveTimeOut_flg>"
  outpmodule/446(VOUTP_FrMCUSigErrDetDTC_raw32) -> bus_creator/446
  bus_selector4/59 -> outpmodule/416(VDDM_DiagHCrashDTC_raw32)  "<VDDM_DiagHCrashDTC_raw32>"
  outpmodule/245(VOUTP_SPTGDet_flg) -> bus_creator/245
  bus_selector16/14 -> outpmodule/996(VVMC_RearWhlSlipRatioCtrl_flg)  "<VVMC_RearWhlSlipRatioCtrl_flg>"
  outpmodule/922(VOUTP_ModelVersionChksum_raw) -> bus_creator/922
  outpmodule/865(VOUTP_LRSensorMode_flg) -> bus_creator/865
  bus_selector16/13 -> outpmodule/995(VVMC_FrontRearSlipRatioCtrl_flg)  "<VVMC_FrontRearSlipRatioCtrl_flg>"
  bus_selector16/9 -> outpmodule/991(VVMC_FeatArbitrSta_enum)  "<VVMC_FeatArbitrSta_enum>"
  bus_selector4/42 -> outpmodule/399(VDDM_RLDoorSWDTC_raw32)  "<VDDM_RLDoorSWDTC_raw32>"
  outpmodule/408(VOUTP_APSCorrErrDTC_raw32) -> bus_creator/408
  outpmodule/625(VOUTP_Change1_cnt) -> bus_creator/625
  outpmodule/324(VOUTP_PTGUserHeight7_cnt) -> bus_creator/324
  bus_selector16/10 -> outpmodule/992(VVMC_FeatReqSpd_kph)  "<VVMC_FeatReqSpd_kph>"
  outpmodule/828(VOUTP_LRBatWarn_flg) -> bus_creator/828
  bus_selector16/5 -> outpmodule/987(VVMC_VMCAEBCtrlAvail_flg)  "<VVMC_VMCAEBCtrlAvail_flg>"
  bus_selector16/3 -> outpmodule/985(VVMC_VehicleSpeed_kph)  "<VVMC_VehicleSpeed_kph>"
  bus_selector16/2 -> outpmodule/984(VVMC_VehicleSpeed_mph)  "<VVMC_VehicleSpeed_mph>"
  bus_selector16/1 -> outpmodule/983(VVMC_FeatSetSpdFinal_raw32)  "<VVMC_FeatSetSpdFinal_raw32>"
  outpmodule/997(VOUTP_SingleWhlSlipRatioCtrl_flg) -> bus_creator/997
  BTHC_outputs/1 -> bus_selector11/1
  BV2L_outputs/1 -> bus_selector15/1
  bus_selector15/5 -> outpmodule/980(VV2L_ReqOBCIntrV2LEna_enum)  "<VV2L_ReqOBCIntrV2LEna_enum>"
  bus_selector15/6 -> outpmodule/981(VV2L_HVPO120VGrpALDSt_enum)  "<VV2L_HVPO120VGrpALDSt_enum>"
  outpmodule/129(VOUTP_EPBExtReleaseAvail_flg) -> bus_creator/129
  bus_selector2/114 -> outpmodule/117(VAPM_LongAccelV_flg)  "<VAPM_LongAccelV_flg>"
  bus_selector4/92 -> outpmodule/449(VDDM_ACCAccelCmdErrDetDTC_raw32)  "<VDDM_ACCAccelCmdErrDetDTC_raw32>"
  outpmodule/1053(VOUTP_ADASLFCHandsOffWarning_enum) -> bus_creator/1053
  bus_selector15/3 -> outpmodule/978(VV2L_ReqV2LIVIDisChrg_enum)  "<VV2L_ReqV2LIVIDisChrg_enum>"
  outpmodule/106(VOUTP_YawRateTimeOut_flg) -> bus_creator/106
  outpmodule/181(VOUTP_HornCtrl_flg) -> bus_creator/181
  bus_selector2/44 -> outpmodule/47(VAPM_LFRawWhlSpeed_kph)  "<VAPM_LFRawWhlSpeed_kph>"
  bus_selector12/33 -> outpmodule/858(VTPM_LRWheelPSW_raw8)  "<VTPM_LRWheelPSW_raw8>"
  outpmodule/983(VOUTP_FeatSetSpdFinal_raw32) -> bus_creator/983
  BTQR_outputs/1 -> bus_selector14/1
  outpmodule/320(VOUTP_PTGUserHeight2_cnt) -> bus_creator/320
  bus_selector16/8 -> outpmodule/990(VVMC_VMCMSACtrlAvail_flg)  "<VVMC_VMCMSACtrlAvail_flg>"
  BTQD_outputs/1 -> bus_selector13/1
  outpmodule/325(VOUTP_PTGOpenHeight12_enum) -> bus_creator/325
  outpmodule/1043(VOUTP_ADASSLIFSpdLim_enum) -> bus_creator/1043
  outpmodule/150(VOUTP_IVIScreenTimeOut_flg) -> bus_creator/150
  bus_selector16/30 -> outpmodule/1012(VVMC_LKATOIFault_flg)  "<VVMC_LKATOIFault_flg>"
  bus_selector10/12 -> outpmodule/618(VSYS_Minor2_cnt)  "<VSYS_Minor2_cnt>"
  BBCM_outputs/1 -> bus_selector3/1
  outpmodule/508(VOUTP_CAN2BusErrorDTC_raw32) -> bus_creator/508
  outpmodule/78(VOUTP_RRPulseCountVTimeOut_flg) -> bus_creator/78
  outpmodule/83(VOUTP_LRPulseCount_enum) -> bus_creator/83
  bus_selector3/178 -> outpmodule/356(VBCM_WinLROpenedSta_pct)  "<VBCM_WinLROpenedSta_pct>"
  bus_selector3/27 -> outpmodule/205(VBCM_ReverseLamp_flg)  "<VBCM_ReverseLamp_flg>"
  bus_selector3/176 -> outpmodule/354(VBCM_WinLFOpenedSta_pct)  "<VBCM_WinLFOpenedSta_pct>"
  bus_selector6/9 -> outpmodule/533(VDKC_PCommandToBCM_enum)  "<VDKC_PCommandToBCM_enum>"
  bus_selector3/100 -> outpmodule/278(VBCM_AmbColorSta1_enum)  "<VBCM_AmbColorSta1_enum>"
  outpmodule/119(VOUTP_MCPressureV_bar) -> bus_creator/119
  bus_selector16/11 -> outpmodule/993(VVMC_JerkPCT_pct)  "<VVMC_JerkPCT_pct>"
  bus_selector10/24 -> outpmodule/630(VSYS_SHA3_cnt)  "<VSYS_SHA3_cnt>"
